simulink model "MATLAB_TEST"  (R2019b)
settings: Solver=FixedStepDiscrete  StartTime=0  StopTime=50  FixedStep=0.0025  RelTol=1e-3
undefined symbols (not defined in the file): BCM_COM_PROC_P20, BCM_COM_PROC_P20_SFW_R2018b, BCM_COM_PROC_P2_5, BCM_COM_PROC_P2_5_SFW_R2018b, BCM_COM_PROC_P5, BCM_COM_PROC_P5_SFW_R2018b, BCMA_ACCU_PT_Conf_Flt, BCMA_ACCU_PT_Unconf_Flt, BCMA_Antiskid_Off_Sanction, BCMA_Avionics_Conf_Flt, BCMA_BCM_CCDL_Conf_Flt, BCMA_BCM_CCDL_Unconf_Flt, BCMA_BCM_DBCU_INHIBITION_Conf_Flt, BCMA_BCM_DBCU_INHIBITION_Unconf_Flt, BCMA_BCP_ALT_Disp_Sw_Conf_Flt, BCMA_BCP_ALT_Disp_Sw_Unconf_Flt, BCMA_BCP_ALT_SW_ON_CMD_Conf_Flt, BCMA_BCP_ALT_SW_ON_CMD_Unconf_Flt, BCMA_BCP_PARK_OFF_SW_CMD_Conf_Flt, BCMA_BCP_PARK_OFF_SW_CMD_Unconf_Flt, BCMA_CF_BSELV_JCL, BCMA_CF_BSELV_JOP, BCMA_CF_BSELV_OC, BCMA_CF_BSELV_SC, BCMA_CF_LH_SV_JCL, BCMA_CF_LH_SV_JOP, BCMA_CF_LH_SV_OC, BCMA_CF_LH_SV_SC, BCMA_CF_PARK_BRK, BCMA_CF_RESIDUAL_PRESS, BCMA_CF_RH_SV_JCL, BCMA_CF_RH_SV_JOP, BCMA_CF_RH_SV_OC, BCMA_CF_RH_SV_SC, BCMA_CF_SELV_JCL, BCMA_CF_SELV_JOP, BCMA_CF_SELV_OC, BCMA_CF_SELV_SC, BCMA_CF_SV_DRIFT, BCMA_DBCU_ALT_MODE_Conf_Flt, BCMA_DBCU_ALT_MODE_Unconf_Flt, BCMA_DBCU_BRK_ORDER_FAIL_Conf_Flt, BCMA_DBCU_BRK_ORDER_FAIL_Unconf_Flt, BCMA_DBCU_Conf_Flt, BCMA_DBCU_DISPATCH_SW_ON_Conf_Flt, BCMA_DBCU_DISPATCH_SW_ON_Unconf_Flt, BCMA_DBCU_FAILED_Conf_Flt, BCMA_DBCU_FAILED_Unconf_Flt, BCMA_DFCS1_Capsule_Validity, BCMA_DFCS1_Label202_Corrupted, BCMA_DFCS1_Label202_Not_Refreshed, BCMA_DFCS1_Label204_Corrupted, BCMA_DFCS1_Label204_Not_Refreshed, BCMA_DFCS1_Label205_Corrupted, BCMA_DFCS1_Label205_Not_Refreshed, BCMA_DFCS1_Label206_Corrupted, BCMA_DFCS1_Label206_Not_Refreshed, BCMA_DFCS1_Label207_Corrupted, BCMA_DFCS1_Label207_Not_Refreshed, BCMA_DFCS3_Capsule_Validity ... (+762)
libraries: simulink x73, lib_MBD_Control x5
(part 10 of 16)

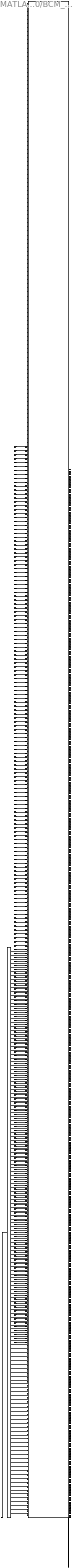
== system MATLAB_TEST/AVIONICS/Brake_Control_Module_Side_A/BCSA Controller CP/BCM_COM_PROC_P20/BCM_COM_PROC_P20 ==
  V_BCM_COM_Tacho_Conf_Flt_W12 : Inport
  V_BCM_COM_Tacho_Conf_Flt_W34 : Inport  Port=2
  V_BCM_COM_DFCS_A_Gnd_Spd_Acq : Inport  Port=3
  V_BCM_COM_DFCS_B_Gnd_Spd_Acq : Inport  Port=4
  V_BCM_COM_DFCS_A_Long_Accel_Acq : Inport  Port=5
  V_BCM_COM_DFCS_B_Long_Accel_Acq : Inport  Port=6
  V_BCM_COM_DFCS_A_Pitch_Ang_Acq : Inport  Port=7
  V_BCM_COM_DFCS_B_Pitch_Ang_Acq : Inport  Port=8
  V_BCM_COM_DFCS_A_LMLG_WOWs_Acq : Inport  Port=9
  V_BCM_COM_DFCS_B_LMLG_WOWs_Acq : Inport  Port=10
  V_BCM_COM_DFCS_A_RMLG_WOWs_Acq : Inport  Port=11
  V_BCM_COM_DFCS_B_RMLG_WOWs_Acq : Inport  Port=12
  V_BCM_COM_DFCS_A_NLG_WOWs_Acq : Inport  Port=13
  V_BCM_COM_DFCS_B_NLG_WOWs_Acq : Inport  Port=14
  V_BCM_COM_DFCS_A_WOWs_Val_Acq : Inport  Port=15
  V_BCM_COM_DFCS_B_WOWs_Val_Acq : Inport  Port=16
  V_BCM_COM_RH_Decel_Law_Brkg_Press_Cmd : Inport  Port=17
  V_BCM_COM_LH_Decel_Law_Brkg_Press_Cmd : Inport  Port=18
  V_BCM_COM_DFCS_A_DFCS_LH_Braking_Cmd_Acq : Inport  Port=19
  V_BCM_COM_DFCS_A_DFCS_RH_Braking_Cmd_Acq : Inport  Port=20
  V_BCM_COM_DFCS_B_DFCS_LH_Braking_Cmd_Acq : Inport  Port=21
  V_BCM_COM_DFCS_B_DFCS_RH_Braking_Cmd_Acq : Inport  Port=22
  V_BCM_COM_DFCS_A_Decel_Law_Inhib_Acq : Inport  Port=23
  V_BCM_COM_DFCS_B_Decel_Law_Inhib_Acq : Inport  Port=24
  V_BCM_COM_DFCS_A_TLA_Above_Idle_Acq : Inport  Port=25
  V_BCM_COM_DFCS_B_TLA_Above_Idle_Acq : Inport  Port=26
  V_BCM_COM_LG_Lever_Up_Acq : Inport  Port=27
  V_BCM_COM_LG_Lever_Up_Unconf_Flt : Inport  Port=28
  V_BCM_COM_LG_Lever_Up_Conf_Flt : Inport  Port=29
  V_BCM_COM_LMLG_Downlock_Acq : Inport  Port=30
  V_BCM_COM_RMLG_Downlock_Acq : Inport  Port=31
  V_BCM_COM_LMLG_Dnlk_Unconf_Flt : Inport  Port=32
  V_BCM_COM_LMLG_Dnlk_Conf_Flt : Inport  Port=33
  V_BCM_COM_RMLG_Dnlk_Unconf_Flt : Inport  Port=34
  V_BCM_COM_RMLG_Dnlk_Conf_Flt : Inport  Port=35
  V_BCM_COM_Engine_Running_Acq : Inport  Port=36
  V_BCM_COM_Maint_Itv_Function_Req : Inport  Port=37
  V_BCM_COM_BCM_Config : Inport  Port=38
  V_BCM_COM_BCM_Off_Sanction : Inport  Port=39
  V_BCM_COM_BCM_Validity_By_SP : Inport  Port=40
  V_BCM_COM_BCP_BCM_Alt_Sw_On_Cmd_Acq : Inport  Port=41
  V_BCM_COM_BCP_BCM_Alt_Sw_On_Cmd_Conf_Flt : Inport  Port=42
  V_BCM_COM_BCP_BCM_Alt_Sw_On_Cmd_Unconf_Flt : Inport  Port=43
  V_BCM_COM_MP_BCMA_Alt_Disp_Sw_Conf_Flt : Inport  Port=44
  V_BCM_COM_MP_BCMA_Alt_Disp_Sw_Unconf_Flt : Inport  Port=45
  V_BCM_COM_MP_BCMA_Alt_Disp_Sw_Acq : Inport  Port=46
  V_BCM_COM_Antiskid_Off_Sanction : Inport  Port=47
  V_BCM_COM_Norm_Brkg_Off_Sanc : Inport  Port=48
  V_BCM_COM_CF_LH_ALT_BRK_LOSS : Inport  Port=49
  V_BCM_COM_CF_DBCU_FAILED : Inport  Port=50
  V_BCM_COM_CF_RH_ALT_BRK_LOSS : Inport  Port=51
  V_BCM_COM_SV_PT_Filt : Inport  Port=52
  V_BCM_COM_PBSELV_ON_POS_Acq : Inport  Port=53
  V_BCM_COM_PBSELV_ON_POS_Unconf_Flt : Inport  Port=54
  V_BCM_COM_PBSELV_ON_POS_Conf_Flt : Inport  Port=55
  V_BCM_COM_Hyd_A_Press_Acq : Inport  Port=56
  V_BCM_COM_Hyd_B_Press_Acq : Inport  Port=57
  V_BCM_COM_Whl_AS_Inhib_Cond_W12 : Inport  Port=58
  V_BCM_COM_Whl_AS_Inhib_Cond_W34 : Inport  Port=59
  V_BCM_COM_Whl_LP_AS_Curr_Order : Inport  Port=60
  V_BCM_COM_SV_PT_Cons : Inport  Port=61
  V_BCM_COM_Wheel_Filtered_Speed_W12 : Inport  Port=62
  V_BCM_COM_Wheel_Filtered_Speed_W34 : Inport  Port=63
  V_BCM_COM_Wheel_Speed_Error_W12 : Inport  Port=64
  V_BCM_COM_Wheel_Speed_Error_W34 : Inport  Port=65
  V_BCM_COM_Whl_LP_AS_Curr_Order_W12 : Inport  Port=66
  V_BCM_COM_Whl_LP_AS_Curr_Order_W34 : Inport  Port=67
  V_BCM_COM_SV_Current : Inport  Port=68
  V_BCM_COM_SV_PT_Cons_Val : Inport  Port=69
  V_BCM_COM_BCM_CCDL_Conf_Flt : Inport  Port=70
  V_BCM_COM_BCM_CCDL_Unconf_Flt : Inport  Port=71
  V_BCM_COM_Adhesion_In_Acq_W12 : Inport  Port=72
  V_BCM_COM_Adhesion_In_Acq_W34 : Inport  Port=73
  V_BCM_COM_Opt_Adhesion_In_Acq_W12 : Inport  Port=74
  V_BCM_COM_Opt_Adhesion_In_Acq_W34 : Inport  Port=75
  V_BCM_COM_Target_Speed_In_Acq_W12 : Inport  Port=76
  V_BCM_COM_Target_Speed_In_Acq_W34 : Inport  Port=77
  V_BCM_COM_Big_Slip_WD_Trig_In_Acq_W12 : Inport  Port=78
  V_BCM_COM_Big_Slip_WD_Trig_In_Acq_W34 : Inport  Port=79
  V_BCM_COM_Big_Gamma_Trig_In_Acq_W12 : Inport  Port=80
  V_BCM_COM_Big_Gamma_Trig_In_Acq_W34 : Inport  Port=81
  V_BCM_COM_Small_Slip_Trig_In_Acq_W12 : Inport  Port=82
  V_BCM_COM_Small_Slip_Trig_In_Acq_W34 : Inport  Port=83
  V_BCM_COM_Big_Slip_Trig_In_Acq_W12 : Inport  Port=84
  V_BCM_COM_Big_Slip_Trig_In_Acq_W34 : Inport  Port=85
  V_BCM_COM_BCM_DBCU_INHIBITION_Conf_Flt : Inport  Port=86
  V_BCM_COM_BCM_DBCU_INHIBITION_Unconf_Flt : Inport  Port=87
  V_BCM_COM_BCM_DBCU_INHIBITION_Acq : Inport  Port=88
  V_BCM_COM_Engine_1_Running_Acq_Val : Inport  Port=89
  V_BCM_COM_Engine_2_Running_Acq_Val : Inport  Port=90
  V_BCM_COM_Hyd_A_Press_Acq_Val : Inport  Port=91
  V_BCM_COM_Hyd_B_Press_Acq_Val : Inport  Port=92
  V_BCM_COM_DFCS_A_Gnd_Spd_Acq_Val : Inport  Port=93
  V_BCM_COM_DFCS_A_Long_Accel_Acq_Val : Inport  Port=94
  V_BCM_COM_DFCS_A_Pitch_Angle_Acq_Val : Inport  Port=95
  V_BCM_COM_DFCS_A_Decel_Law_Inhib_Acq_Val : Inport  Port=96
  V_BCM_COM_DFCS_B_Decel_Law_Inhib_Acq_Val : Inport  Port=97
  V_BCM_COM_DFCS_B_Gnd_Spd_Acq_Val : Inport  Port=98
  V_BCM_COM_DFCS_B_Long_Accel_Acq_Val : Inport  Port=99
  V_BCM_COM_DFCS_B_Pitch_Angle_Acq_Val : Inport  Port=100
  V_BCM_COM_DFCS_A_Lmlg_Wow_1_Acq_Val : Inport  Port=101
  V_BCM_COM_DFCS_A_Lmlg_Wow_2_Acq_Val : Inport  Port=102
  V_BCM_COM_DFCS_A_Lmlg_Wow_3_Acq_Val : Inport  Port=103
  V_BCM_COM_DFCS_A_Rmlg_Wow_1_Acq_Val : Inport  Port=104
  V_BCM_COM_DFCS_A_Rmlg_Wow_2_Acq_Val : Inport  Port=105
  V_BCM_COM_DFCS_A_Rmlg_Wow_3_Acq_Val : Inport  Port=106
  V_BCM_COM_DFCS_A_Nlg_Wow_1_Acq_Val : Inport  Port=107
  V_BCM_COM_DFCS_A_Nlg_Wow_2_Acq_Val : Inport  Port=108
  V_BCM_COM_DFCS_A_Nlg_Wow_3_Acq_Val : Inport  Port=109
  V_BCM_COM_DFCS_A_Wow_Val_1_Acq_Val : Inport  Port=110
  V_BCM_COM_DFCS_A_Wow_Val_2_Acq_Val : Inport  Port=111
  V_BCM_COM_DFCS_A_Wow_Val_3_Acq_Val : Inport  Port=112
  V_BCM_COM_DFCS_B_Lmlg_Wow_1_Acq_Val : Inport  Port=113
  V_BCM_COM_DFCS_B_Lmlg_Wow_2_Acq_Val : Inport  Port=114
  V_BCM_COM_DFCS_B_Lmlg_Wow_3_Acq_Val : Inport  Port=115
  V_BCM_COM_DFCS_B_Rmlg_Wow_1_Acq_Val : Inport  Port=116
  V_BCM_COM_DFCS_B_Rmlg_Wow_2_Acq_Val : Inport  Port=117
  V_BCM_COM_DFCS_B_Rmlg_Wow_3_Acq_Val : Inport  Port=118
  V_BCM_COM_DFCS_B_Nlg_Wow_1_Acq_Val : Inport  Port=119
  V_BCM_COM_DFCS_B_Nlg_Wow_2_Acq_Val : Inport  Port=120
  V_BCM_COM_DFCS_B_Nlg_Wow_3_Acq_Val : Inport  Port=121
  V_BCM_COM_DFCS_B_Wow_Val_1_Acq_Val : Inport  Port=122
  V_BCM_COM_DFCS_B_Wow_Val_2_Acq_Val : Inport  Port=123
  V_BCM_COM_DFCS_B_Wow_Val_3_Acq_Val : Inport  Port=124
  V_BCM_COM_DFCS_B_DFCS_RH_Brkg_Cmd_Acq_Val : Inport  Port=125
  V_BCM_COM_DFCS_B_DFCS_LH_Brkg_Cmd_Acq_Val : Inport  Port=126
  V_BCM_COM_DFCS_A_DFCS_RH_Brkg_Cmd_Acq_Val : Inport  Port=127
  V_BCM_COM_DFCS_A_DFCS_LH_Brkg_Cmd_Acq_Val : Inport  Port=128
  V_BCM_COM_DFCS_A_DBCU_ALT_Mode_1_Acq_Val : Inport  Port=129
  V_BCM_COM_DFCS_A_DBCU_ALT_Mode_2_Acq_Val : Inport  Port=130
  V_BCM_COM_DFCS_B_DBCU_ALT_Mode_1_Acq_Val : Inport  Port=131
  V_BCM_COM_DFCS_B_DBCU_ALT_Mode_2_Acq_Val : Inport  Port=132
  V_BCM_COM_DFCS_A_TLA_Above_Idle_Acq_Val : Inport  Port=133
  V_BCM_COM_DFCS_B_TLA_Above_Idle_Acq_Val : Inport  Port=134
  V_BCM_COM_UTC_Time_Hours_Acq : Inport  Port=135
  V_BCM_COM_UTC_Time_Hours_Conf_Flt : Inport  Port=136
  V_BCM_COM_UTC_Time_Hours_Unconf_Flt : Inport  Port=137
  V_BCM_COM_UTC_Time_Minutes_Acq : Inport  Port=138
  V_BCM_COM_UTC_Time_Minutes_Conf_Flt : Inport  Port=139
  V_BCM_COM_UTC_Time_Minutes_Unconf_Flt : Inport  Port=140
  V_BCM_COM_UTC_Time_Seconds_Acq : Inport  Port=141
  V_BCM_COM_UTC_Time_Seconds_Conf_Flt : Inport  Port=142
  V_BCM_COM_UTC_Time_Seconds_Unconf_Flt : Inport  Port=143
  V_BCM_COM_DBCU_BRK_ORDER_FAIL_Acq : Inport  Port=144
  V_BCM_COM_DBCU_DISPATCH_SW_ON_Acq : Inport  Port=145
  V_BCM_COM_LH_DBCU_BRK_CMD_FDBK_Acq : Inport  Port=146
  V_BCM_COM_RH_DBCU_BRK_CMD_FDBK_Acq : Inport  Port=147
  V_BCM_COM_DBCU_FAILED_Acq : Inport  Port=148
  V_BCM_COM_DBCU_ALT_MODE_Acq : Inport  Port=149
  V_BCM_COM_DBCU_BRK_ORDER_FAIL_Conf_Flt : Inport  Port=150
  V_BCM_COM_DBCU_BRK_ORDER_FAIL_Unconf_Flt : Inport  Port=151
  V_BCM_COM_DBCU_DISPATCH_SW_ON_Conf_Flt : Inport  Port=152
  V_BCM_COM_DBCU_DISPATCH_SW_ON_Unconf_Flt : Inport  Port=153
  V_BCM_COM_LH_DBCU_BRK_CMD_FDBK_Conf_Flt : Inport  Port=154
  V_BCM_COM_LH_DBCU_BRK_CMD_FDBK_Unconf_Flt : Inport  Port=155
  V_BCM_COM_RH_DBCU_BRK_CMD_FDBK_Conf_Flt : Inport  Port=156
  V_BCM_COM_RH_DBCU_BRK_CMD_FDBK_Unconf_Flt : Inport  Port=157
  V_BCM_COM_DBCU_FAILED_Conf_Flt : Inport  Port=158
  V_BCM_COM_DBCU_FAILED_Unconf_Flt : Inport  Port=159
  V_BCM_COM_DBCU_ALT_MODE_Conf_Flt : Inport  Port=160
  V_BCM_COM_DBCU_ALT_MODE_Unconf_Flt : Inport  Port=161
  V_BCM_COM_ACCU_PT_Conf_Flt : Inport  Port=162
  V_BCM_COM_ACCU_PT_Unconf_Flt : Inport  Port=163
  V_BCM_COM_ACCU_PT_Acq : Inport  Port=164
  V_BCM_COM_LH_BTS_Conf_Flt : Inport  Port=165
  V_BCM_COM_LH_BTS_Unconf_Flt : Inport  Port=166
  V_BCM_COM_RH_BTS_Conf_Flt : Inport  Port=167
  V_BCM_COM_RH_BTS_Unconf_Flt : Inport  Port=168
  V_BCM_COM_BCP_PARK_OFF_SW_CMD_Acq : Inport  Port=169
  V_BCM_COM_BCP_PARK_OFF_SW_CMD_Conf_Flt : Inport  Port=170
  V_BCM_COM_BCP_PARK_OFF_SW_CMD_Unconf_Flt : Inport  Port=171
  V_BCM_COM_MP_MAINT_MODE_CMD_28V_Acq : Inport  Port=172
  V_BCM_COM_MP_MAINT_MODE_CMD_GND_Acq : Inport  Port=173
  V_BCM_COM_LNLG_Tire_Press_Acq : Inport  Port=174
  V_BCM_COM_LNLG_Tire_Press_Conf_Flt : Inport  Port=175
  V_BCM_COM_LNLG_Tire_Press_Unconf_Flt : Inport  Port=176
  V_BCM_COM_RNLG_Tire_Press_Acq : Inport  Port=177
  V_BCM_COM_RNLG_Tire_Press_Conf_Flt : Inport  Port=178
  V_BCM_COM_RNLG_Tire_Press_Unconf_Flt : Inport  Port=179
  V_BCM_COM_LMLG_Outboard_Tire_Press_Acq : Inport  Port=180
  V_BCM_COM_LMLG_Outboard_Tire_Press_Conf_Flt : Inport  Port=181
  V_BCM_COM_LMLG_Outboard_Tire_Press_Unconf_Flt : Inport  Port=182
  V_BCM_COM_LMLG_Inboard_Tire_Press_Acq : Inport  Port=183
  V_BCM_COM_LMLG_Inboard_Tire_Press_Conf_Flt : Inport  Port=184
  V_BCM_COM_LMLG_Inboard_Tire_Press_Unconf_Flt : Inport  Port=185
  V_BCM_COM_RMLG_Inboard_Tire_Press_Acq : Inport  Port=186
  V_BCM_COM_RMLG_Inboard_Tire_Press_Conf_Flt : Inport  Port=187
  V_BCM_COM_RMLG_Inboard_Tire_Press_Unconf_Flt : Inport  Port=188
  V_BCM_COM_RMLG_Outboard_Tire_Press_Acq : Inport  Port=189
  V_BCM_COM_RMLG_Outboard_Tire_Press_Conf_Flt : Inport  Port=190
  V_BCM_COM_RMLG_Outboard_Tire_Press_Unconf_Flt : Inport  Port=191
  V_BCM_COM_Whl_AS_Curr_Order : Inport  Port=192
  V_BCM_COM_SV_Current_Readback : Inport  Port=193
  V_BCM_COM_Whl_AS_Activity : Inport  Port=194
  V_BCM_COM_SELV_High_Side_Readback_Val : Inport  Port=195
  V_BCM_COM_SELV_High_Side_Readback : Inport  Port=196
  V_BCM_COM_CF_LH_SV_SC : Inport  Port=197
  V_BCM_COM_CF_LH_SV_OC : Inport  Port=198
  V_BCM_COM_CF_RH_SV_SC : Inport  Port=199
  V_BCM_COM_CF_RH_SV_OC : Inport  Port=200
  V_BCM_COM_CF_SELV_SC : Inport  Port=201
  V_BCM_COM_CF_SELV_OC : Inport  Port=202
  V_BCM_COM_CF_SELV_JOP : Inport  Port=203
  V_BCM_COM_CF_SELV_JCL : Inport  Port=204
  V_BCM_COM_CF_PARK_BRK : Inport  Port=205
  V_BCM_COM_CF_RESIDUAL_PRESS : Inport  Port=206
  V_BCM_COM_Avionics_Conf_Flt : Inport  Port=207
  V_BCM_COM_DFCS_A_Conf_Flt : Inport  Port=208
  V_BCM_COM_DFCS_A_DFCS_BCM_Caps_Val : Inport  Port=209
  V_BCM_COM_DFCS_B_Conf_Flt : Inport  Port=210
  V_BCM_COM_DFCS_B_DFCS_BCM_Caps_Val : Inport  Port=211
  V_BCM_COM_PPRG_i_Acquired : Inport  Port=212
  V_BCM_COM_PPRG_Fault : Inport  Port=213
  V_BCM_COM_DBCU_Conf_Flt : Inport  Port=214
  V_BCM_COM_SV_Current_Readback_Val : Inport  Port=215
  V_BCM_COM_SV_Current_Order : Inport  Port=216
  V_BCM_COM_CF_BSELV_OC : Inport  Port=217
  V_BCM_COM_CF_BSELV_SC : Inport  Port=218
  V_BCM_COM_CF_BSELV_JCL : Inport  Port=219
  V_BCM_COM_CF_BSELV_JOP : Inport  Port=220
  V_BCM_COM_LH_SV_PT_Conf_Flt : Inport  Port=221
  V_BCM_COM_CF_SV_DRIFT : Inport  Port=222
  V_BCM_COM_CF_LH_SV_JCL : Inport  Port=223
  V_BCM_COM_CF_LH_SV_JOP : Inport  Port=224
  V_BCM_COM_RH_SV_PT_Conf_Flt : Inport  Port=225
  V_BCM_COM_CF_RH_SV_JCL : Inport  Port=226
  V_BCM_COM_CF_RH_SV_JOP : Inport  Port=227
  V_BCM_COM_LH_BTS_TEMP_Comp : Inport  Port=228
  V_BCM_COM_RH_BTS_TEMP_Comp : Inport  Port=229
  BCM_Tuning : Inport  Port=230
  BCM_COM_PROC_P20 : S-Function  FunctionName=BCM_COM_PROC_P20_SFCT  SFunctionModules=<binary blob, 18839 chars, not shown>  SFunctionDeploymentMode=off  EnableBusSupport=off
  DTC{1..2,9..16,23..36,39..51,53..55,58..59,69..71,78..134,136..137,139..140,142..163,165..173,175..176,178..179,181..182,184..185,187..188,190..191,194..215,217..227} (182 alike) : DataTypeConversion  OutDataTypeStr=boolean  SaturateOnIntegerOverflow=on  RndMeth=Zero
  DTC{37..38,135,138,141} (5 alike) : DataTypeConversion  OutDataTypeStr=int32  SaturateOnIntegerOverflow=on  RndMeth=Zero
  DTC{3..8,17..22,52,56..57,60..68,72..77,164,174,177,180,183,186,189,192..193,216,228..229} (42 alike) : DataTypeConversion  OutDataTypeStr=single  SaturateOnIntegerOverflow=on  RndMeth=Zero
  PRB_BrakeFilled : Terminator
  PRB_BrakeFilled (1) : Terminator
  PRB_GroundStopFastCond : Terminator
  PRB_GroundStopSlowCond : Terminator
  PRB_RateLimitation : Terminator
  PRB_RateLimitation (1) : Terminator
  PRB_RateLimitationActivation : Terminator
  PRB_RateLimitationActivation (1) : Terminator
  Prb_Adhesion : Terminator
  Prb_Adhesion (1) : Terminator
  Prb_Adhesion (2) : Terminator
  Prb_Adhesion (3) : Terminator
  Prb_AdhesionOpt : Terminator
  Prb_AdhesionOpt (1) : Terminator
  Prb_AdhesionOpt (2) : Terminator
  Prb_AdhesionOpt (3) : Terminator
  Prb_AsBrkLossTargetDecel : Terminator
  Prb_AsBrkLossTargetDecel (1) : Terminator
  Prb_AsBrkLossTargetDecel (2) : Terminator
  Prb_AsBrkLossTargetDecel (3) : Terminator
  Prb_AsLowPassTheorCurrent : Terminator
  Prb_AsLowPassTheorCurrent (1) : Terminator
  Prb_AsLowPassTheorCurrent (2) : Terminator
  Prb_AsLowPassTheorCurrent (3) : Terminator
  Prb_AsLowPassTheorPressure : Terminator
  Prb_AsLowPassTheorPressure (1) : Terminator
  Prb_AsLowPassTheorPressure (2) : Terminator
  Prb_AsLowPassTheorPressure (3) : Terminator
  Prb_AutomateFilteredPressure : Terminator
  Prb_AutomateFilteredPressure (1) : Terminator
  Prb_AutomateFilteredPressure (2) : Terminator
  Prb_AutomateFilteredPressure (3) : Terminator
  Prb_AutomateSofteningFreezingCond : Terminator
  Prb_AutomateSofteningFreezingCond (1) : Terminator
  Prb_AutomateSofteningFreezingCond (2) : Terminator
  Prb_AutomateSofteningFreezingCond (3) : Terminator
  Prb_AutomateState : Terminator
  Prb_AutomateState (1) : Terminator
  Prb_AutomateState (2) : Terminator
  Prb_AutomateState (3) : Terminator
  Prb_BigGammaStepSize : Terminator
  Prb_BigGammaStepSize (1) : Terminator
  Prb_BigGammaStepSize (2) : Terminator
  Prb_BigGammaStepSize (3) : Terminator
  Prb_BigGammaThreshold : Terminator
  Prb_BigGammaThreshold (1) : Terminator
  Prb_BigGammaThreshold (2) : Terminator
  Prb_BigGammaThreshold (3) : Terminator
  Prb_BigSlipStepAuthorize : Terminator
  Prb_BigSlipStepAuthorize (1) : Terminator
  Prb_BigSlipStepAuthorize (2) : Terminator
  Prb_BigSlipStepAuthorize (3) : Terminator
  Prb_BigSlipWatchDogTargetDecel : Terminator
  Prb_BigSlipWatchDogTargetDecel (1) : Terminator
  Prb_BigSlipWatchDogTargetDecel (2) : Terminator
  Prb_BigSlipWatchDogTargetDecel (3) : Terminator
  Prb_BrakingPhaseAcceleration : Terminator
  Prb_BrakingPhaseAcceleration (1) : Terminator
  Prb_BrakingPhaseAcceleration (2) : Terminator
  Prb_BrakingPhaseAcceleration (3) : Terminator
  Prb_BrakingPhaseAcceleration (4) : Terminator
  Prb_CommandedPressureTheorCurrent : Terminator
  Prb_CommandedPressureTheorCurrent (1) : Terminator
  Prb_CommandedPressureTheorCurrent (2) : Terminator
  Prb_CommandedPressureTheorCurrent (3) : Terminator
  Prb_DecelerationDecrement : Terminator
  Prb_DecelerationDecrement (1) : Terminator
  Prb_DecelerationDecrement (2) : Terminator
  Prb_DecelerationDecrement (3) : Terminator
  Prb_DenAccuBigSlip : Terminator
  Prb_DenAccuBigSlip (1) : Terminator
  Prb_DenAccuBigSlip (2) : Terminator
  Prb_DenAccuBigSlip (3) : Terminator
  Prb_FastMonitoringCondition : Terminator
  Prb_FastMonitoringCondition (1) : Terminator
  Prb_FastMonitoringCondition (2) : Terminator
  Prb_FastMonitoringCondition (3) : Terminator
  Prb_FastStateCondition : Terminator
  Prb_FastStateCondition (1) : Terminator
  Prb_FastStateCondition (2) : Terminator
  Prb_FastStateCondition (3) : Terminator
  Prb_FastTrigCondition : Terminator
  Prb_FastTrigCondition (1) : Terminator
  Prb_FastTrigCondition (2) : Terminator
  Prb_FastTrigCondition (3) : Terminator
  Prb_ForcedBigGammaStep : Terminator
  Prb_ForcedBigGammaStep (1) : Terminator
  Prb_ForcedBigGammaStep (2) : Terminator
  Prb_ForcedBigGammaStep (3) : Terminator
  Prb_ForcedBigSlipStep : Terminator
  Prb_ForcedBigSlipStep (1) : Terminator
  Prb_ForcedBigSlipStep (2) : Terminator
  Prb_ForcedBigSlipStep (3) : Terminator
  Prb_ForcedBigSlipWatchDog : Terminator
  Prb_ForcedBigSlipWatchDog (1) : Terminator
  Prb_ForcedBigSlipWatchDog (2) : Terminator
  Prb_ForcedBigSlipWatchDog (3) : Terminator
  Prb_ForcedMonitoringAuthorized : Terminator
  Prb_ForcedMonitoringAuthorized (1) : Terminator
  Prb_ForcedMonitoringAuthorized (2) : Terminator
  Prb_ForcedMonitoringAuthorized (3) : Terminator
  Prb_ForcedSmallSlipStep : Terminator
  Prb_ForcedSmallSlipStep (1) : Terminator
  Prb_ForcedSmallSlipStep (2) : Terminator
  Prb_ForcedSmallSlipStep (3) : Terminator
  Prb_HydroplaneAccelCond : Terminator
  Prb_HydroplaneAccelCond (1) : Terminator
  Prb_HydroplaneAccelCond (2) : Terminator
  Prb_HydroplaneAccelCond (3) : Terminator
  Prb_HydroplaneAccelCond (4) : Terminator
  Prb_HydroplaneAccelProblem : Terminator
  Prb_HydroplaneAccelProblem (1) : Terminator
  Prb_HydroplaneAccelProblem (2) : Terminator
  Prb_HydroplaneAccelProblem (3) : Terminator
  Prb_HydroplaneAccelProblem (4) : Terminator
  Prb_HydroplaneAcceleration : Terminator
  Prb_HydroplaneAcceleration (1) : Terminator
  Prb_HydroplaneAcceleration (2) : Terminator
  Prb_HydroplaneAcceleration (3) : Terminator
  Prb_HydroplaneAcceleration (4) : Terminator
  Prb_HydroplaneCondition : Terminator
  Prb_HydroplaneCondition (1) : Terminator
  Prb_HydroplaneCondition (2) : Terminator
  Prb_HydroplaneCondition (3) : Terminator
  Prb_HydroplanePhaseInit : Terminator
  Prb_HydroplanePhaseInit (1) : Terminator
  Prb_HydroplanePhaseInit (2) : Terminator
  Prb_HydroplanePhaseInit (3) : Terminator
  Prb_HydroplanePhaseInit (4) : Terminator
  Prb_HydroplaneTransition : Terminator
  Prb_HydroplaneTransition (1) : Terminator
  Prb_HydroplaneTransition (2) : Terminator
  Prb_HydroplaneTransition (3) : Terminator
  Prb_HydroplaneTransition (4) : Terminator
  Prb_Hydroplane_PreviousSpeed : Terminator
  Prb_Hydroplane_PreviousSpeed (1) : Terminator
  Prb_Hydroplane_PreviousSpeed (2) : Terminator
  Prb_Hydroplane_PreviousSpeed (3) : Terminator
  Prb_LeftIsInvalid : Terminator
  Prb_LeftWheelSpeed : Terminator
  Prb_MinimalTargetDecel : Terminator
  Prb_MinimalTargetDecel (1) : Terminator
  Prb_MinimalTargetDecel (2) : Terminator
  Prb_MinimalTargetDecel (3) : Terminator
  Prb_NaturalBigGammaStep : Terminator
  Prb_NaturalBigGammaStep (1) : Terminator
  Prb_NaturalBigGammaStep (2) : Terminator
  Prb_NaturalBigGammaStep (3) : Terminator
  Prb_NaturalBigSlipStep : Terminator
  Prb_NaturalBigSlipStep (1) : Terminator
  Prb_NaturalBigSlipStep (2) : Terminator
  Prb_NaturalBigSlipStep (3) : Terminator
  Prb_NaturalBigSlipWatchDog : Terminator
  Prb_NaturalBigSlipWatchDog (1) : Terminator
  Prb_NaturalBigSlipWatchDog (2) : Terminator
  Prb_NaturalBigSlipWatchDog (3) : Terminator
  Prb_NaturalSmallSlipStep : Terminator
  Prb_NaturalSmallSlipStep (1) : Terminator
  Prb_NaturalSmallSlipStep (2) : Terminator
  Prb_NaturalSmallSlipStep (3) : Terminator
  Prb_OnGndAfterHydroAccel : Terminator
  Prb_OnGndAfterHydroAccel (1) : Terminator
  Prb_OnGndAfterHydroAccel (2) : Terminator
  Prb_OnGndAfterHydroAccel (3) : Terminator
  Prb_OnGndAfterHydroAccel (4) : Terminator
  Prb_OnGroundAfterHydroTransition : Terminator
  Prb_OnGroundAfterHydroTransition (1) : Terminator
  Prb_OnGroundAfterHydroTransition (2) : Terminator
  Prb_OnGroundAfterHydroTransition (3) : Terminator
  Prb_OnGroundAfterHydroplaneTransition : Terminator
  Prb_OptimalSpeed : Terminator
  Prb_OptimalSpeed (1) : Terminator
  Prb_OptimalSpeed (2) : Terminator
  Prb_OptimalSpeed (3) : Terminator
  Prb_PreviousSpeed : Terminator
  Prb_Previous_GlobalReferenceSpeed : Terminator
  Prb_Previous_ReferenceSpeed : Terminator
  Prb_Previous_ReferenceSpeed (1) : Terminator
  Prb_Previous_ReferenceSpeed (2) : Terminator
  Prb_Previous_ReferenceSpeed (3) : Terminator
  Prb_Previous_WheelSpeedState : Terminator
  Prb_Previous_WheelSpeedState (1) : Terminator
  Prb_Previous_WheelSpeedState (2) : Terminator
  Prb_Previous_WheelSpeedState (3) : Terminator
  Prb_Previous_WheelSpeedState (4) : Terminator
  Prb_RefSpeedLowLimit : Terminator
  Prb_RefSpeedLowLimit (1) : Terminator
  Prb_RefSpeedLowLimit (2) : Terminator
  Prb_RefSpeedLowLimit (3) : Terminator
  Prb_RefSpeedLowLimit (4) : Terminator
  Prb_RefSpeedLowLimit (5) : Terminator
  Prb_RefSpeedLowLimit (6) : Terminator
  Prb_RefSpeedLowLimit (7) : Terminator
  Prb_RefSpeedLowLimit (8) : Terminator
  Prb_ReferenceSpeedDelta : Terminator
  Prb_ReferenceSpeedDelta (1) : Terminator
  Prb_ReferenceSpeedDelta (2) : Terminator
  Prb_ReferenceSpeedDelta (3) : Terminator
  Prb_ResearchModeCondition : Terminator
  Prb_ResearchModeCondition (1) : Terminator
  Prb_ResearchModeCondition (2) : Terminator
  Prb_ResearchModeCondition (3) : Terminator
  Prb_RightIsInvalid : Terminator
  Prb_RightWheelSpeed : Terminator
  Prb_SelectedPressureOrder_i : Terminator
  Prb_SlowMonitoringCondition : Terminator
  Prb_SlowMonitoringCondition (1) : Terminator
  Prb_SlowMonitoringCondition (2) : Terminator
  Prb_SlowMonitoringCondition (3) : Terminator
  Prb_SlowStateCondition : Terminator
  Prb_SlowStateCondition (1) : Terminator
  Prb_SlowStateCondition (2) : Terminator
  Prb_SlowStateCondition (3) : Terminator
  Prb_SlowTrigCondition : Terminator
  Prb_SlowTrigCondition (1) : Terminator
  Prb_SlowTrigCondition (2) : Terminator
  Prb_SlowTrigCondition (3) : Terminator
  Prb_SoftSpeedCountOrder : Terminator
  Prb_SoftSpeedCountOrder (1) : Terminator
  Prb_SoftSpeedCountOrder (2) : Terminator
  Prb_SoftSpeedCountOrder (3) : Terminator
  Prb_SoftSpeedCounter : Terminator
  Prb_SoftSpeedCounter (1) : Terminator
  Prb_SoftSpeedCounter (2) : Terminator
  Prb_SoftSpeedCounter (3) : Terminator
  Prb_SoftSpeedMaximum : Terminator
  Prb_SoftSpeedMaximum (1) : Terminator
  Prb_SoftSpeedMaximum (2) : Terminator
  Prb_SoftSpeedMaximum (3) : Terminator
  Prb_SoftSpeedResetOrder : Terminator
  Prb_SoftSpeedResetOrder (1) : Terminator
  Prb_SoftSpeedResetOrder (2) : Terminator
  Prb_SoftSpeedResetOrder (3) : Terminator
  Prb_SofteningSpeed : Terminator
  Prb_SofteningSpeed (1) : Terminator
  Prb_SofteningSpeed (2) : Terminator
  Prb_SofteningSpeed (3) : Terminator
  Prb_SpunUpCondition : Terminator
  Prb_SpunUpCondition (1) : Terminator
  Prb_SpunUpCondition (2) : Terminator
  Prb_SpunUpCondition (3) : Terminator
  Prb_SpunUpCondition_i : Terminator
  Prb_SpunUpProtectedBrakingOrder : Terminator
  Prb_StateSignalValidityCondition : Terminator
  Prb_StateSignalValidityCondition (1) : Terminator
  Prb_StateSignalValidityCondition (2) : Terminator
  Prb_StateSignalValidityCondition (3) : Terminator
  Prb_StepSize : Terminator
  Prb_StepSize (1) : Terminator
  Prb_StepSize (2) : Terminator
  Prb_StepSize (3) : Terminator
  Prb_SvLowPassTheorCurrent : Terminator
  Prb_SvLowPassTheorCurrent (1) : Terminator
  Prb_SvLowPassTheorCurrent (2) : Terminator
  Prb_SvLowPassTheorCurrent (3) : Terminator
  Prb_TargetOverDecelInteg : Terminator
  Prb_TargetOverDecelInteg (1) : Terminator
  Prb_TargetOverDecelInteg (2) : Terminator
  Prb_TargetOverDecelInteg (3) : Terminator
  Prb_TargetSpeedDelta : Terminator
  Prb_TargetSpeedDelta (1) : Terminator
  Prb_TargetSpeedDelta (2) : Terminator
  Prb_TargetSpeedDelta (3) : Terminator
  Prb_TheorCommandedPressure : Terminator
  Prb_TheorCommandedPressure (1) : Terminator
  Prb_TheorCommandedPressure (2) : Terminator
  Prb_TheorCommandedPressure (3) : Terminator
  Prb_TransitionAntiskidBrakeLoss : Terminator
  Prb_TransitionAntiskidBrakeLoss (1) : Terminator
  Prb_TransitionAntiskidBrakeLoss (2) : Terminator
  Prb_TransitionAntiskidBrakeLoss (3) : Terminator
  Prb_TransitionBigGammaStep : Terminator
  Prb_TransitionBigGammaStep (1) : Terminator
  Prb_TransitionBigGammaStep (2) : Terminator
  Prb_TransitionBigGammaStep (3) : Terminator
  Prb_TransitionBigSlipStep : Terminator
  Prb_TransitionBigSlipStep (1) : Terminator
  Prb_TransitionBigSlipStep (2) : Terminator
  Prb_TransitionBigSlipStep (3) : Terminator
  Prb_TransitionBigSlipWatchDog : Terminator
  Prb_TransitionBigSlipWatchDog (1) : Terminator
  Prb_TransitionBigSlipWatchDog (2) : Terminator
  Prb_TransitionBigSlipWatchDog (3) : Terminator
  Prb_TransitionBrakingInit : Terminator
  Prb_TransitionBrakingInit (1) : Terminator
  Prb_TransitionBrakingInit (2) : Terminator
  Prb_TransitionBrakingInit (3) : Terminator
  Prb_TransitionGammaDecrease : Terminator
  Prb_TransitionGammaDecrease (1) : Terminator
  Prb_TransitionGammaDecrease (2) : Terminator
  Prb_TransitionGammaDecrease (3) : Terminator
  Prb_TransitionGammaIncrease : Terminator
  Prb_TransitionGammaIncrease (1) : Terminator
  Prb_TransitionGammaIncrease (2) : Terminator
  Prb_TransitionGammaIncrease (3) : Terminator
  Prb_TransitionSmallSlipStep : Terminator
  Prb_TransitionSmallSlipStep (1) : Terminator
  Prb_TransitionSmallSlipStep (2) : Terminator
  Prb_TransitionSmallSlipStep (3) : Terminator
  Prb_UncorrectedMinimaltargetDecel : Terminator
  Prb_UncorrectedMinimaltargetDecel (1) : Terminator
  Prb_UncorrectedMinimaltargetDecel (2) : Terminator
  Prb_UncorrectedMinimaltargetDecel (3) : Terminator
  Prb_UnlimitedReferenceSpeed_3 : Terminator
  Prb_UnlimitedReferenceSpeed_3 (1) : Terminator
  Prb_UnlimitedReferenceSpeed_3 (2) : Terminator
  Prb_UnlimitedReferenceSpeed_3 (3) : Terminator
  Prb_UnlimitedReferenceSpeed_4 : Terminator
  Prb_UnlimitedReferenceSpeed_4 (1) : Terminator
  Prb_UnlimitedReferenceSpeed_4 (2) : Terminator
  Prb_UnlimitedReferenceSpeed_4 (3) : Terminator
  Prb_WheelSkidSmoothAverage : Terminator
  Prb_WheelSkidSmoothAverage (1) : Terminator
  Prb_WheelSkidSmoothAverage (2) : Terminator
  Prb_WheelSkidSmoothAverage (3) : Terminator
  Prb_WheelSpeedState : Terminator
  Prb_WheelSpeedState (1) : Terminator
  Prb_WheelSpeedState (2) : Terminator
  Prb_WheelSpeedState (3) : Terminator
  Prb_WheelSpeedState (4) : Terminator
  Prb_WheelSpunUpCond : Terminator
  Subsystem : Subsystem
  v_BCM_COM_AC_Long_Accel_Filt : Terminator
  v_BCM_COM_ATB_in : Terminator
  v_BCM_COM_ATB_out : Terminator
  v_BCM_COM_All_Engines_Off : Terminator
  v_BCM_COM_Alt_FT_Reset_Cond : Terminator
  v_BCM_COM_Automate_On_W12 : Terminator
  v_BCM_COM_Automate_On_W34 : Terminator
  v_BCM_COM_Automate_WD_Frozen : Terminator
  v_BCM_COM_Braking_On_W12 : Terminator
  v_BCM_COM_Braking_On_W34 : Terminator
  v_BCM_COM_Braking_State_Norm : Terminator
  v_BCM_COM_Braking_Ste_Is_Normal : Terminator
  v_BCM_COM_Brkg_SELV_High_Side_FT_Cond : Terminator
  v_BCM_COM_CF_DFCS_A_ACCEL_RX : Terminator
  v_BCM_COM_CF_DFCS_A_DBCU_ALT_MODE_1_RX : Terminator
  v_BCM_COM_CF_DFCS_A_DBCU_ALT_MODE_2_RX : Terminator
  v_BCM_COM_CF_DFCS_A_DECEL_LAW_INHIB_RX : Terminator
  v_BCM_COM_CF_DFCS_A_GND_SPEED_RX : Terminator
  v_BCM_COM_CF_DFCS_A_LH_BRK_CMD_RX : Terminator
  v_BCM_COM_CF_DFCS_A_LMLGWOW_1_RX : Terminator
  v_BCM_COM_CF_DFCS_A_LMLGWOW_2_RX : Terminator
  v_BCM_COM_CF_DFCS_A_LMLGWOW_3_RX : Terminator
  v_BCM_COM_CF_DFCS_A_NLGWOW_1_RX : Terminator
  v_BCM_COM_CF_DFCS_A_NLGWOW_2_RX : Terminator
  v_BCM_COM_CF_DFCS_A_NLGWOW_3_RX : Terminator
  v_BCM_COM_CF_DFCS_A_PITCH_RX : Terminator
  v_BCM_COM_CF_DFCS_A_RH_BRK_CMD_RX : Terminator
  v_BCM_COM_CF_DFCS_A_RMLGWOW_1_RX : Terminator
  v_BCM_COM_CF_DFCS_A_RMLGWOW_2_RX : Terminator
  v_BCM_COM_CF_DFCS_A_RMLGWOW_3_RX : Terminator
  v_BCM_COM_CF_DFCS_A_TLA_ABOVE_IDLE_RX : Terminator
  v_BCM_COM_CF_DFCS_A_VALWOW_1_RX : Terminator
  v_BCM_COM_CF_DFCS_A_VALWOW_2_RX : Terminator
  v_BCM_COM_CF_DFCS_A_VALWOW_3_RX : Terminator
  v_BCM_COM_CF_DFCS_B_ACCEL_RX : Terminator
  v_BCM_COM_CF_DFCS_B_DBCU_ALT_MODE_1_RX : Terminator
  v_BCM_COM_CF_DFCS_B_DBCU_ALT_MODE_2_RX : Terminator
  v_BCM_COM_CF_DFCS_B_DECEL_LAW_INHIB_RX : Terminator
  v_BCM_COM_CF_DFCS_B_GND_SPEED_RX : Terminator
  v_BCM_COM_CF_DFCS_B_LH_BRK_CMD_RX : Terminator
  v_BCM_COM_CF_DFCS_B_LMLGWOW_1_RX : Terminator
  v_BCM_COM_CF_DFCS_B_LMLGWOW_2_RX : Terminator
  v_BCM_COM_CF_DFCS_B_LMLGWOW_3_RX : Terminator
  v_BCM_COM_CF_DFCS_B_NLGWOW_1_RX : Terminator
  v_BCM_COM_CF_DFCS_B_NLGWOW_2_RX : Terminator
  v_BCM_COM_CF_DFCS_B_NLGWOW_3_RX : Terminator
  v_BCM_COM_CF_DFCS_B_PITCH_RX : Terminator
  v_BCM_COM_CF_DFCS_B_RH_BRK_CMD_RX : Terminator
  v_BCM_COM_CF_DFCS_B_RMLGWOW_1_RX : Terminator
  v_BCM_COM_CF_DFCS_B_RMLGWOW_2_RX : Terminator
  v_BCM_COM_CF_DFCS_B_RMLGWOW_3_RX : Terminator
  v_BCM_COM_CF_DFCS_B_TLA_ABOVE_IDLE_RX : Terminator
  v_BCM_COM_CF_DFCS_B_VALWOW_1_RX : Terminator
  v_BCM_COM_CF_DFCS_B_VALWOW_2_RX : Terminator
  v_BCM_COM_CF_DFCS_B_VALWOW_3_RX : Terminator
  v_BCM_COM_CF_ENG_1_RUN_RX : Terminator
  v_BCM_COM_CF_ENG_2_RUN_RX : Terminator
  v_BCM_COM_CF_HYD_A_PRESS_RX : Terminator
  v_BCM_COM_CF_HYD_B_PRESS_RX : Terminator
  v_BCM_COM_Custom_Braking_Mode : Terminator
  v_BCM_COM_Custom_Brkg_Cmd : Terminator
  v_BCM_COM_ERU_in : Terminator
  v_BCM_COM_ERU_out : Terminator
  v_BCM_COM_FTB_in : Terminator
  v_BCM_COM_FTB_out : Terminator
  v_BCM_COM_Forced_Act_SELV : Terminator
  v_BCM_COM_Func_Test_Press_Cmd : Terminator
  v_BCM_COM_Hyd_Press_State : Terminator
  v_BCM_COM_LGRB_in : Terminator
  v_BCM_COM_LGRB_out : Terminator
  v_BCM_COM_MLG_Dnlk_State_Cons : Terminator
  v_BCM_COM_MLG_Downlock_State_Cond : Terminator
  v_BCM_COM_MTB_in : Terminator
  v_BCM_COM_MTB_out : Terminator
  v_BCM_COM_Norm_FT_Reset_Cond : Terminator
  v_BCM_COM_PB_in : Terminator
  v_BCM_COM_PB_out : Terminator
  v_BCM_COM_Press_Cmd_FT : Terminator
  v_BCM_COM_Press_Rate_Lim_Inhib_Cond : Terminator
  v_BCM_COM_Rate_Lim_Law : Terminator
  v_BCM_COM_Regular_Brkg_Press_Cmd : Terminator
  v_BCM_COM_Ret_Brkg_Press_Cmd : Terminator
  v_BCM_COM_SELV_FT : Terminator
  v_BCM_COM_SELV_High_Side_Cmd_Order_Prev : Terminator
  v_BCM_COM_Spun_Up_Condition_W12 : Terminator
  v_BCM_COM_Spun_Up_Condition_W34 : Terminator
  v_BCM_COM_Takeoff_Phase : Terminator
  v_BCM_COM_Touchdown_Not_Active : Terminator
  v_BCM_COM_UF_DFCS_A_ACCEL_RX : Terminator
  v_BCM_COM_UF_DFCS_A_DBCU_ALT_MODE_1_RX : Terminator
  v_BCM_COM_UF_DFCS_A_DBCU_ALT_MODE_2_RX : Terminator
  v_BCM_COM_UF_DFCS_A_DECEL_LAW_INHIB_RX : Terminator
  v_BCM_COM_UF_DFCS_A_GND_SPEED_RX : Terminator
  v_BCM_COM_UF_DFCS_A_LH_BRK_CMD_RX : Terminator
  v_BCM_COM_UF_DFCS_A_LMLGWOW_1_RX : Terminator
  v_BCM_COM_UF_DFCS_A_LMLGWOW_2_RX : Terminator
  v_BCM_COM_UF_DFCS_A_LMLGWOW_3_RX : Terminator
  v_BCM_COM_UF_DFCS_A_NLGWOW_1_RX : Terminator
  v_BCM_COM_UF_DFCS_A_NLGWOW_2_RX : Terminator
  v_BCM_COM_UF_DFCS_A_NLGWOW_3_RX : Terminator
  v_BCM_COM_UF_DFCS_A_PITCH_RX : Terminator
  v_BCM_COM_UF_DFCS_A_RH_BRK_CMD_RX : Terminator
  v_BCM_COM_UF_DFCS_A_RMLGWOW_1_RX : Terminator
  v_BCM_COM_UF_DFCS_A_RMLGWOW_2_RX : Terminator
  v_BCM_COM_UF_DFCS_A_RMLGWOW_3_RX : Terminator
  v_BCM_COM_UF_DFCS_A_TLA_ABOVE_IDLE_RX : Terminator
  v_BCM_COM_UF_DFCS_A_VALWOW_1_RX : Terminator
  v_BCM_COM_UF_DFCS_A_VALWOW_2_RX : Terminator
  v_BCM_COM_UF_DFCS_A_VALWOW_3_RX : Terminator
  v_BCM_COM_UF_DFCS_B_ACCEL_RX : Terminator
  v_BCM_COM_UF_DFCS_B_DBCU_ALT_MODE_1_RX : Terminator
  v_BCM_COM_UF_DFCS_B_DBCU_ALT_MODE_2_RX : Terminator
  v_BCM_COM_UF_DFCS_B_DECEL_LAW_INHIB_RX : Terminator
  v_BCM_COM_UF_DFCS_B_GND_SPEED_RX : Terminator
  v_BCM_COM_UF_DFCS_B_LH_BRK_CMD_RX : Terminator
  v_BCM_COM_UF_DFCS_B_LMLGWOW_1_RX : Terminator
  v_BCM_COM_UF_DFCS_B_LMLGWOW_2_RX : Terminator
  v_BCM_COM_UF_DFCS_B_LMLGWOW_3_RX : Terminator
  v_BCM_COM_UF_DFCS_B_NLGWOW_1_RX : Terminator
  v_BCM_COM_UF_DFCS_B_NLGWOW_2_RX : Terminator
  v_BCM_COM_UF_DFCS_B_NLGWOW_3_RX : Terminator
  v_BCM_COM_UF_DFCS_B_PITCH_RX : Terminator
  v_BCM_COM_UF_DFCS_B_RH_BRK_CMD_RX : Terminator
  v_BCM_COM_UF_DFCS_B_RMLGWOW_1_RX : Terminator
  v_BCM_COM_UF_DFCS_B_RMLGWOW_2_RX : Terminator
  v_BCM_COM_UF_DFCS_B_RMLGWOW_3_RX : Terminator
  v_BCM_COM_UF_DFCS_B_TLA_ABOVE_IDLE_RX : Terminator
  v_BCM_COM_UF_DFCS_B_VALWOW_1_RX : Terminator
  v_BCM_COM_UF_DFCS_B_VALWOW_2_RX : Terminator
  v_BCM_COM_UF_DFCS_B_VALWOW_3_RX : Terminator
  v_BCM_COM_UF_ENG_1_RUN_RX : Terminator
  v_BCM_COM_UF_ENG_2_RUN_RX : Terminator
  v_BCM_COM_UF_HYD_A_PRESS_RX : Terminator
  v_BCM_COM_UF_HYD_B_PRESS_RX : Terminator
  V_BCM_COM_Whl_Spun_Up_State_W12 : Outport
  V_BCM_COM_Whl_Ref_Speed_W12 : Outport  Port=2
  V_BCM_COM_Whl_Spun_Up_State_W34 : Outport  Port=3
  V_BCM_COM_Whl_Ref_Speed_W34 : Outport  Port=4
  V_BCM_COM_DFCS_A_Gnd_Spd_Conv : Outport  Port=5
  V_BCM_COM_DFCS_B_Gnd_Spd_Conv : Outport  Port=6
  V_BCM_COM_AC_Gnd_Spd_Cons : Outport  Port=7
  V_BCM_COM_AC_Gnd_Spd_Cons_Val : Outport  Port=8
  V_BCM_COM_DFCS_A_Long_Accel_Conv : Outport  Port=9
  V_BCM_COM_DFCS_B_Long_Accel_Conv : Outport  Port=10
  V_BCM_COM_AC_Long_Accel_Cons : Outport  Port=11
  V_BCM_COM_AC_Long_Accel_Cons_Val : Outport  Port=12
  V_BCM_COM_AC_Long_Accel_Filt_Corr : Outport  Port=13
  V_BCM_COM_AC_Pitch_Ang_Cons_Val : Outport  Port=14
  V_BCM_COM_AC_Pitch_Ang_Filt : Outport  Port=15
  V_BCM_COM_AC_Pitch_Ang_Cons : Outport  Port=16
  V_BCM_COM_DFCS_A_WOWs_Val_Cons : Outport  Port=17
  V_BCM_COM_DFCS_B_WOWs_Val_Cons : Outport  Port=18
  V_BCM_COM_LMLG_WOWs_Cons : Outport  Port=19
  V_BCM_COM_LMLG_WOWs_Cons_Val : Outport  Port=20
  V_BCM_COM_RMLG_WOWs_Cons : Outport  Port=21
  V_BCM_COM_RMLG_WOWs_Cons_Val : Outport  Port=22
  V_BCM_COM_NLG_WOWs_Cons : Outport  Port=23
  V_BCM_COM_NLG_WOWs_Cons_Val : Outport  Port=24
  V_BCM_COM_LMLG_On_Gnd_State : Outport  Port=25
  V_BCM_COM_RMLG_On_Gnd_State : Outport  Port=26
  V_BCM_COM_LMLG_On_Gnd_State_Val : Outport  Port=27
  V_BCM_COM_RMLG_On_Gnd_State_Val : Outport  Port=28
  V_BCM_COM_MLG_On_Gnd_State : Outport  Port=29
  V_BCM_COM_NLG_On_Gnd_State : Outport  Port=30
  V_BCM_COM_NLG_On_Gnd_State_Val : Outport  Port=31
  V_BCM_COM_NLG_On_Gnd_State_Cons : Outport  Port=32
  V_BCM_COM_LH_Braking_Cmd_Cons : Outport  Port=33
  V_BCM_COM_RH_Braking_Cmd_Cons : Outport  Port=34
  V_BCM_COM_Decel_Law_Inhib_Cons : Outport  Port=35
  V_BCM_COM_Decel_Law_Inhib_Cons_Val : Outport  Port=36
  V_BCM_COM_TLA_State_Cons : Outport  Port=37
  V_BCM_COM_TLA_State_Cons_Val : Outport  Port=38
  V_BCM_COM_LG_Lever_Up_Conf : Outport  Port=39
  V_BCM_COM_LG_Lever_State_Cons : Outport  Port=40
  V_BCM_COM_LG_Lever_Ste_Cons_Val : Outport  Port=41
  V_BCM_COM_LMLG_Downlock_Conf : Outport  Port=42
  V_BCM_COM_RMLG_Downlock_Conf : Outport  Port=43
  V_BCM_COM_LMLG_Downlock_State : Outport  Port=44
  V_BCM_COM_LMLG_Dnlk_State_Val : Outport  Port=45
  V_BCM_COM_RMLG_Downlock_State : Outport  Port=46
  V_BCM_COM_RMLG_Dnlk_State_Val : Outport  Port=47
  V_BCM_COM_SELV_High_Side_Cmd_Order : Outport  Port=48
  V_BCM_COM_SELV_Low_Speed_Logic : Outport  Port=49
  V_BCM_COM_Engine_State : Outport  Port=50
  V_BCM_COM_Engine_State_Val : Outport  Port=51
  V_BCM_COM_LH_Braking_Cmd_State : Outport  Port=52
  V_BCM_COM_RH_Braking_Cmd_State : Outport  Port=53
  V_BCM_COM_LH_Regular_Brkg_Press_Cmd : Outport  Port=54
  V_BCM_COM_RH_Regular_Brkg_Press_Cmd : Outport  Port=55
  V_BCM_COM_Wheels_Global_Spun_Up_Ste : Outport  Port=56
  V_BCM_COM_Global_Reference_Spd : Outport  Port=57
  V_BCM_COM_Global_Wheel_Spd : Outport  Port=58
  V_BCM_COM_LMLG_Global_Wheel_Spd : Outport  Port=59
  V_BCM_COM_RMLG_Global_Wheel_Spd : Outport  Port=60
  V_BCM_COM_AC_State : Outport  Port=61
  V_BCM_COM_AC_Flight_Phase : Outport  Port=62
  V_BCM_COM_Braking_Mode : Outport  Port=63
  v_BCM_COM_FT_Seq : Outport  Port=64
  V_BCM_COM_Start_Norm_FT_Cond : Outport  Port=65
  V_BCM_COM_Brkg_Norm_FT_Prog_Sts : Outport  Port=66
  V_BCM_COM_Brkg_Norm_FT_Cond : Outport  Port=67
  V_BCM_COM_Braking_Norm_FT_Seq : Outport  Port=68
  V_BCM_COM_Abort_Norm_FT_Cond : Outport  Port=69
  V_BCM_COM_Brkg_Alt_FT_Prog_Sts : Outport  Port=70
  V_BCM_COM_Braking_Alt_FT_Seq : Outport  Port=71
  V_BCM_COM_Abort_Alt_FT_Cond : Outport  Port=72
  V_BCM_COM_Start_Alt_FT_Cond : Outport  Port=73
  V_BCM_COM_Brkg_Alt_FT_Cond : Outport  Port=74
  V_BCM_COM_LH_Press_Reg_FT_Act_Cond : Outport  Port=75
  V_BCM_COM_RH_Press_Reg_FT_Act_Cond : Outport  Port=76
  V_BCM_COM_LH_Press_Law_Brkg_Press_Cmd : Outport  Port=77
  V_BCM_COM_RH_Press_Law_Brkg_Press_Cmd : Outport  Port=78
  V_BCM_COM_LH_FT_Press_Cmd : Outport  Port=79
  V_BCM_COM_RH_FT_Press_Cmd : Outport  Port=80
  V_BCM_COM_LH_Ret_Brkg_Press_Cmd : Outport  Port=81
  V_BCM_COM_RH_Ret_Brkg_Press_Cmd : Outport  Port=82
  V_BCM_COM_LH_Eng_Run_Press_Cmd : Outport  Port=83
  V_BCM_COM_RH_Eng_Run_Press_Cmd : Outport  Port=84
  V_BCM_COM_Brkg_SELV_High_Side_FT_Cmd_Order : Outport  Port=85
  V_BCM_COM_DBCU_FT_Inhib_Order : Outport  Port=86
  V_BCM_COM_DBCU_Inhib_Order : Outport  Port=87
  V_BCM_COM_BCM_Validity : Outport  Port=88
  V_BCM_COM_Alt_Sw_Cmd_Cons : Outport  Port=89
  V_BCM_COM_Alt_Sw_Cmd_Cons_Val : Outport  Port=90
  V_BCM_COM_Disp_Sw_Cmd_Cons : Outport  Port=91
  V_BCM_COM_Disp_Sw_Cmd_Cons_Val : Outport  Port=92
  V_BCM_COM_MP_BCMA_Alt_Disp_Sw_Conf : Outport  Port=93
  V_BCM_COM_BCP_BCM_Alt_Sw_On_Cmd_Conf : Outport  Port=94
  V_BCM_COM_Braking_State : Outport  Port=95
  V_BCM_COM_Norm_Brkg_Availability : Outport  Port=96
  V_BCM_COM_Alt_Brkg_Availability : Outport  Port=97
  V_BCM_COM_Braking_Type : Outport  Port=98
  V_BCM_COM_Press_Cmd : Outport  Port=99
  V_BCM_COM_Brkg_On_Wheels : Outport  Port=100
  V_BCM_COM_Press_Cmd_Rate_Lim : Outport  Port=101
  V_BCM_COM_PBSELV_ON_POS_Conf : Outport  Port=102
  V_BCM_COM_PBSELV_State_Cons : Outport  Port=103
  V_BCM_COM_PBSELV_State_Cons_Val : Outport  Port=104
  V_BCM_COM_Hyd_A_Press_Cons : Outport  Port=105
  V_BCM_COM_Hyd_B_Press_Cons : Outport  Port=106
  V_BCM_COM_Hyd_A_Press_Cons_Val : Outport  Port=107
  V_BCM_COM_Hyd_B_Press_Cons_Val : Outport  Port=108
  V_BCM_COM_Hyd_A_Press_State : Outport  Port=109
  V_BCM_COM_Hyd_B_Press_State : Outport  Port=110
  V_BCM_COM_Sys_Sanc_Inhib_During_FT : Outport  Port=111
  V_BCM_COM_Wheel_Control_Speed_W12 : Outport  Port=112
  V_BCM_COM_Wheel_Control_Speed_W34 : Outport  Port=113
  V_BCM_COM_Big_Gamma_Trig_Out_W12 : Outport  Port=114
  V_BCM_COM_Big_Gamma_Trig_Out_W34 : Outport  Port=115
  V_BCM_COM_Big_Slip_Trig_Out_W12 : Outport  Port=116
  V_BCM_COM_Big_Slip_Trig_Out_W34 : Outport  Port=117
  V_BCM_COM_Big_Slip_WD_Trig_Out_W12 : Outport  Port=118
  V_BCM_COM_Big_Slip_WD_Trig_Out_W34 : Outport  Port=119
  V_BCM_COM_Small_Slip_Trig_Out_W12 : Outport  Port=120
  V_BCM_COM_Small_Slip_Trig_Out_W34 : Outport  Port=121
  V_BCM_COM_Automate_State_W12 : Outport  Port=122
  V_BCM_COM_Automate_State_W34 : Outport  Port=123
  V_BCM_COM_Target_Speed_Out_W12 : Outport  Port=124
  V_BCM_COM_Target_Speed_Out_W34 : Outport  Port=125
  V_BCM_COM_Target_Decel_Out_W12 : Outport  Port=126
  V_BCM_COM_Target_Decel_Out_W34 : Outport  Port=127
  V_BCM_COM_Adhesion_Out_W12 : Outport  Port=128
  V_BCM_COM_Adhesion_Out_W34 : Outport  Port=129
  V_BCM_COM_Opt_Adhesion_Out_W12 : Outport  Port=130
  V_BCM_COM_Opt_Adhesion_Out_W34 : Outport  Port=131
  V_BCM_COM_Whl_AS_Adp_Gain_W12 : Outport  Port=132
  V_BCM_COM_Whl_AS_Adp_Gain_W34 : Outport  Port=133
  V_BCM_COM_Adhesion_In_Cons_W12 : Outport  Port=134
  V_BCM_COM_Adhesion_In_Cons_W34 : Outport  Port=135
  V_BCM_COM_Opt_Adhesion_In_Cons_W12 : Outport  Port=136
  V_BCM_COM_Opt_Adhesion_In_Cons_W34 : Outport  Port=137
  V_BCM_COM_Target_Speed_In_Cons_W12 : Outport  Port=138
  V_BCM_COM_Target_Speed_In_Cons_W34 : Outport  Port=139
  V_BCM_COM_Big_Slip_WD_Trig_In_Cons_W12 : Outport  Port=140
  V_BCM_COM_Big_Slip_WD_Trig_In_Cons_W34 : Outport  Port=141
  V_BCM_COM_Big_Gamma_Trig_In_Cons_W12 : Outport  Port=142
  V_BCM_COM_Big_Gamma_Trig_In_Cons_W34 : Outport  Port=143
  V_BCM_COM_Small_Slip_Trig_In_Cons_W12 : Outport  Port=144
  V_BCM_COM_Small_Slip_Trig_In_Cons_W34 : Outport  Port=145
  V_BCM_COM_Big_Slip_Trig_In_Cons_W12 : Outport  Port=146
  V_BCM_COM_Big_Slip_Trig_In_Cons_W34 : Outport  Port=147
  V_BCM_COM_CCDL_Data_From_Opp_BCM_Val : Outport  Port=148
  V_BCM_COM_DBCU_Inhibition_Order_From_Opp_BCM_Cons : Outport  Port=149
  V_BCM_COM_DBCU_Inhibition_Order_From_Opp_BCM_Cons_Val : Outport  Port=150
  V_BCM_COM_Engine_Running_Conf_Flt : Outport  Port=151
  V_BCM_COM_Engine_Running_Unconf_Flt : Outport  Port=152
  V_BCM_COM_Hyd_A_Press_Conf_Flt : Outport  Port=153
  V_BCM_COM_Hyd_B_Press_Conf_Flt : Outport  Port=154
  V_BCM_COM_Hyd_A_Press_Unconf_Flt : Outport  Port=155
  V_BCM_COM_Hyd_B_Press_Unconf_Flt : Outport  Port=156
  V_BCM_COM_DFCS_A_AC_Gnd_Spd_Val : Outport  Port=157
  V_BCM_COM_DFCS_A_AC_Long_Accel_Val : Outport  Port=158
  V_BCM_COM_DFCS_A_AC_Pitch_Angle_Val : Outport  Port=159
  V_BCM_COM_DFCS_A_Decel_Law_Inhib_Val : Outport  Port=160
  V_BCM_COM_DFCS_B_Decel_Law_Inhib_Val : Outport  Port=161
  V_BCM_COM_DFCS_B_AC_Gnd_Spd_Val : Outport  Port=162
  V_BCM_COM_DFCS_B_AC_Long_Accel_Val : Outport  Port=163
  V_BCM_COM_DFCS_B_AC_Pitch_Angle_Val : Outport  Port=164
  V_BCM_COM_DFCS_A_LMLG_WOWs_Val : Outport  Port=165
  V_BCM_COM_DFCS_A_RMLG_WOWs_Val : Outport  Port=166
  V_BCM_COM_DFCS_A_NLG_WOWs_Val : Outport  Port=167
  V_BCM_COM_DFCS_A_WOWs_Val_Val : Outport  Port=168
  V_BCM_COM_DFCS_B_LMLG_WOWs_Val : Outport  Port=169
  V_BCM_COM_DFCS_B_RMLG_WOWs_Val : Outport  Port=170
  V_BCM_COM_DFCS_B_NLG_WOWs_Val : Outport  Port=171
  V_BCM_COM_DFCS_B_WOWs_Val_Val : Outport  Port=172
  V_BCM_COM_DFCS_A_LH_Braking_Cmd_Val : Outport  Port=173
  V_BCM_COM_DFCS_A_RH_Braking_Cmd_Val : Outport  Port=174
  V_BCM_COM_DFCS_B_LH_Braking_Cmd_Val : Outport  Port=175
  V_BCM_COM_DFCS_B_RH_Braking_Cmd_Val : Outport  Port=176
  V_BCM_COM_DFCS_A_DBCU_Alt_Mode_1_Val : Outport  Port=177
  V_BCM_COM_DFCS_A_DBCU_Alt_Mode_2_Val : Outport  Port=178
  V_BCM_COM_DFCS_B_DBCU_Alt_Mode_1_Val : Outport  Port=179
  V_BCM_COM_DFCS_B_DBCU_Alt_Mode_2_Val : Outport  Port=180
  V_BCM_COM_DFCS_A_TLA_Above_Idle_Val : Outport  Port=181
  V_BCM_COM_DFCS_B_TLA_Above_Idle_Val : Outport  Port=182
  V_BCM_COM_UTC_Time_Hours_Cons : Outport  Port=183
  V_BCM_COM_UTC_Time_Hours_Cons_Val : Outport  Port=184
  V_BCM_COM_UTC_Time_Minutes_Cons : Outport  Port=185
  V_BCM_COM_UTC_Time_Minutes_Cons_Val : Outport  Port=186
  V_BCM_COM_UTC_Time_Seconds_Cons : Outport  Port=187
  V_BCM_COM_UTC_Time_Seconds_Cons_Val : Outport  Port=188
  V_BCM_COM_DBCU_BRK_ORDER_FAIL_Conf : Outport  Port=189
  V_BCM_COM_DBCU_DISPATCH_SW_ON_Conf : Outport  Port=190
  V_BCM_COM_LH_DBCU_BRK_CMD_FDBK_Conf : Outport  Port=191
  V_BCM_COM_RH_DBCU_BRK_CMD_FDBK_Conf : Outport  Port=192
  V_BCM_COM_DBCU_FAILED_Conf : Outport  Port=193
  V_BCM_COM_DBCU_ALT_MODE_Conf : Outport  Port=194
  V_BCM_COM_DBCU_BRK_ORDER_FAIL_Cons : Outport  Port=195
  V_BCM_COM_DBCU_BRK_ORDER_FAIL_Cons_Val : Outport  Port=196
  V_BCM_COM_DBCU_DISPATCH_SW_ON_Cons : Outport  Port=197
  V_BCM_COM_DBCU_DISPATCH_SW_ON_Cons_Val : Outport  Port=198
  V_BCM_COM_LH_DBCU_BRK_CMD_FDBK_Cons : Outport  Port=199
  V_BCM_COM_LH_DBCU_BRK_CMD_FDBK_Cons_Val : Outport  Port=200
  V_BCM_COM_RH_DBCU_BRK_CMD_FDBK_Cons : Outport  Port=201
  V_BCM_COM_RH_DBCU_BRK_CMD_FDBK_Cons_Val : Outport  Port=202
  V_BCM_COM_DBCU_FAILED_Cons : Outport  Port=203
  V_BCM_COM_DBCU_FAILED_Cons_Val : Outport  Port=204
  V_BCM_COM_DBCU_ALT_MODE_Cons : Outport  Port=205
  V_BCM_COM_DBCU_ALT_MODE_Cons_Val : Outport  Port=206
  V_BCM_COM_ACCU_PT_Cons : Outport  Port=207
  V_BCM_COM_ACCU_PT_Cons_Val : Outport  Port=208
  V_BCM_COM_ACCU_Pressure_State : Outport  Port=209
  V_BCM_COM_LH_Brake_Temp_Cons : Outport  Port=210
  V_BCM_COM_LH_Brake_Temp_Cons_Val : Outport  Port=211
  V_BCM_COM_RH_Brake_Temp_Cons : Outport  Port=212
  V_BCM_COM_RH_Brake_Temp_Cons_Val : Outport  Port=213
  V_BCM_COM_BCP_PARK_OFF_SW_CMD_Conf : Outport  Port=214
  V_BCM_COM_Park_Sw_Cmd_Cons : Outport  Port=215
  V_BCM_COM_Park_Sw_Cmd_Cons_Val : Outport  Port=216
  V_BCM_COM_MP_MAINT_MODE_CMD_28V_Conf : Outport  Port=217
  V_BCM_COM_MP_MAINT_MODE_CMD_GND_Conf : Outport  Port=218
  V_BCM_COM_Maint_Mode_State_Cons : Outport  Port=219
  V_BCM_COM_LNLG_Tire_Press_Cons : Outport  Port=220
  V_BCM_COM_RNLG_Tire_Press_Cons : Outport  Port=221
  V_BCM_COM_LNLG_Tire_Press_Cons_Val : Outport  Port=222
  V_BCM_COM_RNLG_Tire_Press_Cons_Val : Outport  Port=223
  V_BCM_COM_LMLG_Outboard_Tire_Press_Cons : Outport  Port=224
  V_BCM_COM_LMLG_Outboard_Tire_Press_Cons_Val : Outport  Port=225
  V_BCM_COM_LMLG_Inboard_Tire_Press_Cons : Outport  Port=226
  V_BCM_COM_LMLG_Inboard_Tire_Press_Cons_Val : Outport  Port=227
  V_BCM_COM_RMLG_Inboard_Tire_Press_Cons : Outport  Port=228
  V_BCM_COM_RMLG_Inboard_Tire_Press_Cons_Val : Outport  Port=229
  V_BCM_COM_RMLG_Outboard_Tire_Press_Cons : Outport  Port=230
  V_BCM_COM_RMLG_Outboard_Tire_Press_Cons_Val : Outport  Port=231
  V_BCM_COM_A429_SSM_Avionics_Label_005 : Outport  Port=232
  V_BCM_COM_A429_SSM_Avionics_Label_006 : Outport  Port=233
  V_BCM_COM_A429_SSM_Avionics_Label_021 : Outport  Port=234
  V_BCM_COM_A429_SSM_Avionics_Label_022 : Outport  Port=235
  V_BCM_COM_A429_SSM_Avionics_Label_030 : Outport  Port=236
  V_BCM_COM_A429_SSM_Avionics_Label_031 : Outport  Port=237
  V_BCM_COM_A429_SSM_Avionics_Label_032 : Outport  Port=238
  V_BCM_COM_A429_SSM_Avionics_Label_033 : Outport  Port=239
  V_BCM_COM_A429_SSM_Avionics_Label_040 : Outport  Port=240
  V_BCM_COM_A429_SSM_Avionics_Label_041 : Outport  Port=241
  V_BCM_COM_A429_SSM_Avionics_Label_042 : Outport  Port=242
  V_BCM_COM_A429_SSM_Avionics_Label_043 : Outport  Port=243
  V_BCM_COM_A429_SSM_Avionics_Label_050 : Outport  Port=244
  V_BCM_COM_A429_SSM_DFCS_Label_105 : Outport  Port=245
  V_BCM_COM_A429_Wheel_Speed_W12 : Outport  Port=246
  V_BCM_COM_A429_Wheel_Speed_W34 : Outport  Port=247
  V_BCM_COM_A429_TACHO_Fail_W12 : Outport  Port=248
  V_BCM_COM_A429_TACHO_Fail_W34 : Outport  Port=249
  V_BCM_COM_A429_SSM_Avionics_Label_001 : Outport  Port=250
  V_BCM_COM_A429_SSM_Avionics_Label_002 : Outport  Port=251
  V_BCM_COM_A429_SSM_Avionics_Label_003 : Outport  Port=252
  V_BCM_COM_A429_SSM_Avionics_Label_004 : Outport  Port=253
  V_BCM_COM_A429_SSM_DFCS_Label_101 : Outport  Port=254
  V_BCM_COM_A429_SSM_DFCS_Label_102 : Outport  Port=255
  V_BCM_COM_A429_SSM_DFCS_Label_103 : Outport  Port=256
  V_BCM_COM_A429_SSM_DFCS_Label_104 : Outport  Port=257
  V_BCM_COM_A429_LH_Brake_Temp : Outport  Port=258
  V_BCM_COM_A429_RH_Brake_Temp : Outport  Port=259
  V_BCM_COM_A429_LH_Brake_Temp_Sensor_Fail : Outport  Port=260
  V_BCM_COM_A429_RH_Brake_Temp_Sensor_Fail : Outport  Port=261
  V_BCM_COM_A429_SSM_Avionics_Label_010 : Outport  Port=262
  V_BCM_COM_A429_SSM_Avionics_Label_011 : Outport  Port=263
  V_BCM_COM_A429_LNLG_Tire_Press : Outport  Port=264
  V_BCM_COM_A429_RNLG_Tire_Press : Outport  Port=265
  V_BCM_COM_A429_LMLG_Outboard_Tire_Press : Outport  Port=266
  V_BCM_COM_A429_LMLG_Inboard_Tire_Press : Outport  Port=267
  V_BCM_COM_A429_RMLG_Inboard_Tire_Press : Outport  Port=268
  V_BCM_COM_A429_RMLG_Outboard_Tire_Press : Outport  Port=269
  V_BCM_COM_A429_LNLG_Tire_Press_Sensor_Fail : Outport  Port=270
  V_BCM_COM_A429_RNLG_Tire_Press_Sensor_Fail : Outport  Port=271
  V_BCM_COM_A429_LMLG_Outboard_Tire_Press_Sensor_Fail : Outport  Port=272
  V_BCM_COM_A429_LMLG_Inboard_Tire_Press_Sensor_Fail : Outport  Port=273
  V_BCM_COM_A429_RMLG_Inboard_Tire_Press_Sensor_Fail : Outport  Port=274
  V_BCM_COM_A429_RMLG_Outboard_Tire_Press_Sensor_Fail : Outport  Port=275
  V_BCM_COM_A429_TPIS_Fail : Outport  Port=276
  V_BCM_COM_A429_SSM_Avionics_Label_012 : Outport  Port=277
  V_BCM_COM_A429_SSM_Avionics_Label_013 : Outport  Port=278
  V_BCM_COM_A429_SSM_Avionics_Label_014 : Outport  Port=279
  V_BCM_COM_A429_SSM_Avionics_Label_015 : Outport  Port=280
  V_BCM_COM_A429_SSM_Avionics_Label_016 : Outport  Port=281
  V_BCM_COM_A429_SSM_Avionics_Label_017 : Outport  Port=282
  V_BCM_COM_A429_Curr_Ord_Before_AS : Outport  Port=283
  V_BCM_COM_A429_AS_Curr_Order : Outport  Port=284
  V_BCM_COM_A429_SV_Current_Readback : Outport  Port=285
  V_BCM_COM_A429_SV_PT_In_Bar : Outport  Port=286
  V_BCM_COM_A429_SV_PT_In_PSI : Outport  Port=287
  V_BCM_COM_A429_Antiskid_Activity : Outport  Port=288
  V_BCM_COM_A429_ACCU_PT_Fail : Outport  Port=289
  V_BCM_COM_A429_SV_PT_Fail : Outport  Port=290
  V_BCM_COM_A429_SV_Fail : Outport  Port=291
  V_BCM_COM_A429_ACCU_PT : Outport  Port=292
  V_BCM_COM_A429_SELV_Disc_Sts_Rdbk : Outport  Port=293
  V_BCM_COM_A429_SELV_Disc_Sts_Rdbk_Val : Outport  Port=294
  V_BCM_COM_A429_SELV_Fail : Outport  Port=295
  V_BCM_COM_A429_SSM_Avionics_Label_020 : Outport  Port=296
  V_BCM_COM_A429_SSM_Avionics_Label_036 : Outport  Port=297
  V_BCM_COM_A429_SSM_Avionics_Label_037 : Outport  Port=298
  V_BCM_COM_A429_SSM_DFCS_Label_106 : Outport  Port=299
  V_BCM_COM_A429_SSM_DFCS_Label_107 : Outport  Port=300
  V_BCM_COM_A429_SSM_Avionics_Label_034 : Outport  Port=301
  V_BCM_COM_A429_SSM_Avionics_Label_035 : Outport  Port=302
  V_BCM_COM_A429_Park_Brake_ON : Outport  Port=303
  V_BCM_COM_A429_Park_Brake_Fail : Outport  Port=304
  V_BCM_COM_A429_Norm_FT_In_Progress : Outport  Port=305
  V_BCM_COM_A429_Alt_FT_In_Progress : Outport  Port=306
  V_BCM_COM_A429_Alt_FT_DFCS_Brkg_Req : Outport  Port=307
  V_BCM_COM_A429_Brk_Residual_Press : Outport  Port=308
  V_BCM_COM_A429_PLT_Not_Performed : Outport  Port=309
  V_BCM_COM_A429_Avionics_Comm_Fail_RX : Outport  Port=310
  V_BCM_COM_A429_DFCS_Decel_Law_Inhib : Outport  Port=311
  V_BCM_COM_A429_LH_Brkg_Cmd_Fdbk : Outport  Port=312
  V_BCM_COM_A429_RH_Brkg_Cmd_Fdbk : Outport  Port=313
  V_BCM_COM_A429_DFCS_LH_Brk_Pdl_Ord_Fail : Outport  Port=314
  V_BCM_COM_A429_DFCS_RH_Brk_Pdl_Ord_Fail : Outport  Port=315
  V_BCM_COM_A429_DFCS_A_Comm_Fail_RX : Outport  Port=316
  V_BCM_COM_A429_DFCS_B_Comm_Fail_RX : Outport  Port=317
  V_BCM_COM_A429_DFCS_A_Capsule_Fail : Outport  Port=318
  V_BCM_COM_A429_DFCS_B_Capsule_Fail : Outport  Port=319
  V_BCM_COM_A429_Pinprog_1 : Outport  Port=320
  V_BCM_COM_A429_Pinprog_2 : Outport  Port=321
  V_BCM_COM_A429_Pinprog_3 : Outport  Port=322
  V_BCM_COM_A429_Pinprog_4 : Outport  Port=323
  V_BCM_COM_A429_Pinprog_5 : Outport  Port=324
  V_BCM_COM_A429_PP_Channel_ID : Outport  Port=325
  V_BCM_COM_A429_DBCU_Dispatch_Conf : Outport  Port=326
  V_BCM_COM_A429_Maint_Mode_Active : Outport  Port=327
  V_BCM_COM_A429_Maint_Mode_Req_GND : Outport  Port=328
  V_BCM_COM_A429_Maint_Mode_Req_28V : Outport  Port=329
  V_BCM_COM_A429_Pinprog_Fail : Outport  Port=330
  V_BCM_COM_A429_Norm_Brake_Fail : Outport  Port=331
  V_BCM_COM_A429_BCM_Passivated : Outport  Port=332
  V_BCM_COM_A429_BCM_Fail : Outport  Port=333
  V_BCM_COM_A429_DBCU_Fail : Outport  Port=334
  V_BCM_COM_A429_Alternate_Fail : Outport  Port=335
  V_BCM_COM_A429_DBCU_LH_Brk_Cmd_Fdbk : Outport  Port=336
  V_BCM_COM_A429_DBCU_RH_Brk_Cmd_Fdbk : Outport  Port=337
  V_BCM_COM_A429_DBCU_Inhib_Opp_Side : Outport  Port=338
  V_BCM_COM_A429_DBCU_Alt_Mode : Outport  Port=339
  V_BCM_COM_A429_SSM_DFCS_Label_100 : Outport  Port=340
  V_BCM_COM_A429_Global_Wheel_Spd : Outport  Port=341
  V_BCM_COM_ETH_HYD_A_PRESS : Outport  Port=342
  V_BCM_COM_ETH_HYD_B_PRESS : Outport  Port=343
  V_BCM_COM_ETH_ENG1_RUNNING : Outport  Port=344
  V_BCM_COM_ETH_ENG2_RUNNING : Outport  Port=345
  V_BCM_COM_ETH_LMLG_Dnlk : Outport  Port=346
  V_BCM_COM_ETH_RMLG_Dnlk : Outport  Port=347
  V_BCM_COM_ETH_Lever_Up : Outport  Port=348
  V_BCM_COM_ETH_BCP_BCM_ALT_SW_ON_CMD : Outport  Port=349
  V_BCM_COM_ETH_MP_MAINT_MODE_CMD_GND : Outport  Port=350
  V_BCM_COM_ETH_MP_MAINT_MODE_CMD_28V : Outport  Port=351
  V_BCM_COM_ETH_MP_BCMA_ALT_DISP_SW : Outport  Port=352
  V_BCM_COM_ETH_PBSELV_ON_POS : Outport  Port=353
  V_BCM_COM_ETH_DBCU_BRK_ORDER_FAIL : Outport  Port=354
  V_BCM_COM_ETH_DISPATCH_SW_ON : Outport  Port=355
  V_BCM_COM_ETH_LH_DBCU_BRK_CMD_FDBK : Outport  Port=356
  V_BCM_COM_ETH_RH_DBCU_BRK_CMD_FDBK : Outport  Port=357
  V_BCM_COM_ETH_DBCU_FAILED : Outport  Port=358
  V_BCM_COM_ETH_ALT_MODE : Outport  Port=359
  V_BCM_COM_ETH_Opp_BCM_DBCU_INHIB : Outport  Port=360
  V_BCM_COM_ETH_LH_SV_Current_Order : Outport  Port=361
  V_BCM_COM_ETH_RH_SV_Current_Order : Outport  Port=362
  V_BCM_COM_ETH_SELV_High_Side_Cmd_Order : Outport  Port=363
  V_BCM_COM_ETH_DBCU_Inhib_Order : Outport  Port=364
  V_BCM_COM_ETH_FB_BCM_FAIL : Outport  Port=365
  V_BCM_COM_ETH_FB_DFCS_A_RX : Outport  Port=366
  V_BCM_COM_ETH_FB_DFCS_B_RX : Outport  Port=367
  V_BCM_COM_ETH_FB_MAINT_MODE_DIS : Outport  Port=368
  V_BCM_COM_ETH_FB_PARK_BRK_STATUS_DIS : Outport  Port=369
  V_BCM_COM_ETH_FB_BCM_DBCU_MODE_DIS : Outport  Port=370
  V_BCM_COM_ETH_FB_DBCU_SIMULT_ACT : Outport  Port=371
  V_BCM_COM_ETH_FB_DBCU_FAIL : Outport  Port=372
  V_BCM_COM_ETH_FB_DBCU_BRK_ORDER_FAIL : Outport  Port=373
  V_BCM_COM_ETH_FB_INHIB_FAIL : Outport  Port=374
  V_BCM_COM_ETH_FB_HYD_A_LOW_PRESS : Outport  Port=375
  V_BCM_COM_ETH_FB_HYD_B_LOW_PRESS : Outport  Port=376
  V_BCM_COM_ETH_FB_ACCU_LOW_PRESS : Outport  Port=377
  V_BCM_COM_ETH_FB_ACCU_PT_FAIL : Outport  Port=378
  V_BCM_COM_ETH_FB_BSELV_CMD_FAIL : Outport  Port=379
  V_BCM_COM_ETH_FB_BSELV_JCL : Outport  Port=380
  V_BCM_COM_ETH_FB_BSELV_JOP : Outport  Port=381
  V_BCM_COM_ETH_FB_LH_SV_PT_FAIL : Outport  Port=382
  V_BCM_COM_ETH_FB_LH_SV_CMD_FAIL : Outport  Port=383
  V_BCM_COM_ETH_FB_LH_SV_JCL : Outport  Port=384
  V_BCM_COM_ETH_FB_LH_SV_JOP : Outport  Port=385
  V_BCM_COM_ETH_FB_RH_SV_PT_FAIL : Outport  Port=386
  V_BCM_COM_ETH_FB_RH_SV_CMD_FAIL : Outport  Port=387
  V_BCM_COM_ETH_FB_RH_SV_JCL : Outport  Port=388
  V_BCM_COM_ETH_FB_RH_SV_JOP : Outport  Port=389
  V_BCM_COM_ETH_AC_State : Outport  Port=390
  V_BCM_COM_ETH_AC_Flight_Phase : Outport  Port=391
  V_BCM_COM_ETH_Braking_Mode : Outport  Port=392
  V_BCM_COM_ETH_Braking_Norm_FT_Seq : Outport  Port=393
  V_BCM_COM_ETH_Braking_Alt_FT_Seq : Outport  Port=394
  V_BCM_COM_ETH_FB_LG_LEVER_FAIL : Outport  Port=395
  V_BCM_COM_ETH_FB_LMLG_DWNLOCK_FAIL : Outport  Port=396
  V_BCM_COM_ETH_FB_RMLG_DWNLOCK_FAIL : Outport  Port=397
  V_BCM_COM_ETH_TARGET_HW_ID : Outport  Port=398
  V_BCM_COM_ETH_Invalid_Config : Outport  Port=399
  V_BCM_COM_ETH_FB_LH_OUT_TACHO_FAIL : Outport  Port=400
  V_BCM_COM_ETH_FB_LH_IN_TACHO_FAIL : Outport  Port=401
  V_BCM_COM_ETH_FB_RH_IN_TACHO_FAIL : Outport  Port=402
  V_BCM_COM_ETH_FB_RH_OUT_TACHO_FAIL : Outport  Port=403
  V_BCM_COM_ETH_TT_in_progress_id : Outport  Port=404
  V_BCM_COM_ETH_TT_rejection_cause : Outport  Port=405
  V_BCM_COM_ETH_TT_rejected : Outport  Port=406
  V_BCM_COM_ETH_TT_completed : Outport  Port=407
  V_BCM_COM_ETH_TT_result_significant : Outport  Port=408
  V_BCM_COM_BCM_DBCU_INHIBITION_Conf : Outport  Port=409
  V_BCM_COM_Target_DCL : Outport  Port=410
  V_BCM_COM_Decel_Ctrl_Loop_Act_Cond : Outport  Port=411
  wires:
  BCM_COM_PROC_P20/81 -> V_BCM_COM_LH_Ret_Brkg_Press_Cmd/1
  BCM_COM_PROC_P20/519 -> v_BCM_COM_MTB_in/1  "v_BCM_COM_MTB_in_1_BCMA"
  BCM_COM_PROC_P20/853 -> v_BCM_COM_Ret_Brkg_Press_Cmd/1  "v_BCM_COM_Ret_Brkg_Press_Cmd_1_BCMA"
  BCM_COM_PROC_P20/856 -> v_BCM_COM_Braking_Ste_Is_Normal/1  "v_BCM_COM_Braking_Ste_Is_Normal_1_BCMA"
  BCM_COM_PROC_P20/275 -> V_BCM_COM_A429_RMLG_Outboard_Tire_Press_Sensor_Fail/1
  BCM_COM_PROC_P20/866 -> v_BCM_COM_Press_Cmd_FT/1  "v_BCM_COM_Press_Cmd_FT_1_BCMA"
  BCM_COM_PROC_P20/638 -> Prb_ForcedMonitoringAuthorized (1)/1  "Prb_ForcedMonitoringAuthorized_3_BCMA"
  BCM_COM_PROC_P20/386 -> V_BCM_COM_ETH_FB_RH_SV_PT_FAIL/1
  BCM_COM_PROC_P20/805 -> v_BCM_COM_UF_DFCS_A_LMLGWOW_2_RX/1  "v_BCM_COM_UF_DFCS_A_LMLGWOW_2_RX_1_BCMA"
  BCM_COM_PROC_P20/32 -> V_BCM_COM_NLG_On_Gnd_State_Cons/1
  BCM_COM_PROC_P20/808 -> v_BCM_COM_CF_DFCS_B_LMLGWOW_2_RX/1  "v_BCM_COM_CF_DFCS_B_LMLGWOW_2_RX_1_BCMA"
  BCM_COM_PROC_P20/465 -> Prb_Previous_ReferenceSpeed (2)/1  "Prb_Previous_ReferenceSpeed_2_BCMA"
  BCM_COM_PROC_P20/382 -> V_BCM_COM_ETH_FB_LH_SV_PT_FAIL/1
  BCM_COM_PROC_P20/812 -> v_BCM_COM_CF_DFCS_B_RMLGWOW_2_RX/1  "v_BCM_COM_CF_DFCS_B_RMLGWOW_2_RX_1_BCMA"
  BCM_COM_PROC_P20/231 -> V_BCM_COM_RMLG_Outboard_Tire_Press_Cons_Val/1
  BCM_COM_PROC_P20/865 -> v_BCM_COM_SELV_FT/1  "v_BCM_COM_SELV_FT_1_BCMA"
  BCM_COM_PROC_P20/615 -> Prb_ForcedBigGammaStep (1)/1  "Prb_ForcedBigGammaStep_3_BCMA"
  BCM_COM_PROC_P20/864 -> v_BCM_COM_Rate_Lim_Law/1  "v_BCM_COM_Rate_Lim_Law_1_BCMA"
  BCM_COM_PROC_P20/861 -> PRB_RateLimitationActivation (1)/1  "PRB_RateLimitationActivation_1_BCMA"
  BCM_COM_PROC_P20/863 -> v_BCM_COM_Press_Rate_Lim_Inhib_Cond/1  "v_BCM_COM_Press_Rate_Lim_Inhib_Cond_1_BCMA"
  BCM_COM_PROC_P20/852 -> v_BCM_COM_Touchdown_Not_Active/1  "v_BCM_COM_Touchdown_Not_Active_1_BCMA"
  BCM_COM_PROC_P20/433 -> Prb_HydroplaneCondition (1)/1  "Prb_HydroplaneCondition_3_BCMA"
  BCM_COM_PROC_P20/859 -> PRB_BrakeFilled/1  "PRB_BrakeFilled_2_BCMA"
  BCM_COM_PROC_P20/431 -> Prb_OnGroundAfterHydroTransition (1)/1  "Prb_OnGroundAfterHydroTransition_3_BCMA"
  BCM_COM_PROC_P20/854 -> v_BCM_COM_Func_Test_Press_Cmd/1  "v_BCM_COM_Func_Test_Press_Cmd_1_BCMA"
  BCM_COM_PROC_P20/500 -> Prb_HydroplaneAccelCond (4)/1  "Prb_HydroplaneAccelCond_1_BCMA"
  BCM_COM_PROC_P20/851 -> v_BCM_COM_Custom_Brkg_Cmd/1  "v_BCM_COM_Custom_Brkg_Cmd_1_BCMA"
  BCM_COM_PROC_P20/759 -> v_BCM_COM_CF_HYD_A_PRESS_RX/1  "v_BCM_COM_CF_HYD_A_PRESS_RX_1_BCMA"
  BCM_COM_PROC_P20/844 -> v_BCM_COM_CF_DFCS_B_TLA_ABOVE_IDLE_RX/1  "v_BCM_COM_CF_DFCS_B_TLA_ABOVE_IDLE_RX_1_BCMA"
  BCM_COM_PROC_P20/847 -> Prb_SelectedPressureOrder_i/1  "Prb_SelectedPressureOrder_i_1_BCMA"
  BCM_COM_PROC_P20/850 -> v_BCM_COM_Custom_Braking_Mode/1  "v_BCM_COM_Custom_Braking_Mode_1_BCMA"
  BCM_COM_PROC_P20/419 -> Prb_HydroplaneAcceleration/1  "Prb_HydroplaneAcceleration_5_BCMA"
  V_BCM_COM_CF_RH_SV_JOP/1 -> DTC227/1
  BCM_COM_PROC_P20/741 -> Prb_MinimalTargetDecel (3)/1  "Prb_MinimalTargetDecel_1_BCMA"
  BCM_COM_PROC_P20/641 -> Prb_CommandedPressureTheorCurrent (2)/1  "Prb_CommandedPressureTheorCurrent_2_BCMA"
  BCM_COM_PROC_P20/34 -> V_BCM_COM_RH_Braking_Cmd_Cons/1
  BCM_COM_PROC_P20/849 -> Prb_SpunUpCondition_i/1  "Prb_SpunUpCondition_i_1_BCMA"
  BCM_COM_PROC_P20/848 -> Prb_SpunUpProtectedBrakingOrder/1  "Prb_SpunUpProtectedBrakingOrder_1_BCMA"
  BCM_COM_PROC_P20/837 -> v_BCM_COM_CF_DFCS_B_DBCU_ALT_MODE_2_RX/1  "v_BCM_COM_CF_DFCS_B_DBCU_ALT_MODE_2_RX_1_BCMA"
  BCM_COM_PROC_P20/418 -> Prb_HydroplaneAccelCond/1  "Prb_HydroplaneAccelCond_5_BCMA"
  BCM_COM_PROC_P20/514 -> v_BCM_COM_ATB_out/1  "v_BCM_COM_ATB_out_1_BCMA"
  BCM_COM_PROC_P20/414 -> Prb_SpunUpCondition/1  "Prb_SpunUpCondition_4_BCMA"
  BCM_COM_PROC_P20/838 -> v_BCM_COM_CF_DFCS_B_DBCU_ALT_MODE_1_RX/1  "v_BCM_COM_CF_DFCS_B_DBCU_ALT_MODE_1_RX_1_BCMA"
  BCM_COM_PROC_P20/455 -> Prb_HydroplaneAcceleration (2)/1  "Prb_HydroplaneAcceleration_3_BCMA"
  BCM_COM_PROC_P20/199 -> V_BCM_COM_LH_DBCU_BRK_CMD_FDBK_Cons/1
  BCM_COM_PROC_P20/843 -> v_BCM_COM_CF_DFCS_A_TLA_ABOVE_IDLE_RX/1  "v_BCM_COM_CF_DFCS_A_TLA_ABOVE_IDLE_RX_1_BCMA"
  BCM_COM_PROC_P20/842 -> v_BCM_COM_UF_DFCS_A_DBCU_ALT_MODE_1_RX/1  "v_BCM_COM_UF_DFCS_A_DBCU_ALT_MODE_1_RX_1_BCMA"
  BCM_COM_PROC_P20/543 -> Prb_SoftSpeedMaximum/1  "Prb_SoftSpeedMaximum_4_BCMA"
  BCM_COM_PROC_P20/841 -> v_BCM_COM_UF_DFCS_A_DBCU_ALT_MODE_2_RX/1  "v_BCM_COM_UF_DFCS_A_DBCU_ALT_MODE_2_RX_1_BCMA"
  BCM_COM_PROC_P20/839 -> v_BCM_COM_UF_DFCS_B_DBCU_ALT_MODE_2_RX/1  "v_BCM_COM_UF_DFCS_B_DBCU_ALT_MODE_2_RX_1_BCMA"
  BCM_COM_PROC_P20/708 -> Prb_SoftSpeedMaximum (3)/1  "Prb_SoftSpeedMaximum_1_BCMA"
  BCM_COM_PROC_P20/259 -> V_BCM_COM_A429_RH_Brake_Temp/1
  BCM_COM_PROC_P20/201 -> V_BCM_COM_RH_DBCU_BRK_CMD_FDBK_Cons/1
  BCM_COM_PROC_P20/155 -> V_BCM_COM_Hyd_A_Press_Unconf_Flt/1
  BCM_COM_PROC_P20/409 -> V_BCM_COM_BCM_DBCU_INHIBITION_Conf/1
  BCM_COM_PROC_P20/826 -> v_BCM_COM_UF_DFCS_B_NLGWOW_2_RX/1  "v_BCM_COM_UF_DFCS_B_NLGWOW_2_RX_1_BCMA"
  BCM_COM_PROC_P20/830 -> v_BCM_COM_UF_DFCS_B_LMLGWOW_1_RX/1  "v_BCM_COM_UF_DFCS_B_LMLGWOW_1_RX_1_BCMA"
  BCM_COM_PROC_P20/836 -> v_BCM_COM_CF_DFCS_A_DBCU_ALT_MODE_2_RX/1  "v_BCM_COM_CF_DFCS_A_DBCU_ALT_MODE_2_RX_1_BCMA"
  BCM_COM_PROC_P20/660 -> Prb_StateSignalValidityCondition (2)/1  "Prb_StateSignalValidityCondition_2_BCMA"
  BCM_COM_PROC_P20/777 -> v_BCM_COM_CF_DFCS_B_GND_SPEED_RX/1  "v_BCM_COM_CF_DFCS_B_GND_SPEED_RX_1_BCMA"
  BCM_COM_PROC_P20/584 -> Prb_AutomateFilteredPressure (1)/1  "Prb_AutomateFilteredPressure_3_BCMA"
  BCM_COM_PROC_P20/835 -> v_BCM_COM_CF_DFCS_A_DBCU_ALT_MODE_1_RX/1  "v_BCM_COM_CF_DFCS_A_DBCU_ALT_MODE_1_RX_1_BCMA"
  BCM_COM_PROC_P20/834 -> v_BCM_COM_UF_DFCS_B_DECEL_LAW_INHIB_RX/1  "v_BCM_COM_UF_DFCS_B_DECEL_LAW_INHIB_RX_1_BCMA"
  BCM_COM_PROC_P20/712 -> Prb_ResearchModeCondition (3)/1  "Prb_ResearchModeCondition_1_BCMA"
  BCM_COM_PROC_P20/491 -> v_BCM_COM_Brkg_SELV_High_Side_FT_Cond/1  "v_BCM_COM_Brkg_SELV_High_Side_FT_Cond_1_BCMA"
  BCM_COM_PROC_P20/833 -> v_BCM_COM_UF_DFCS_A_DECEL_LAW_INHIB_RX/1  "v_BCM_COM_UF_DFCS_A_DECEL_LAW_INHIB_RX_1_BCMA"
  BCM_COM_PROC_P20/827 -> v_BCM_COM_UF_DFCS_B_NLGWOW_1_RX/1  "v_BCM_COM_UF_DFCS_B_NLGWOW_1_RX_1_BCMA"
  BCM_COM_PROC_P20/782 -> v_BCM_COM_UF_DFCS_B_ACCEL_RX/1  "v_BCM_COM_UF_DFCS_B_ACCEL_RX_1_BCMA"
  BCM_COM_PROC_P20/821 -> v_BCM_COM_UF_DFCS_B_VALWOW_1_RX/1  "v_BCM_COM_UF_DFCS_B_VALWOW_1_RX_1_BCMA"
  BCM_COM_PROC_P20/402 -> V_BCM_COM_ETH_FB_RH_IN_TACHO_FAIL/1
  BCM_COM_PROC_P20/401 -> V_BCM_COM_ETH_FB_LH_IN_TACHO_FAIL/1
  BCM_COM_PROC_P20/86 -> V_BCM_COM_DBCU_FT_Inhib_Order/1
  BCM_COM_PROC_P20/822 -> v_BCM_COM_UF_DFCS_B_RMLGWOW_3_RX/1  "v_BCM_COM_UF_DFCS_B_RMLGWOW_3_RX_1_BCMA"
  BCM_COM_PROC_P20/825 -> v_BCM_COM_UF_DFCS_B_NLGWOW_3_RX/1  "v_BCM_COM_UF_DFCS_B_NLGWOW_3_RX_1_BCMA"
  BCM_COM_PROC_P20/815 -> v_BCM_COM_CF_DFCS_B_NLGWOW_2_RX/1  "v_BCM_COM_CF_DFCS_B_NLGWOW_2_RX_1_BCMA"
  BCM_COM_PROC_P20/105 -> V_BCM_COM_Hyd_A_Press_Cons/1
  BCM_COM_PROC_P20/818 -> v_BCM_COM_CF_DFCS_B_VALWOW_2_RX/1  "v_BCM_COM_CF_DFCS_B_VALWOW_2_RX_1_BCMA"
  BCM_COM_PROC_P20/819 -> v_BCM_COM_UF_DFCS_B_VALWOW_3_RX/1  "v_BCM_COM_UF_DFCS_B_VALWOW_3_RX_1_BCMA"
  BCM_COM_PROC_P20/388 -> V_BCM_COM_ETH_FB_RH_SV_JCL/1
  BCM_COM_PROC_P20/202 -> V_BCM_COM_RH_DBCU_BRK_CMD_FDBK_Cons_Val/1
  BCM_COM_PROC_P20/814 -> v_BCM_COM_CF_DFCS_B_NLGWOW_1_RX/1  "v_BCM_COM_CF_DFCS_B_NLGWOW_1_RX_1_BCMA"
  BCM_COM_PROC_P20/263 -> V_BCM_COM_A429_SSM_Avionics_Label_011/1
  BCM_COM_PROC_P20/813 -> v_BCM_COM_CF_DFCS_B_NLGWOW_3_RX/1  "v_BCM_COM_CF_DFCS_B_NLGWOW_3_RX_1_BCMA"
  BCM_COM_PROC_P20/811 -> v_BCM_COM_CF_DFCS_B_RMLGWOW_1_RX/1  "v_BCM_COM_CF_DFCS_B_RMLGWOW_1_RX_1_BCMA"
  BCM_COM_PROC_P20/803 -> v_BCM_COM_UF_DFCS_A_NLGWOW_1_RX/1  "v_BCM_COM_UF_DFCS_A_NLGWOW_1_RX_1_BCMA"
  BCM_COM_PROC_P20/304 -> V_BCM_COM_A429_Park_Brake_Fail/1
  BCM_COM_PROC_P20/810 -> v_BCM_COM_CF_DFCS_B_RMLGWOW_3_RX/1  "v_BCM_COM_CF_DFCS_B_RMLGWOW_3_RX_1_BCMA"
  BCM_COM_PROC_P20/794 -> v_BCM_COM_CF_DFCS_A_VALWOW_2_RX/1  "v_BCM_COM_CF_DFCS_A_VALWOW_2_RX_1_BCMA"
  BCM_COM_PROC_P20/186 -> V_BCM_COM_UTC_Time_Minutes_Cons_Val/1
  BCM_COM_PROC_P20/302 -> V_BCM_COM_A429_SSM_Avionics_Label_035/1
  BCM_COM_PROC_P20/686 -> Prb_MinimalTargetDecel (2)/1  "Prb_MinimalTargetDecel_2_BCMA"
  BCM_COM_PROC_P20/785 -> v_BCM_COM_CF_DFCS_A_LMLGWOW_3_RX/1  "v_BCM_COM_CF_DFCS_A_LMLGWOW_3_RX_1_BCMA"
  BCM_COM_PROC_P20/297 -> V_BCM_COM_A429_SSM_Avionics_Label_036/1
  BCM_COM_PROC_P20/806 -> v_BCM_COM_UF_DFCS_A_LMLGWOW_1_RX/1  "v_BCM_COM_UF_DFCS_A_LMLGWOW_1_RX_1_BCMA"
  BCM_COM_PROC_P20/804 -> v_BCM_COM_UF_DFCS_A_LMLGWOW_3_RX/1  "v_BCM_COM_UF_DFCS_A_LMLGWOW_3_RX_1_BCMA"
  BCM_COM_PROC_P20/381 -> V_BCM_COM_ETH_FB_BSELV_JOP/1
  BCM_COM_PROC_P20/795 -> v_BCM_COM_UF_DFCS_A_VALWOW_3_RX/1  "v_BCM_COM_UF_DFCS_A_VALWOW_3_RX_1_BCMA"
  BCM_COM_PROC_P20/798 -> v_BCM_COM_UF_DFCS_A_RMLGWOW_3_RX/1  "v_BCM_COM_UF_DFCS_A_RMLGWOW_3_RX_1_BCMA"
  BCM_COM_PROC_P20/802 -> v_BCM_COM_UF_DFCS_A_NLGWOW_2_RX/1  "v_BCM_COM_UF_DFCS_A_NLGWOW_2_RX_1_BCMA"
  BCM_COM_PROC_P20/378 -> V_BCM_COM_ETH_FB_ACCU_PT_FAIL/1
  BCM_COM_PROC_P20/801 -> v_BCM_COM_UF_DFCS_A_NLGWOW_3_RX/1  "v_BCM_COM_UF_DFCS_A_NLGWOW_3_RX_1_BCMA"
  BCM_COM_PROC_P20/592 -> Prb_UncorrectedMinimaltargetDecel (1)/1  "Prb_UncorrectedMinimaltargetDecel_3_BCMA"
  BCM_COM_PROC_P20/748 -> Prb_ForcedMonitoringAuthorized (3)/1  "Prb_ForcedMonitoringAuthorized_1_BCMA"
  BCM_COM_PROC_P20/800 -> v_BCM_COM_UF_DFCS_A_RMLGWOW_1_RX/1  "v_BCM_COM_UF_DFCS_A_RMLGWOW_1_RX_1_BCMA"
  BCM_COM_PROC_P20/177 -> V_BCM_COM_DFCS_A_DBCU_Alt_Mode_1_Val/1
  BCM_COM_PROC_P20/799 -> v_BCM_COM_UF_DFCS_A_RMLGWOW_2_RX/1  "v_BCM_COM_UF_DFCS_A_RMLGWOW_2_RX_1_BCMA"
  BCM_COM_PROC_P20/441 -> Prb_UnlimitedReferenceSpeed_3 (1)/1  "Prb_UnlimitedReferenceSpeed_3_3_BCMA"
  BCM_COM_PROC_P20/790 -> v_BCM_COM_CF_DFCS_A_NLGWOW_1_RX/1  "v_BCM_COM_CF_DFCS_A_NLGWOW_1_RX_1_BCMA"
  BCM_COM_PROC_P20/792 -> v_BCM_COM_CF_DFCS_A_VALWOW_3_RX/1  "v_BCM_COM_CF_DFCS_A_VALWOW_3_RX_1_BCMA"
  BCM_COM_PROC_P20/444 -> Prb_UnlimitedReferenceSpeed_4 (1)/1  "Prb_UnlimitedReferenceSpeed_4_3_BCMA"
  BCM_COM_PROC_P20/791 -> v_BCM_COM_CF_DFCS_A_NLGWOW_2_RX/1  "v_BCM_COM_CF_DFCS_A_NLGWOW_2_RX_1_BCMA"
  BCM_COM_PROC_P20/832 -> v_BCM_COM_CF_DFCS_B_DECEL_LAW_INHIB_RX/1  "v_BCM_COM_CF_DFCS_B_DECEL_LAW_INHIB_RX_1_BCMA"
  BCM_COM_PROC_P20/789 -> v_BCM_COM_CF_DFCS_A_NLGWOW_3_RX/1  "v_BCM_COM_CF_DFCS_A_NLGWOW_3_RX_1_BCMA"
  BCM_COM_PROC_P20/757 -> v_BCM_COM_UF_ENG_2_RUN_RX/1  "v_BCM_COM_UF_ENG_2_RUN_RX_1_BCMA"
  BCM_COM_PROC_P20/781 -> v_BCM_COM_UF_DFCS_B_GND_SPEED_RX/1  "v_BCM_COM_UF_DFCS_B_GND_SPEED_RX_1_BCMA"
  BCM_COM_PROC_P20/787 -> v_BCM_COM_CF_DFCS_A_RMLGWOW_1_RX/1  "v_BCM_COM_CF_DFCS_A_RMLGWOW_1_RX_1_BCMA"
  BCM_COM_PROC_P20/14 -> V_BCM_COM_AC_Pitch_Ang_Cons_Val/1
  BCM_COM_PROC_P20/786 -> v_BCM_COM_CF_DFCS_A_RMLGWOW_3_RX/1  "v_BCM_COM_CF_DFCS_A_RMLGWOW_3_RX_1_BCMA"
  BCM_COM_PROC_P20/778 -> v_BCM_COM_CF_DFCS_B_ACCEL_RX/1  "v_BCM_COM_CF_DFCS_B_ACCEL_RX_1_BCMA"
  BCM_COM_PROC_P20/377 -> V_BCM_COM_ETH_FB_ACCU_LOW_PRESS/1
  BCM_COM_PROC_P20/114 -> V_BCM_COM_Big_Gamma_Trig_Out_W12/1
  BCM_COM_PROC_P20/779 -> v_BCM_COM_CF_DFCS_B_PITCH_RX/1  "v_BCM_COM_CF_DFCS_B_PITCH_RX_1_BCMA"
  BCM_COM_PROC_P20/784 -> v_BCM_COM_CF_DFCS_A_LMLGWOW_2_RX/1  "v_BCM_COM_CF_DFCS_A_LMLGWOW_2_RX_1_BCMA"
  BCM_COM_PROC_P20/776 -> v_BCM_COM_UF_DFCS_A_PITCH_RX/1  "v_BCM_COM_UF_DFCS_A_PITCH_RX_1_BCMA"
  BCM_COM_PROC_P20/415 -> Prb_HydroplaneCondition/1  "Prb_HydroplaneCondition_4_BCMA"
  BCM_COM_PROC_P20/775 -> v_BCM_COM_UF_DFCS_A_GND_SPEED_RX/1  "v_BCM_COM_UF_DFCS_A_GND_SPEED_RX_1_BCMA"
  BCM_COM_PROC_P20/525 -> v_BCM_COM_MLG_Downlock_State_Cond/1  "v_BCM_COM_MLG_Downlock_State_Cond_1_BCMA"
  BCM_COM_PROC_P20/64 -> v_BCM_COM_FT_Seq/1
  BCM_COM_PROC_P20/371 -> V_BCM_COM_ETH_FB_DBCU_SIMULT_ACT/1
  BCM_COM_PROC_P20/773 -> v_BCM_COM_CF_DFCS_A_PITCH_RX/1  "v_BCM_COM_CF_DFCS_A_PITCH_RX_1_BCMA"
  BCM_COM_PROC_P20/772 -> v_BCM_COM_CF_DFCS_A_ACCEL_RX/1  "v_BCM_COM_CF_DFCS_A_ACCEL_RX_1_BCMA"
  BCM_COM_PROC_P20/770 -> v_BCM_COM_UF_DFCS_A_LH_BRK_CMD_RX/1  "v_BCM_COM_UF_DFCS_A_LH_BRK_CMD_RX_1_BCMA"
  BCM_COM_PROC_P20/335 -> V_BCM_COM_A429_Alternate_Fail/1
  BCM_COM_PROC_P20/768 -> v_BCM_COM_UF_DFCS_B_LH_BRK_CMD_RX/1  "v_BCM_COM_UF_DFCS_B_LH_BRK_CMD_RX_1_BCMA"
  BCM_COM_PROC_P20/367 -> V_BCM_COM_ETH_FB_DFCS_B_RX/1
  BCM_COM_PROC_P20/767 -> v_BCM_COM_UF_DFCS_B_RH_BRK_CMD_RX/1  "v_BCM_COM_UF_DFCS_B_RH_BRK_CMD_RX_1_BCMA"
  BCM_COM_PROC_P20/766 -> v_BCM_COM_CF_DFCS_A_LH_BRK_CMD_RX/1  "v_BCM_COM_CF_DFCS_A_LH_BRK_CMD_RX_1_BCMA"
  BCM_COM_PROC_P20/765 -> v_BCM_COM_CF_DFCS_A_RH_BRK_CMD_RX/1  "v_BCM_COM_CF_DFCS_A_RH_BRK_CMD_RX_1_BCMA"
  BCM_COM_PROC_P20/360 -> V_BCM_COM_ETH_Opp_BCM_DBCU_INHIB/1
  BCM_COM_PROC_P20/361 -> V_BCM_COM_ETH_LH_SV_Current_Order/1
  DTC207/1 -> BCM_COM_PROC_P20/207
  BCM_COM_PROC_P20/764 -> v_BCM_COM_CF_DFCS_B_LH_BRK_CMD_RX/1  "v_BCM_COM_CF_DFCS_B_LH_BRK_CMD_RX_1_BCMA"
  BCM_COM_PROC_P20/336 -> V_BCM_COM_A429_DBCU_LH_Brk_Cmd_Fdbk/1
  BCM_COM_PROC_P20/163 -> V_BCM_COM_DFCS_B_AC_Long_Accel_Val/1
  BCM_COM_PROC_P20/363 -> V_BCM_COM_ETH_SELV_High_Side_Cmd_Order/1
  BCM_COM_PROC_P20/762 -> v_BCM_COM_UF_HYD_B_PRESS_RX/1  "v_BCM_COM_UF_HYD_B_PRESS_RX_1_BCMA"
  BCM_COM_PROC_P20/354 -> V_BCM_COM_ETH_DBCU_BRK_ORDER_FAIL/1
  BCM_COM_PROC_P20/761 -> v_BCM_COM_CF_HYD_B_PRESS_RX/1  "v_BCM_COM_CF_HYD_B_PRESS_RX_1_BCMA"
  BCM_COM_PROC_P20/758 -> v_BCM_COM_CF_ENG_2_RUN_RX/1  "v_BCM_COM_CF_ENG_2_RUN_RX_1_BCMA"
  BCM_COM_PROC_P20/359 -> V_BCM_COM_ETH_ALT_MODE/1
  BCM_COM_PROC_P20/755 -> v_BCM_COM_CF_ENG_1_RUN_RX/1  "v_BCM_COM_CF_ENG_1_RUN_RX_1_BCMA"
  BCM_COM_PROC_P20/406 -> V_BCM_COM_ETH_TT_rejected/1
  BCM_COM_PROC_P20/410 -> V_BCM_COM_Target_DCL/1
  BCM_COM_PROC_P20/752 -> PRB_GroundStopSlowCond/1  "PRB_GroundStopSlowCond_1_BCMA"
  BCM_COM_PROC_P20/192 -> V_BCM_COM_RH_DBCU_BRK_CMD_FDBK_Conf/1
  BCM_COM_PROC_P20/751 -> v_BCM_COM_Automate_On_W12/1  "v_BCM_COM_Automate_On_W12_1_BCMA"
  BCM_COM_PROC_P20/711 -> Prb_BigSlipWatchDogTargetDecel (3)/1  "Prb_BigSlipWatchDogTargetDecel_1_BCMA"
  BCM_COM_PROC_P20/537 -> Prb_UncorrectedMinimaltargetDecel/1  "Prb_UncorrectedMinimaltargetDecel_4_BCMA"
  BCM_COM_PROC_P20/750 -> v_BCM_COM_Automate_On_W34/1  "v_BCM_COM_Automate_On_W34_1_BCMA"
  BCM_COM_PROC_P20/729 -> Prb_BigSlipStepAuthorize (3)/1  "Prb_BigSlipStepAuthorize_1_BCMA"
  BCM_COM_PROC_P20/573 -> Prb_AutomateState/1  "Prb_AutomateState_4_BCMA"
  BCM_COM_PROC_P20/749 -> v_BCM_COM_Automate_WD_Frozen/1  "v_BCM_COM_Automate_WD_Frozen_1_BCMA"
  BCM_COM_PROC_P20/347 -> V_BCM_COM_ETH_RMLG_Dnlk/1
  BCM_COM_PROC_P20/746 -> Prb_StepSize (3)/1  "Prb_StepSize_1_BCMA"
  V_BCM_COM_MP_MAINT_MODE_CMD_GND_Acq/1 -> DTC173/1
  BCM_COM_PROC_P20/642 -> Prb_AsLowPassTheorPressure (2)/1  "Prb_AsLowPassTheorPressure_2_BCMA"
  BCM_COM_PROC_P20/745 -> Prb_DenAccuBigSlip (3)/1  "Prb_DenAccuBigSlip_1_BCMA"
  BCM_COM_PROC_P20/744 -> Prb_WheelSkidSmoothAverage (3)/1  "Prb_WheelSkidSmoothAverage_1_BCMA"
  BCM_COM_PROC_P20/348 -> V_BCM_COM_ETH_Lever_Up/1
  BCM_COM_PROC_P20/743 -> Prb_SofteningSpeed (3)/1  "Prb_SofteningSpeed_1_BCMA"
  BCM_COM_PROC_P20/337 -> V_BCM_COM_A429_DBCU_RH_Brk_Cmd_Fdbk/1
  BCM_COM_PROC_P20/742 -> Prb_OptimalSpeed (3)/1  "Prb_OptimalSpeed_1_BCMA"
  BCM_COM_PROC_P20/340 -> V_BCM_COM_A429_SSM_DFCS_Label_100/1
  V_BCM_COM_CF_LH_SV_OC/1 -> DTC198/1
  BCM_COM_PROC_P20/740 -> Prb_TargetSpeedDelta (3)/1  "Prb_TargetSpeedDelta_1_BCMA"
  BCM_COM_PROC_P20/738 -> Prb_AutomateState (3)/1  "Prb_AutomateState_1_BCMA"
  BCM_COM_PROC_P20/736 -> Prb_TransitionGammaDecrease (3)/1  "Prb_TransitionGammaDecrease_1_BCMA"
  BCM_COM_PROC_P20/596 -> Prb_SoftSpeedCountOrder (1)/1  "Prb_SoftSpeedCountOrder_3_BCMA"
  BCM_COM_PROC_P20/735 -> Prb_TransitionSmallSlipStep (3)/1  "Prb_TransitionSmallSlipStep_1_BCMA"
  BCM_COM_PROC_P20/734 -> Prb_ForcedSmallSlipStep (3)/1  "Prb_ForcedSmallSlipStep_1_BCMA"
  BCM_COM_PROC_P20/637 -> Prb_TargetOverDecelInteg (1)/1  "Prb_TargetOverDecelInteg_3_BCMA"
  BCM_COM_PROC_P20/732 -> Prb_TransitionBigSlipStep (3)/1  "Prb_TransitionBigSlipStep_1_BCMA"
  BCM_COM_PROC_P20/558 -> Prb_NaturalBigSlipWatchDog/1  "Prb_NaturalBigSlipWatchDog_4_BCMA"
  BCM_COM_PROC_P20/731 -> Prb_NaturalBigSlipStep (3)/1  "Prb_NaturalBigSlipStep_1_BCMA"
  BCM_COM_PROC_P20/334 -> V_BCM_COM_A429_DBCU_Fail/1
  BCM_COM_PROC_P20/194 -> V_BCM_COM_DBCU_ALT_MODE_Conf/1
  BCM_COM_PROC_P20/730 -> Prb_ForcedBigSlipStep (3)/1  "Prb_ForcedBigSlipStep_1_BCMA"
  BCM_COM_PROC_P20/326 -> V_BCM_COM_A429_DBCU_Dispatch_Conf/1
  BCM_COM_PROC_P20/726 -> Prb_NaturalBigGammaStep (3)/1  "Prb_NaturalBigGammaStep_1_BCMA"
  BCM_COM_PROC_P20/725 -> Prb_ForcedBigGammaStep (3)/1  "Prb_ForcedBigGammaStep_1_BCMA"
  BCM_COM_PROC_P20/723 -> Prb_NaturalBigSlipWatchDog (3)/1  "Prb_NaturalBigSlipWatchDog_1_BCMA"
  BCM_COM_PROC_P20/793 -> v_BCM_COM_CF_DFCS_A_VALWOW_1_RX/1  "v_BCM_COM_CF_DFCS_A_VALWOW_1_RX_1_BCMA"
  BCM_COM_PROC_P20/252 -> V_BCM_COM_A429_SSM_Avionics_Label_003/1
  BCM_COM_PROC_P20/715 -> Prb_StateSignalValidityCondition (3)/1  "Prb_StateSignalValidityCondition_1_BCMA"
  BCM_COM_PROC_P20/267 -> V_BCM_COM_A429_LMLG_Inboard_Tire_Press/1
  BCM_COM_PROC_P20/722 -> Prb_ForcedBigSlipWatchDog (3)/1  "Prb_ForcedBigSlipWatchDog_1_BCMA"
  BCM_COM_PROC_P20/487 -> v_BCM_COM_Spun_Up_Condition_W12/1  "v_BCM_COM_Spun_Up_Condition_W12_1_BCMA"
  BCM_COM_PROC_P20/330 -> V_BCM_COM_A429_Pinprog_Fail/1
  BCM_COM_PROC_P20/721 -> Prb_SlowTrigCondition (3)/1  "Prb_SlowTrigCondition_1_BCMA"
  BCM_COM_PROC_P20/719 -> Prb_SlowStateCondition (3)/1  "Prb_SlowStateCondition_1_BCMA"
  BCM_COM_PROC_P20/718 -> Prb_FastStateCondition (3)/1  "Prb_FastStateCondition_1_BCMA"
  BCM_COM_PROC_P20/716 -> Prb_FastMonitoringCondition (3)/1  "Prb_FastMonitoringCondition_1_BCMA"
  BCM_COM_PROC_P20/325 -> V_BCM_COM_A429_PP_Channel_ID/1
  BCM_COM_PROC_P20/281 -> V_BCM_COM_A429_SSM_Avionics_Label_016/1
  BCM_COM_PROC_P20/422 -> Prb_RefSpeedLowLimit (1)/1  "Prb_RefSpeedLowLimit_8_BCMA"
  BCM_COM_PROC_P20/714 -> Prb_TransitionAntiskidBrakeLoss (3)/1  "Prb_TransitionAntiskidBrakeLoss_1_BCMA"
  BCM_COM_PROC_P20/710 -> Prb_AsBrkLossTargetDecel (3)/1  "Prb_AsBrkLossTargetDecel_1_BCMA"
  BCM_COM_PROC_P20/709 -> Prb_DecelerationDecrement (3)/1  "Prb_DecelerationDecrement_1_BCMA"
  BCM_COM_PROC_P20/307 -> V_BCM_COM_A429_Alt_FT_DFCS_Brkg_Req/1
  BCM_COM_PROC_P20/707 -> Prb_SoftSpeedResetOrder (3)/1  "Prb_SoftSpeedResetOrder_1_BCMA"
  BCM_COM_PROC_P20/318 -> V_BCM_COM_A429_DFCS_A_Capsule_Fail/1
  BCM_COM_PROC_P20/319 -> V_BCM_COM_A429_DFCS_B_Capsule_Fail/1
  BCM_COM_PROC_P20/706 -> Prb_SoftSpeedCountOrder (3)/1  "Prb_SoftSpeedCountOrder_1_BCMA"
  BCM_COM_PROC_P20/704 -> Prb_AutomateSofteningFreezingCond (3)/1  "Prb_AutomateSofteningFreezingCond_1_BCMA"
  BCM_COM_PROC_P20/536 -> Prb_AdhesionOpt/1  "Prb_AdhesionOpt_4_BCMA"
  BCM_COM_PROC_P20/332 -> V_BCM_COM_A429_BCM_Passivated/1
  BCM_COM_PROC_P20/702 -> Prb_UncorrectedMinimaltargetDecel (3)/1  "Prb_UncorrectedMinimaltargetDecel_1_BCMA"
  BCM_COM_PROC_P20/699 -> Prb_SvLowPassTheorCurrent (3)/1  "Prb_SvLowPassTheorCurrent_1_BCMA"
  BCM_COM_PROC_P20/391 -> V_BCM_COM_ETH_AC_Flight_Phase/1
  BCM_COM_PROC_P20/698 -> Prb_AsLowPassTheorCurrent (3)/1  "Prb_AsLowPassTheorCurrent_1_BCMA"
  BCM_COM_PROC_P20/316 -> V_BCM_COM_A429_DFCS_A_Comm_Fail_RX/1
  DTC219/1 -> BCM_COM_PROC_P20/219
  BCM_COM_PROC_P20/697 -> Prb_AsLowPassTheorPressure (3)/1  "Prb_AsLowPassTheorPressure_1_BCMA"
  BCM_COM_PROC_P20/538 -> Prb_BigGammaStepSize/1  "Prb_BigGammaStepSize_4_BCMA"
  BCM_COM_PROC_P20/696 -> Prb_CommandedPressureTheorCurrent (3)/1  "Prb_CommandedPressureTheorCurrent_1_BCMA"
  BCM_COM_PROC_P20/273 -> V_BCM_COM_A429_LMLG_Inboard_Tire_Press_Sensor_Fail/1
  BCM_COM_PROC_P20/665 -> Prb_FastTrigCondition (2)/1  "Prb_FastTrigCondition_2_BCMA"
  BCM_COM_PROC_P20/693 -> Prb_ForcedMonitoringAuthorized (2)/1  "Prb_ForcedMonitoringAuthorized_2_BCMA"
  BCM_COM_PROC_P20/549 -> Prb_TransitionAntiskidBrakeLoss/1  "Prb_TransitionAntiskidBrakeLoss_4_BCMA"
  BCM_COM_PROC_P20/692 -> Prb_TargetOverDecelInteg (2)/1  "Prb_TargetOverDecelInteg_2_BCMA"
  BCM_COM_PROC_P20/691 -> Prb_StepSize (2)/1  "Prb_StepSize_2_BCMA"
  BCM_COM_PROC_P20/649 -> Prb_AutomateSofteningFreezingCond (2)/1  "Prb_AutomateSofteningFreezingCond_2_BCMA"
  BCM_COM_PROC_P20/688 -> Prb_SofteningSpeed (2)/1  "Prb_SofteningSpeed_2_BCMA"
  BCM_COM_PROC_P20/684 -> Prb_ReferenceSpeedDelta (2)/1  "Prb_ReferenceSpeedDelta_2_BCMA"
  BCM_COM_PROC_P20/306 -> V_BCM_COM_A429_Alt_FT_In_Progress/1
  BCM_COM_PROC_P20/682 -> Prb_TransitionGammaIncrease (2)/1  "Prb_TransitionGammaIncrease_2_BCMA"
  BCM_COM_PROC_P20/389 -> V_BCM_COM_ETH_FB_RH_SV_JOP/1
  BCM_COM_PROC_P20/681 -> Prb_TransitionGammaDecrease (2)/1  "Prb_TransitionGammaDecrease_2_BCMA"
  BCM_COM_PROC_P20/679 -> Prb_ForcedSmallSlipStep (2)/1  "Prb_ForcedSmallSlipStep_2_BCMA"
  BCM_COM_PROC_P20/461 -> Prb_BrakingPhaseAcceleration (2)/1  "Prb_BrakingPhaseAcceleration_3_BCMA"
  BCM_COM_PROC_P20/678 -> Prb_NaturalSmallSlipStep (2)/1  "Prb_NaturalSmallSlipStep_2_BCMA"
  BCM_COM_PROC_P20/695 -> Prb_TheorCommandedPressure (3)/1  "Prb_TheorCommandedPressure_1_BCMA"
  BCM_COM_PROC_P20/295 -> V_BCM_COM_A429_SELV_Fail/1
  BCM_COM_PROC_P20/677 -> Prb_TransitionBigSlipStep (2)/1  "Prb_TransitionBigSlipStep_2_BCMA"
  BCM_COM_PROC_P20/739 -> Prb_ReferenceSpeedDelta (3)/1  "Prb_ReferenceSpeedDelta_1_BCMA"
  BCM_COM_PROC_P20/284 -> V_BCM_COM_A429_AS_Curr_Order/1
  BCM_COM_PROC_P20/286 -> V_BCM_COM_A429_SV_PT_In_Bar/1
  BCM_COM_PROC_P20/817 -> v_BCM_COM_CF_DFCS_B_VALWOW_1_RX/1  "v_BCM_COM_CF_DFCS_B_VALWOW_1_RX_1_BCMA"
  BCM_COM_PROC_P20/676 -> Prb_NaturalBigSlipStep (2)/1  "Prb_NaturalBigSlipStep_2_BCMA"
  BCM_COM_PROC_P20/675 -> Prb_ForcedBigSlipStep (2)/1  "Prb_ForcedBigSlipStep_2_BCMA"
  BCM_COM_PROC_P20/674 -> Prb_BigSlipStepAuthorize (2)/1  "Prb_BigSlipStepAuthorize_2_BCMA"
  BCM_COM_PROC_P20/291 -> V_BCM_COM_A429_SV_Fail/1
  BCM_COM_PROC_P20/75 -> V_BCM_COM_LH_Press_Reg_FT_Act_Cond/1
  BCM_COM_PROC_P20/671 -> Prb_NaturalBigGammaStep (2)/1  "Prb_NaturalBigGammaStep_2_BCMA"
  BCM_COM_PROC_P20/672 -> Prb_BigGammaThreshold (2)/1  "Prb_BigGammaThreshold_2_BCMA"
  BCM_COM_PROC_P20/670 -> Prb_ForcedBigGammaStep (2)/1  "Prb_ForcedBigGammaStep_2_BCMA"
  BCM_COM_PROC_P20/669 -> Prb_TransitionBigSlipWatchDog (2)/1  "Prb_TransitionBigSlipWatchDog_2_BCMA"
  V_BCM_COM_RNLG_Tire_Press_Acq/1 -> DTC177/1
  BCM_COM_PROC_P20/283 -> V_BCM_COM_A429_Curr_Ord_Before_AS/1
  BCM_COM_PROC_P20/667 -> Prb_ForcedBigSlipWatchDog (2)/1  "Prb_ForcedBigSlipWatchDog_2_BCMA"
  BCM_COM_PROC_P20/99 -> V_BCM_COM_Press_Cmd/1
  BCM_COM_PROC_P20/666 -> Prb_SlowTrigCondition (2)/1  "Prb_SlowTrigCondition_2_BCMA"
  BCM_COM_PROC_P20/664 -> Prb_SlowStateCondition (2)/1  "Prb_SlowStateCondition_2_BCMA"
  BCM_COM_PROC_P20/542 -> Prb_SoftSpeedResetOrder/1  "Prb_SoftSpeedResetOrder_4_BCMA"
  BCM_COM_PROC_P20/662 -> Prb_SlowMonitoringCondition (2)/1  "Prb_SlowMonitoringCondition_2_BCMA"
  DTC213/1 -> BCM_COM_PROC_P20/213
  BCM_COM_PROC_P20/661 -> Prb_FastMonitoringCondition (2)/1  "Prb_FastMonitoringCondition_2_BCMA"
  BCM_COM_PROC_P20/200 -> V_BCM_COM_LH_DBCU_BRK_CMD_FDBK_Cons_Val/1
  BCM_COM_PROC_P20/159 -> V_BCM_COM_DFCS_A_AC_Pitch_Angle_Val/1
  BCM_COM_PROC_P20/656 -> Prb_BigSlipWatchDogTargetDecel (2)/1  "Prb_BigSlipWatchDogTargetDecel_2_BCMA"
  BCM_COM_PROC_P20/272 -> V_BCM_COM_A429_LMLG_Outboard_Tire_Press_Sensor_Fail/1
  DTC174/1 -> BCM_COM_PROC_P20/174
  BCM_COM_PROC_P20/654 -> Prb_DecelerationDecrement (2)/1  "Prb_DecelerationDecrement_2_BCMA"
  BCM_COM_PROC_P20/653 -> Prb_SoftSpeedMaximum (2)/1  "Prb_SoftSpeedMaximum_2_BCMA"
  BCM_COM_PROC_P20/449 -> Prb_OnGroundAfterHydroTransition (2)/1  "Prb_OnGroundAfterHydroTransition_2_BCMA"
  BCM_COM_PROC_P20/753 -> PRB_GroundStopFastCond/1  "PRB_GroundStopFastCond_1_BCMA"
  BCM_COM_PROC_P20/651 -> Prb_SoftSpeedCountOrder (2)/1  "Prb_SoftSpeedCountOrder_2_BCMA"
  BCM_COM_PROC_P20/262 -> V_BCM_COM_A429_SSM_Avionics_Label_010/1
  BCM_COM_PROC_P20/650 -> Prb_SoftSpeedCounter (2)/1  "Prb_SoftSpeedCounter_2_BCMA"
  BCM_COM_PROC_P20/606 -> Prb_FastMonitoringCondition (1)/1  "Prb_FastMonitoringCondition_3_BCMA"
  BCM_COM_PROC_P20/648 -> Prb_BigGammaStepSize (2)/1  "Prb_BigGammaStepSize_2_BCMA"
  BCM_COM_PROC_P20/243 -> V_BCM_COM_A429_SSM_Avionics_Label_043/1
  BCM_COM_PROC_P20/351 -> V_BCM_COM_ETH_MP_MAINT_MODE_CMD_28V/1
  BCM_COM_PROC_P20/244 -> V_BCM_COM_A429_SSM_Avionics_Label_050/1
  V_BCM_COM_CF_SELV_JCL/1 -> DTC204/1
  BCM_COM_PROC_P20/647 -> Prb_UncorrectedMinimaltargetDecel (2)/1  "Prb_UncorrectedMinimaltargetDecel_2_BCMA"
  BCM_COM_PROC_P20/644 -> Prb_SvLowPassTheorCurrent (2)/1  "Prb_SvLowPassTheorCurrent_2_BCMA"
  BCM_COM_PROC_P20/190 -> V_BCM_COM_DBCU_DISPATCH_SW_ON_Conf/1
  BCM_COM_PROC_P20/238 -> V_BCM_COM_A429_SSM_Avionics_Label_032/1
  BCM_COM_PROC_P20/196 -> V_BCM_COM_DBCU_BRK_ORDER_FAIL_Cons_Val/1
  BCM_COM_PROC_P20/639 -> Prb_AutomateFilteredPressure (2)/1  "Prb_AutomateFilteredPressure_2_BCMA"
  BCM_COM_PROC_P20/253 -> V_BCM_COM_A429_SSM_Avionics_Label_004/1
  BCM_COM_PROC_P20/426 -> Prb_UnlimitedReferenceSpeed_4/1  "Prb_UnlimitedReferenceSpeed_4_4_BCMA"
  BCM_COM_PROC_P20/635 -> Prb_DenAccuBigSlip (1)/1  "Prb_DenAccuBigSlip_3_BCMA"
  BCM_COM_PROC_P20/234 -> V_BCM_COM_A429_SSM_Avionics_Label_021/1
  BCM_COM_PROC_P20/235 -> V_BCM_COM_A429_SSM_Avionics_Label_022/1
  BCM_COM_PROC_P20/633 -> Prb_SofteningSpeed (1)/1  "Prb_SofteningSpeed_3_BCMA"
  BCM_COM_PROC_P20/539 -> Prb_AutomateSofteningFreezingCond/1  "Prb_AutomateSofteningFreezingCond_4_BCMA"
  BCM_COM_PROC_P20/631 -> Prb_MinimalTargetDecel (1)/1  "Prb_MinimalTargetDecel_3_BCMA"
  V_BCM_COM_CF_BSELV_SC/1 -> DTC218/1
  BCM_COM_PROC_P20/629 -> Prb_ReferenceSpeedDelta (1)/1  "Prb_ReferenceSpeedDelta_3_BCMA"
  BCM_COM_PROC_P20/236 -> V_BCM_COM_A429_SSM_Avionics_Label_030/1
  BCM_COM_PROC_P20/628 -> Prb_AutomateState (1)/1  "Prb_AutomateState_3_BCMA"
  BCM_COM_PROC_P20/626 -> Prb_TransitionGammaDecrease (1)/1  "Prb_TransitionGammaDecrease_3_BCMA"
  BCM_COM_PROC_P20/432 -> Prb_SpunUpCondition (1)/1  "Prb_SpunUpCondition_3_BCMA"
  BCM_COM_PROC_P20/226 -> V_BCM_COM_LMLG_Inboard_Tire_Press_Cons/1
  BCM_COM_PROC_P20/621 -> Prb_NaturalBigSlipStep (1)/1  "Prb_NaturalBigSlipStep_3_BCMA"
  BCM_COM_PROC_P20/219 -> V_BCM_COM_Maint_Mode_State_Cons/1
  BCM_COM_PROC_P20/135 -> V_BCM_COM_Adhesion_In_Cons_W34/1
  BCM_COM_PROC_P20/620 -> Prb_ForcedBigSlipStep (1)/1  "Prb_ForcedBigSlipStep_3_BCMA"
  BCM_COM_PROC_P20/619 -> Prb_BigSlipStepAuthorize (1)/1  "Prb_BigSlipStepAuthorize_3_BCMA"
  BCM_COM_PROC_P20/211 -> V_BCM_COM_LH_Brake_Temp_Cons_Val/1
  BCM_COM_PROC_P20/220 -> V_BCM_COM_LNLG_Tire_Press_Cons/1
  BCM_COM_PROC_P20/617 -> Prb_BigGammaThreshold (1)/1  "Prb_BigGammaThreshold_3_BCMA"
  BCM_COM_PROC_P20/687 -> Prb_OptimalSpeed (2)/1  "Prb_OptimalSpeed_2_BCMA"
  BCM_COM_PROC_P20/224 -> V_BCM_COM_LMLG_Outboard_Tire_Press_Cons/1
  BCM_COM_PROC_P20/616 -> Prb_NaturalBigGammaStep (1)/1  "Prb_NaturalBigGammaStep_3_BCMA"
  BCM_COM_PROC_P20/210 -> V_BCM_COM_LH_Brake_Temp_Cons/1
  BCM_COM_PROC_P20/77 -> V_BCM_COM_LH_Press_Law_Brkg_Press_Cmd/1
  BCM_COM_PROC_P20/614 -> Prb_TransitionBigSlipWatchDog (1)/1  "Prb_TransitionBigSlipWatchDog_3_BCMA"
  BCM_COM_PROC_P20/613 -> Prb_NaturalBigSlipWatchDog (1)/1  "Prb_NaturalBigSlipWatchDog_3_BCMA"
  BCM_COM_PROC_P20/611 -> Prb_SlowTrigCondition (1)/1  "Prb_SlowTrigCondition_3_BCMA"
  BCM_COM_PROC_P20/610 -> Prb_FastTrigCondition (1)/1  "Prb_FastTrigCondition_3_BCMA"
  BCM_COM_PROC_P20/483 -> Prb_Previous_ReferenceSpeed (3)/1  "Prb_Previous_ReferenceSpeed_1_BCMA"
  BCM_COM_PROC_P20/658 -> Prb_TransitionBrakingInit (2)/1  "Prb_TransitionBrakingInit_2_BCMA"
  BCM_COM_PROC_P20/552 -> Prb_SlowMonitoringCondition/1  "Prb_SlowMonitoringCondition_4_BCMA"
  BCM_COM_PROC_P20/845 -> v_BCM_COM_UF_DFCS_B_TLA_ABOVE_IDLE_RX/1  "v_BCM_COM_UF_DFCS_B_TLA_ABOVE_IDLE_RX_1_BCMA"
  BCM_COM_PROC_P20/609 -> Prb_SlowStateCondition (1)/1  "Prb_SlowStateCondition_3_BCMA"
  BCM_COM_PROC_P20/607 -> Prb_SlowMonitoringCondition (1)/1  "Prb_SlowMonitoringCondition_3_BCMA"
  BCM_COM_PROC_P20/195 -> V_BCM_COM_DBCU_BRK_ORDER_FAIL_Cons/1
  BCM_COM_PROC_P20/605 -> Prb_StateSignalValidityCondition (1)/1  "Prb_StateSignalValidityCondition_3_BCMA"
  V_BCM_COM_RMLG_Outboard_Tire_Press_Acq/1 -> DTC189/1
  BCM_COM_PROC_P20/591 -> Prb_AdhesionOpt (1)/1  "Prb_AdhesionOpt_3_BCMA"
  BCM_COM_PROC_P20/603 -> Prb_TransitionBrakingInit (1)/1  "Prb_TransitionBrakingInit_3_BCMA"
  BCM_COM_PROC_P20/602 -> Prb_ResearchModeCondition (1)/1  "Prb_ResearchModeCondition_3_BCMA"
  BCM_COM_PROC_P20/179 -> V_BCM_COM_DFCS_B_DBCU_Alt_Mode_1_Val/1
  V_BCM_COM_SV_Current_Readback/1 -> DTC193/1
  BCM_COM_PROC_P20/601 -> Prb_BigSlipWatchDogTargetDecel (1)/1  "Prb_BigSlipWatchDogTargetDecel_3_BCMA"
  BCM_COM_PROC_P20/598 -> Prb_SoftSpeedMaximum (1)/1  "Prb_SoftSpeedMaximum_3_BCMA"
  BCM_COM_PROC_P20/597 -> Prb_SoftSpeedResetOrder (1)/1  "Prb_SoftSpeedResetOrder_3_BCMA"
  BCM_COM_PROC_P20/595 -> Prb_SoftSpeedCounter (1)/1  "Prb_SoftSpeedCounter_3_BCMA"
  BCM_COM_PROC_P20/590 -> Prb_Adhesion (1)/1  "Prb_Adhesion_3_BCMA"
  BCM_COM_PROC_P20/831 -> v_BCM_COM_CF_DFCS_A_DECEL_LAW_INHIB_RX/1  "v_BCM_COM_CF_DFCS_A_DECEL_LAW_INHIB_RX_1_BCMA"
  BCM_COM_PROC_P20/589 -> Prb_SvLowPassTheorCurrent (1)/1  "Prb_SvLowPassTheorCurrent_3_BCMA"
  BCM_COM_PROC_P20/208 -> V_BCM_COM_ACCU_PT_Cons_Val/1
  BCM_COM_PROC_P20/587 -> Prb_AsLowPassTheorPressure (1)/1  "Prb_AsLowPassTheorPressure_3_BCMA"
  BCM_COM_PROC_P20/157 -> V_BCM_COM_DFCS_A_AC_Gnd_Spd_Val/1
  BCM_COM_PROC_P20/586 -> Prb_CommandedPressureTheorCurrent (1)/1  "Prb_CommandedPressureTheorCurrent_3_BCMA"
  DTC188/1 -> BCM_COM_PROC_P20/188
  BCM_COM_PROC_P20/574 -> Prb_ReferenceSpeedDelta/1  "Prb_ReferenceSpeedDelta_4_BCMA"
  BCM_COM_PROC_P20/585 -> Prb_TheorCommandedPressure (1)/1  "Prb_TheorCommandedPressure_3_BCMA"
  BCM_COM_PROC_P20/583 -> Prb_ForcedMonitoringAuthorized/1  "Prb_ForcedMonitoringAuthorized_4_BCMA"
  BCM_COM_PROC_P20/26 -> V_BCM_COM_RMLG_On_Gnd_State/1
  BCM_COM_PROC_P20/582 -> Prb_TargetOverDecelInteg/1  "Prb_TargetOverDecelInteg_4_BCMA"
  BCM_COM_PROC_P20/188 -> V_BCM_COM_UTC_Time_Seconds_Cons_Val/1
  BCM_COM_PROC_P20/145 -> V_BCM_COM_Small_Slip_Trig_In_Cons_W34/1
  BCM_COM_PROC_P20/352 -> V_BCM_COM_ETH_MP_BCMA_ALT_DISP_SW/1
  BCM_COM_PROC_P20/581 -> Prb_StepSize/1  "Prb_StepSize_4_BCMA"
  BCM_COM_PROC_P20/357 -> V_BCM_COM_ETH_RH_DBCU_BRK_CMD_FDBK/1
  BCM_COM_PROC_P20/579 -> Prb_WheelSkidSmoothAverage/1  "Prb_WheelSkidSmoothAverage_4_BCMA"
  BCM_COM_PROC_P20/561 -> Prb_NaturalBigGammaStep/1  "Prb_NaturalBigGammaStep_4_BCMA"
  BCM_COM_PROC_P20/578 -> Prb_SofteningSpeed/1  "Prb_SofteningSpeed_4_BCMA"
  BCM_COM_PROC_P20/577 -> Prb_OptimalSpeed/1  "Prb_OptimalSpeed_4_BCMA"
  BCM_COM_PROC_P20/513 -> v_BCM_COM_ATB_in/1  "v_BCM_COM_ATB_in_1_BCMA"
  BCM_COM_PROC_P20/137 -> V_BCM_COM_Opt_Adhesion_In_Cons_W34/1
  BCM_COM_PROC_P20/576 -> Prb_MinimalTargetDecel/1  "Prb_MinimalTargetDecel_4_BCMA"
  BCM_COM_PROC_P20/575 -> Prb_TargetSpeedDelta/1  "Prb_TargetSpeedDelta_4_BCMA"
  BCM_COM_PROC_P20/572 -> Prb_TransitionGammaIncrease/1  "Prb_TransitionGammaIncrease_4_BCMA"
  BCM_COM_PROC_P20/531 -> Prb_CommandedPressureTheorCurrent/1  "Prb_CommandedPressureTheorCurrent_4_BCMA"
  BCM_COM_PROC_P20/571 -> Prb_TransitionGammaDecrease/1  "Prb_TransitionGammaDecrease_4_BCMA"
  BCM_COM_PROC_P20/515 -> v_BCM_COM_ERU_in/1  "v_BCM_COM_ERU_in_1_BCMA"
  BCM_COM_PROC_P20/569 -> Prb_ForcedSmallSlipStep/1  "Prb_ForcedSmallSlipStep_4_BCMA"
  BCM_COM_PROC_P20/796 -> v_BCM_COM_UF_DFCS_A_VALWOW_2_RX/1  "v_BCM_COM_UF_DFCS_A_VALWOW_2_RX_1_BCMA"
  BCM_COM_PROC_P20/459 -> Prb_UnlimitedReferenceSpeed_3 (2)/1  "Prb_UnlimitedReferenceSpeed_3_2_BCMA"
  BCM_COM_PROC_P20/341 -> V_BCM_COM_A429_Global_Wheel_Spd/1
  BCM_COM_PROC_P20/568 -> Prb_NaturalSmallSlipStep/1  "Prb_NaturalSmallSlipStep_4_BCMA"
  BCM_COM_PROC_P20/566 -> Prb_NaturalBigSlipStep/1  "Prb_NaturalBigSlipStep_4_BCMA"
  BCM_COM_PROC_P20/564 -> Prb_BigSlipStepAuthorize/1  "Prb_BigSlipStepAuthorize_4_BCMA"
  BCM_COM_PROC_P20/215 -> V_BCM_COM_Park_Sw_Cmd_Cons/1
  BCM_COM_PROC_P20/125 -> V_BCM_COM_Target_Speed_Out_W34/1
  BCM_COM_PROC_P20/563 -> Prb_TransitionBigGammaStep/1  "Prb_TransitionBigGammaStep_4_BCMA"
  BCM_COM_PROC_P20/559 -> Prb_TransitionBigSlipWatchDog/1  "Prb_TransitionBigSlipWatchDog_4_BCMA"
  BCM_COM_PROC_P20/557 -> Prb_ForcedBigSlipWatchDog/1  "Prb_ForcedBigSlipWatchDog_4_BCMA"
  BCM_COM_PROC_P20/303 -> V_BCM_COM_A429_Park_Brake_ON/1
  V_BCM_COM_LNLG_Tire_Press_Unconf_Flt/1 -> DTC176/1
  BCM_COM_PROC_P20/555 -> Prb_FastTrigCondition/1  "Prb_FastTrigCondition_4_BCMA"
  BCM_COM_PROC_P20/554 -> Prb_SlowStateCondition/1  "Prb_SlowStateCondition_4_BCMA"
  BCM_COM_PROC_P20/107 -> V_BCM_COM_Hyd_A_Press_Cons_Val/1
  BCM_COM_PROC_P20/553 -> Prb_FastStateCondition/1  "Prb_FastStateCondition_4_BCMA"
  BCM_COM_PROC_P20/551 -> Prb_FastMonitoringCondition/1  "Prb_FastMonitoringCondition_4_BCMA"
  BCM_COM_PROC_P20/245 -> V_BCM_COM_A429_SSM_DFCS_Label_105/1
  BCM_COM_PROC_P20/550 -> Prb_StateSignalValidityCondition/1  "Prb_StateSignalValidityCondition_4_BCMA"
  BCM_COM_PROC_P20/395 -> V_BCM_COM_ETH_FB_LG_LEVER_FAIL/1
  BCM_COM_PROC_P20/548 -> Prb_TransitionBrakingInit/1  "Prb_TransitionBrakingInit_4_BCMA"
  BCM_COM_PROC_P20/547 -> Prb_ResearchModeCondition/1  "Prb_ResearchModeCondition_4_BCMA"
  BCM_COM_PROC_P20/546 -> Prb_BigSlipWatchDogTargetDecel/1  "Prb_BigSlipWatchDogTargetDecel_4_BCMA"
  BCM_COM_PROC_P20/544 -> Prb_DecelerationDecrement/1  "Prb_DecelerationDecrement_4_BCMA"
  BCM_COM_PROC_P20/223 -> V_BCM_COM_RNLG_Tire_Press_Cons_Val/1
  BCM_COM_PROC_P20/523 -> v_BCM_COM_PB_in/1  "v_BCM_COM_PB_in_1_BCMA"
  BCM_COM_PROC_P20/121 -> V_BCM_COM_Small_Slip_Trig_Out_W34/1
  V_BCM_COM_SV_Current_Readback_Val/1 -> DTC215/1
  BCM_COM_PROC_P20/535 -> Prb_Adhesion/1  "Prb_Adhesion_4_BCMA"
  V_BCM_COM_MP_MAINT_MODE_CMD_28V_Acq/1 -> DTC172/1
  BCM_COM_PROC_P20/533 -> Prb_AsLowPassTheorCurrent/1  "Prb_AsLowPassTheorCurrent_4_BCMA"
  BCM_COM_PROC_P20/90 -> V_BCM_COM_Alt_Sw_Cmd_Cons_Val/1
  BCM_COM_PROC_P20/532 -> Prb_AsLowPassTheorPressure/1  "Prb_AsLowPassTheorPressure_4_BCMA"
  BCM_COM_PROC_P20/530 -> Prb_TheorCommandedPressure/1  "Prb_TheorCommandedPressure_4_BCMA"
  BCM_COM_PROC_P20/529 -> Prb_AutomateFilteredPressure/1  "Prb_AutomateFilteredPressure_4_BCMA"
  BCM_COM_PROC_P20/526 -> v_BCM_COM_Norm_FT_Reset_Cond/1  "v_BCM_COM_Norm_FT_Reset_Cond_1_BCMA"
  BCM_COM_PROC_P20/11 -> V_BCM_COM_AC_Long_Accel_Cons/1
  BCM_COM_PROC_P20/807 -> v_BCM_COM_CF_DFCS_B_LMLGWOW_1_RX/1  "v_BCM_COM_CF_DFCS_B_LMLGWOW_1_RX_1_BCMA"
  BCM_COM_PROC_P20/524 -> v_BCM_COM_PB_out/1  "v_BCM_COM_PB_out_1_BCMA"
  BCM_COM_PROC_P20/522 -> v_BCM_COM_FTB_out/1  "v_BCM_COM_FTB_out_1_BCMA"
  BCM_COM_PROC_P20/521 -> v_BCM_COM_FTB_in/1  "v_BCM_COM_FTB_in_1_BCMA"
  BCM_COM_PROC_P20/165 -> V_BCM_COM_DFCS_A_LMLG_WOWs_Val/1
  BCM_COM_PROC_P20/520 -> v_BCM_COM_MTB_out/1  "v_BCM_COM_MTB_out_1_BCMA"
  BCM_COM_PROC_P20/68 -> V_BCM_COM_Braking_Norm_FT_Seq/1
  BCM_COM_PROC_P20/518 -> v_BCM_COM_LGRB_out/1  "v_BCM_COM_LGRB_out_1_BCMA"
  BCM_COM_PROC_P20/517 -> v_BCM_COM_LGRB_in/1  "v_BCM_COM_LGRB_in_1_BCMA"
  BCM_COM_PROC_P20/516 -> v_BCM_COM_ERU_out/1  "v_BCM_COM_ERU_out_1_BCMA"
  BCM_COM_PROC_P20/511 -> Prb_Previous_WheelSpeedState (4)/1  "Prb_Previous_WheelSpeedState_1_BCMA"
  BCM_COM_PROC_P20/509 -> Prb_RightIsInvalid/1  "Prb_RightIsInvalid_1_BCMA"
  BCM_COM_PROC_P20/508 -> Prb_LeftIsInvalid/1  "Prb_LeftIsInvalid_1_BCMA"
  BCM_COM_PROC_P20/435 -> Prb_HydroplanePhaseInit (1)/1  "Prb_HydroplanePhaseInit_4_BCMA"
  BCM_COM_PROC_P20/862 -> PRB_BrakeFilled (1)/1  "PRB_BrakeFilled_1_BCMA"
  BCM_COM_PROC_P20/507 -> Prb_RightWheelSpeed/1  "Prb_RightWheelSpeed_1_BCMA"
  BCM_COM_PROC_P20/127 -> V_BCM_COM_Target_Decel_Out_W34/1
  BCM_COM_PROC_P20/506 -> Prb_LeftWheelSpeed/1  "Prb_LeftWheelSpeed_1_BCMA"
  BCM_COM_PROC_P20/421 -> Prb_RefSpeedLowLimit/1  "Prb_RefSpeedLowLimit_9_BCMA"
  BCM_COM_PROC_P20/67 -> V_BCM_COM_Brkg_Norm_FT_Cond/1
  BCM_COM_PROC_P20/505 -> Prb_BrakingPhaseAcceleration (4)/1  "Prb_BrakingPhaseAcceleration_1_BCMA"
  BCM_COM_PROC_P20/504 -> Prb_OnGndAfterHydroAccel (4)/1  "Prb_OnGndAfterHydroAccel_1_BCMA"
  BCM_COM_PROC_P20/462 -> Prb_UnlimitedReferenceSpeed_4 (2)/1  "Prb_UnlimitedReferenceSpeed_4_2_BCMA"
  BCM_COM_PROC_P20/139 -> V_BCM_COM_Target_Speed_In_Cons_W34/1
  BCM_COM_PROC_P20/503 -> Prb_RefSpeedLowLimit (8)/1  "Prb_RefSpeedLowLimit_1_BCMA"
  V_BCM_COM_CF_LH_SV_SC/1 -> DTC197/1
  BCM_COM_PROC_P20/499 -> Prb_HydroplanePhaseInit (4)/1  "Prb_HydroplanePhaseInit_1_BCMA"
  BCM_COM_PROC_P20/498 -> Prb_HydroplaneAccelProblem (4)/1  "Prb_HydroplaneAccelProblem_1_BCMA"
  BCM_COM_PROC_P20/168 -> V_BCM_COM_DFCS_A_WOWs_Val_Val/1
  BCM_COM_PROC_P20/497 -> Prb_WheelSpunUpCond/1  "Prb_WheelSpunUpCond_1_BCMA"
  BCM_COM_PROC_P20/496 -> Prb_HydroplaneTransition (4)/1  "Prb_HydroplaneTransition_1_BCMA"
  BCM_COM_PROC_P20/495 -> Prb_OnGroundAfterHydroplaneTransition/1  "Prb_OnGroundAfterHydroplaneTransition_1_BCMA"
  BCM_COM_PROC_P20/271 -> V_BCM_COM_A429_RNLG_Tire_Press_Sensor_Fail/1
  BCM_COM_PROC_P20/701 -> Prb_AdhesionOpt (3)/1  "Prb_AdhesionOpt_1_BCMA"
  BCM_COM_PROC_P20/494 -> v_BCM_COM_SELV_High_Side_Cmd_Order_Prev/1  "v_BCM_COM_SELV_High_Side_Cmd_Order_Prev_1_BCMA"
  BCM_COM_PROC_P20/493 -> v_BCM_COM_Takeoff_Phase/1  "v_BCM_COM_Takeoff_Phase_1_BCMA"
  BCM_COM_PROC_P20/328 -> V_BCM_COM_A429_Maint_Mode_Req_GND/1
  BCM_COM_PROC_P20/492 -> v_BCM_COM_All_Engines_Off/1  "v_BCM_COM_All_Engines_Off_1_BCMA"
  BCM_COM_PROC_P20/222 -> V_BCM_COM_LNLG_Tire_Press_Cons_Val/1
  BCM_COM_PROC_P20/490 -> v_BCM_COM_Braking_State_Norm/1  "v_BCM_COM_Braking_State_Norm_1_BCMA"
  BCM_COM_PROC_P20/365 -> V_BCM_COM_ETH_FB_BCM_FAIL/1
  DTC176/1 -> BCM_COM_PROC_P20/176
  BCM_COM_PROC_P20/771 -> v_BCM_COM_CF_DFCS_A_GND_SPEED_RX/1  "v_BCM_COM_CF_DFCS_A_GND_SPEED_RX_1_BCMA"
  BCM_COM_PROC_P20/489 -> v_BCM_COM_Forced_Act_SELV/1  "v_BCM_COM_Forced_Act_SELV_1_BCMA"
  BCM_COM_PROC_P20/57 -> V_BCM_COM_Global_Reference_Spd/1
  BCM_COM_PROC_P20/488 -> v_BCM_COM_AC_Long_Accel_Filt/1  "v_BCM_COM_AC_Long_Accel_Filt_1_BCMA"
  BCM_COM_PROC_P20/485 -> v_BCM_COM_Spun_Up_Condition_W34/1  "v_BCM_COM_Spun_Up_Condition_W34_1_BCMA"
  BCM_COM_PROC_P20/285 -> V_BCM_COM_A429_SV_Current_Readback/1
  BCM_COM_PROC_P20/482 -> Prb_Previous_WheelSpeedState (3)/1  "Prb_Previous_WheelSpeedState_2_BCMA"
  BCM_COM_PROC_P20/694 -> Prb_AutomateFilteredPressure (3)/1  "Prb_AutomateFilteredPressure_1_BCMA"
  BCM_COM_PROC_P20/310 -> V_BCM_COM_A429_Avionics_Comm_Fail_RX/1
  BCM_COM_PROC_P20/481 -> Prb_WheelSpeedState (3)/1  "Prb_WheelSpeedState_2_BCMA"
  BCM_COM_PROC_P20/860 -> PRB_RateLimitation (1)/1  "PRB_RateLimitation_1_BCMA"
  BCM_COM_PROC_P20/480 -> Prb_UnlimitedReferenceSpeed_4 (3)/1  "Prb_UnlimitedReferenceSpeed_4_1_BCMA"
  BCM_COM_PROC_P20/209 -> V_BCM_COM_ACCU_Pressure_State/1
  BCM_COM_PROC_P20/479 -> Prb_BrakingPhaseAcceleration (3)/1  "Prb_BrakingPhaseAcceleration_2_BCMA"
  BCM_COM_PROC_P20/673 -> Prb_TransitionBigGammaStep (2)/1  "Prb_TransitionBigGammaStep_2_BCMA"
  BCM_COM_PROC_P20/478 -> Prb_OnGndAfterHydroAccel (3)/1  "Prb_OnGndAfterHydroAccel_2_BCMA"
  BCM_COM_PROC_P20/276 -> V_BCM_COM_A429_TPIS_Fail/1
  BCM_COM_PROC_P20/45 -> V_BCM_COM_LMLG_Dnlk_State_Val/1
  BCM_COM_PROC_P20/477 -> Prb_UnlimitedReferenceSpeed_3 (3)/1  "Prb_UnlimitedReferenceSpeed_3_1_BCMA"
  BCM_COM_PROC_P20/400 -> V_BCM_COM_ETH_FB_LH_OUT_TACHO_FAIL/1
  BCM_COM_PROC_P20/476 -> Prb_RefSpeedLowLimit (7)/1  "Prb_RefSpeedLowLimit_2_BCMA"
  BCM_COM_PROC_P20/368 -> V_BCM_COM_ETH_FB_MAINT_MODE_DIS/1
  BCM_COM_PROC_P20/700 -> Prb_Adhesion (3)/1  "Prb_Adhesion_1_BCMA"
  BCM_COM_PROC_P20/475 -> Prb_RefSpeedLowLimit (6)/1  "Prb_RefSpeedLowLimit_3_BCMA"
  BCM_COM_PROC_P20/474 -> Prb_Hydroplane_PreviousSpeed (3)/1  "Prb_Hydroplane_PreviousSpeed_1_BCMA"
  BCM_COM_PROC_P20/380 -> V_BCM_COM_ETH_FB_BSELV_JCL/1
  BCM_COM_PROC_P20/797 -> v_BCM_COM_UF_DFCS_A_VALWOW_1_RX/1  "v_BCM_COM_UF_DFCS_A_VALWOW_1_RX_1_BCMA"
  BCM_COM_PROC_P20/472 -> Prb_HydroplaneAccelCond (3)/1  "Prb_HydroplaneAccelCond_2_BCMA"
  BCM_COM_PROC_P20/446 -> Prb_Previous_WheelSpeedState (1)/1  "Prb_Previous_WheelSpeedState_4_BCMA"
  BCM_COM_PROC_P20/169 -> V_BCM_COM_DFCS_B_LMLG_WOWs_Val/1
  BCM_COM_PROC_P20/39 -> V_BCM_COM_LG_Lever_Up_Conf/1
  BCM_COM_PROC_P20/469 -> Prb_HydroplaneCondition (3)/1  "Prb_HydroplaneCondition_1_BCMA"
  BCM_COM_PROC_P20/468 -> Prb_SpunUpCondition (3)/1  "Prb_SpunUpCondition_1_BCMA"
  BCM_COM_PROC_P20/466 -> Prb_HydroplaneTransition (3)/1  "Prb_HydroplaneTransition_2_BCMA"
  BCM_COM_PROC_P20/464 -> Prb_Previous_WheelSpeedState (2)/1  "Prb_Previous_WheelSpeedState_3_BCMA"
  BCM_COM_PROC_P20/460 -> Prb_OnGndAfterHydroAccel (2)/1  "Prb_OnGndAfterHydroAccel_3_BCMA"
  BCM_COM_PROC_P20/403 -> V_BCM_COM_ETH_FB_RH_OUT_TACHO_FAIL/1
  BCM_COM_PROC_P20/31 -> V_BCM_COM_NLG_On_Gnd_State_Val/1
  BCM_COM_PROC_P20/458 -> Prb_RefSpeedLowLimit (5)/1  "Prb_RefSpeedLowLimit_4_BCMA"
  BCM_COM_PROC_P20/457 -> Prb_RefSpeedLowLimit (4)/1  "Prb_RefSpeedLowLimit_5_BCMA"
  BCM_COM_PROC_P20/456 -> Prb_Hydroplane_PreviousSpeed (2)/1  "Prb_Hydroplane_PreviousSpeed_2_BCMA"
  BCM_COM_PROC_P20/22 -> V_BCM_COM_RMLG_WOWs_Cons_Val/1
  BCM_COM_PROC_P20/454 -> Prb_HydroplaneAccelCond (2)/1  "Prb_HydroplaneAccelCond_3_BCMA"
  BCM_COM_PROC_P20/453 -> Prb_HydroplanePhaseInit (2)/1  "Prb_HydroplanePhaseInit_3_BCMA"
  BCM_COM_PROC_P20/452 -> Prb_HydroplaneAccelProblem (2)/1  "Prb_HydroplaneAccelProblem_3_BCMA"
  BCM_COM_PROC_P20/450 -> Prb_SpunUpCondition (2)/1  "Prb_SpunUpCondition_2_BCMA"
  BCM_COM_PROC_P20/260 -> V_BCM_COM_A429_LH_Brake_Temp_Sensor_Fail/1
  BCM_COM_PROC_P20/447 -> Prb_Previous_ReferenceSpeed (1)/1  "Prb_Previous_ReferenceSpeed_3_BCMA"
  BCM_COM_PROC_P20/21 -> V_BCM_COM_RMLG_WOWs_Cons/1
  BCM_COM_PROC_P20/445 -> Prb_WheelSpeedState (1)/1  "Prb_WheelSpeedState_4_BCMA"
  BCM_COM_PROC_P20/443 -> Prb_BrakingPhaseAcceleration (1)/1  "Prb_BrakingPhaseAcceleration_4_BCMA"
  BCM_COM_PROC_P20/440 -> Prb_RefSpeedLowLimit (3)/1  "Prb_RefSpeedLowLimit_6_BCMA"
  BCM_COM_PROC_P20/438 -> Prb_Hydroplane_PreviousSpeed (1)/1  "Prb_Hydroplane_PreviousSpeed_3_BCMA"
  BCM_COM_PROC_P20/430 -> Prb_HydroplaneTransition (1)/1  "Prb_HydroplaneTransition_4_BCMA"
  BCM_COM_PROC_P20/428 -> Prb_Previous_WheelSpeedState/1  "Prb_Previous_WheelSpeedState_5_BCMA"
  BCM_COM_PROC_P20/427 -> Prb_WheelSpeedState/1  "Prb_WheelSpeedState_5_BCMA"
  BCM_COM_PROC_P20/246 -> V_BCM_COM_A429_Wheel_Speed_W12/1
  BCM_COM_PROC_P20/423 -> Prb_UnlimitedReferenceSpeed_3/1  "Prb_UnlimitedReferenceSpeed_3_4_BCMA"
  BCM_COM_PROC_P20/420 -> Prb_Hydroplane_PreviousSpeed/1  "Prb_Hydroplane_PreviousSpeed_4_BCMA"
  BCM_COM_PROC_P20/417 -> Prb_HydroplanePhaseInit/1  "Prb_HydroplanePhaseInit_5_BCMA"
  BCM_COM_PROC_P20/355 -> V_BCM_COM_ETH_DISPATCH_SW_ON/1
  BCM_COM_PROC_P20/416 -> Prb_HydroplaneAccelProblem/1  "Prb_HydroplaneAccelProblem_5_BCMA"
  BCM_COM_PROC_P20/413 -> Prb_OnGroundAfterHydroTransition/1  "Prb_OnGroundAfterHydroTransition_4_BCMA"
  BCM_COM_PROC_P20/317 -> V_BCM_COM_A429_DFCS_B_Comm_Fail_RX/1
  BCM_COM_PROC_P20/408 -> V_BCM_COM_ETH_TT_result_significant/1
  BCM_COM_PROC_P20/405 -> V_BCM_COM_ETH_TT_rejection_cause/1
  BCM_COM_PROC_P20/622 -> Prb_TransitionBigSlipStep (1)/1  "Prb_TransitionBigSlipStep_3_BCMA"
  BCM_COM_PROC_P20/404 -> V_BCM_COM_ETH_TT_in_progress_id/1
  BCM_COM_PROC_P20/399 -> V_BCM_COM_ETH_Invalid_Config/1
  BCM_COM_PROC_P20/398 -> V_BCM_COM_ETH_TARGET_HW_ID/1
  BCM_COM_PROC_P20/394 -> V_BCM_COM_ETH_Braking_Alt_FT_Seq/1
  BCM_COM_PROC_P20/392 -> V_BCM_COM_ETH_Braking_Mode/1
  BCM_COM_PROC_P20/387 -> V_BCM_COM_ETH_FB_RH_SV_CMD_FAIL/1
  BCM_COM_PROC_P20/385 -> V_BCM_COM_ETH_FB_LH_SV_JOP/1
  BCM_COM_PROC_P20/383 -> V_BCM_COM_ETH_FB_LH_SV_CMD_FAIL/1
  BCM_COM_PROC_P20/379 -> V_BCM_COM_ETH_FB_BSELV_CMD_FAIL/1
  BCM_COM_PROC_P20/376 -> V_BCM_COM_ETH_FB_HYD_B_LOW_PRESS/1
  BCM_COM_PROC_P20/374 -> V_BCM_COM_ETH_FB_INHIB_FAIL/1
  BCM_COM_PROC_P20/373 -> V_BCM_COM_ETH_FB_DBCU_BRK_ORDER_FAIL/1
  BCM_COM_PROC_P20/370 -> V_BCM_COM_ETH_FB_BCM_DBCU_MODE_DIS/1
  BCM_COM_PROC_P20/369 -> V_BCM_COM_ETH_FB_PARK_BRK_STATUS_DIS/1
  BCM_COM_PROC_P20/362 -> V_BCM_COM_ETH_RH_SV_Current_Order/1
  BCM_COM_PROC_P20/473 -> Prb_HydroplaneAcceleration (3)/1  "Prb_HydroplaneAcceleration_2_BCMA"
  BCM_COM_PROC_P20/356 -> V_BCM_COM_ETH_LH_DBCU_BRK_CMD_FDBK/1
  BCM_COM_PROC_P20/350 -> V_BCM_COM_ETH_MP_MAINT_MODE_CMD_GND/1
  BCM_COM_PROC_P20/346 -> V_BCM_COM_ETH_LMLG_Dnlk/1
  BCM_COM_PROC_P20/344 -> V_BCM_COM_ETH_ENG1_RUNNING/1
  BCM_COM_PROC_P20/339 -> V_BCM_COM_A429_DBCU_Alt_Mode/1
  BCM_COM_PROC_P20/333 -> V_BCM_COM_A429_BCM_Fail/1
  BCM_COM_PROC_P20/329 -> V_BCM_COM_A429_Maint_Mode_Req_28V/1
  BCM_COM_PROC_P20/322 -> V_BCM_COM_A429_Pinprog_3/1
  BCM_COM_PROC_P20/321 -> V_BCM_COM_A429_Pinprog_2/1
  BCM_COM_PROC_P20/320 -> V_BCM_COM_A429_Pinprog_1/1
  BCM_COM_PROC_P20/442 -> Prb_OnGndAfterHydroAccel (1)/1  "Prb_OnGndAfterHydroAccel_4_BCMA"
  BCM_COM_PROC_P20/311 -> V_BCM_COM_A429_DFCS_Decel_Law_Inhib/1
  BCM_COM_PROC_P20/308 -> V_BCM_COM_A429_Brk_Residual_Press/1
  BCM_COM_PROC_P20/305 -> V_BCM_COM_A429_Norm_FT_In_Progress/1
  BCM_COM_PROC_P20/301 -> V_BCM_COM_A429_SSM_Avionics_Label_034/1
  BCM_COM_PROC_P20/299 -> V_BCM_COM_A429_SSM_DFCS_Label_106/1
  BCM_COM_PROC_P20/298 -> V_BCM_COM_A429_SSM_Avionics_Label_037/1
  BCM_COM_PROC_P20/293 -> V_BCM_COM_A429_SELV_Disc_Sts_Rdbk/1
  BCM_COM_PROC_P20/471 -> Prb_HydroplanePhaseInit (3)/1  "Prb_HydroplanePhaseInit_2_BCMA"
  BCM_COM_PROC_P20/290 -> V_BCM_COM_A429_SV_PT_Fail/1
  BCM_COM_PROC_P20/289 -> V_BCM_COM_A429_ACCU_PT_Fail/1
  BCM_COM_PROC_P20/287 -> V_BCM_COM_A429_SV_PT_In_PSI/1
  BCM_COM_PROC_P20/282 -> V_BCM_COM_A429_SSM_Avionics_Label_017/1
  BCM_COM_PROC_P20/713 -> Prb_TransitionBrakingInit (3)/1  "Prb_TransitionBrakingInit_1_BCMA"
  BCM_COM_PROC_P20/279 -> V_BCM_COM_A429_SSM_Avionics_Label_014/1
  BCM_COM_PROC_P20/274 -> V_BCM_COM_A429_RMLG_Inboard_Tire_Press_Sensor_Fail/1
  BCM_COM_PROC_P20/269 -> V_BCM_COM_A429_RMLG_Outboard_Tire_Press/1
  BCM_COM_PROC_P20/261 -> V_BCM_COM_A429_RH_Brake_Temp_Sensor_Fail/1
  BCM_COM_PROC_P20/257 -> V_BCM_COM_A429_SSM_DFCS_Label_104/1
  BCM_COM_PROC_P20/437 -> Prb_HydroplaneAcceleration (1)/1  "Prb_HydroplaneAcceleration_4_BCMA"
  BCM_COM_PROC_P20/251 -> V_BCM_COM_A429_SSM_Avionics_Label_002/1
  BCM_COM_PROC_P20/249 -> V_BCM_COM_A429_TACHO_Fail_W34/1
  BCM_COM_PROC_P20/242 -> V_BCM_COM_A429_SSM_Avionics_Label_042/1
  BCM_COM_PROC_P20/424 -> Prb_OnGndAfterHydroAccel/1  "Prb_OnGndAfterHydroAccel_5_BCMA"
  BCM_COM_PROC_P20/240 -> V_BCM_COM_A429_SSM_Avionics_Label_040/1
  BCM_COM_PROC_P20/237 -> V_BCM_COM_A429_SSM_Avionics_Label_031/1
  BCM_COM_PROC_P20/788 -> v_BCM_COM_CF_DFCS_A_RMLGWOW_2_RX/1  "v_BCM_COM_CF_DFCS_A_RMLGWOW_2_RX_1_BCMA"
  BCM_COM_PROC_P20/232 -> V_BCM_COM_A429_SSM_Avionics_Label_005/1
  BCM_COM_PROC_P20/227 -> V_BCM_COM_LMLG_Inboard_Tire_Press_Cons_Val/1
  BCM_COM_PROC_P20/221 -> V_BCM_COM_RNLG_Tire_Press_Cons/1
  BCM_COM_PROC_P20/218 -> V_BCM_COM_MP_MAINT_MODE_CMD_GND_Conf/1
  BCM_COM_PROC_P20/214 -> V_BCM_COM_BCP_PARK_OFF_SW_CMD_Conf/1
  BCM_COM_PROC_P20/213 -> V_BCM_COM_RH_Brake_Temp_Cons_Val/1
  BCM_COM_PROC_P20/627 -> Prb_TransitionGammaIncrease (1)/1  "Prb_TransitionGammaIncrease_3_BCMA"
  BCM_COM_PROC_P20/212 -> V_BCM_COM_RH_Brake_Temp_Cons/1
  BCM_COM_PROC_P20/203 -> V_BCM_COM_DBCU_FAILED_Cons/1
  BCM_COM_PROC_P20/198 -> V_BCM_COM_DBCU_DISPATCH_SW_ON_Cons_Val/1
  BCM_COM_PROC_P20/191 -> V_BCM_COM_LH_DBCU_BRK_CMD_FDBK_Conf/1
  BCM_COM_PROC_P20/187 -> V_BCM_COM_UTC_Time_Seconds_Cons/1
  BCM_COM_PROC_P20/185 -> V_BCM_COM_UTC_Time_Minutes_Cons/1
  BCM_COM_PROC_P20/769 -> v_BCM_COM_UF_DFCS_A_RH_BRK_CMD_RX/1  "v_BCM_COM_UF_DFCS_A_RH_BRK_CMD_RX_1_BCMA"
  BCM_COM_PROC_P20/184 -> V_BCM_COM_UTC_Time_Hours_Cons_Val/1
  BCM_COM_PROC_P20/182 -> V_BCM_COM_DFCS_B_TLA_Above_Idle_Val/1
  BCM_COM_PROC_P20/176 -> V_BCM_COM_DFCS_B_RH_Braking_Cmd_Val/1
  BCM_COM_PROC_P20/175 -> V_BCM_COM_DFCS_B_LH_Braking_Cmd_Val/1
  BCM_COM_PROC_P20/173 -> V_BCM_COM_DFCS_A_LH_Braking_Cmd_Val/1
  BCM_COM_PROC_P20/170 -> V_BCM_COM_DFCS_B_RMLG_WOWs_Val/1
  BCM_COM_PROC_P20/167 -> V_BCM_COM_DFCS_A_NLG_WOWs_Val/1
  BCM_COM_PROC_P20/164 -> V_BCM_COM_DFCS_B_AC_Pitch_Angle_Val/1
  BCM_COM_PROC_P20/160 -> V_BCM_COM_DFCS_A_Decel_Law_Inhib_Val/1
  BCM_COM_PROC_P20/158 -> V_BCM_COM_DFCS_A_AC_Long_Accel_Val/1
  BCM_COM_PROC_P20/156 -> V_BCM_COM_Hyd_B_Press_Unconf_Flt/1
  BCM_COM_PROC_P20/153 -> V_BCM_COM_Hyd_A_Press_Conf_Flt/1
  BCM_COM_PROC_P20/152 -> V_BCM_COM_Engine_Running_Unconf_Flt/1
  BCM_COM_PROC_P20/150 -> V_BCM_COM_DBCU_Inhibition_Order_From_Opp_BCM_Cons_Val/1
  BCM_COM_PROC_P20/149 -> V_BCM_COM_DBCU_Inhibition_Order_From_Opp_BCM_Cons/1
  BCM_COM_PROC_P20/148 -> V_BCM_COM_CCDL_Data_From_Opp_BCM_Val/1
  BCM_COM_PROC_P20/147 -> V_BCM_COM_Big_Slip_Trig_In_Cons_W34/1
  BCM_COM_PROC_P20/142 -> V_BCM_COM_Big_Gamma_Trig_In_Cons_W12/1
  BCM_COM_PROC_P20/141 -> V_BCM_COM_Big_Slip_WD_Trig_In_Cons_W34/1
  BCM_COM_PROC_P20/140 -> V_BCM_COM_Big_Slip_WD_Trig_In_Cons_W12/1
  BCM_COM_PROC_P20/858 -> PRB_RateLimitationActivation/1  "PRB_RateLimitationActivation_2_BCMA"
  BCM_COM_PROC_P20/138 -> V_BCM_COM_Target_Speed_In_Cons_W12/1
  BCM_COM_PROC_P20/136 -> V_BCM_COM_Opt_Adhesion_In_Cons_W12/1
  BCM_COM_PROC_P20/470 -> Prb_HydroplaneAccelProblem (3)/1  "Prb_HydroplaneAccelProblem_2_BCMA"
  BCM_COM_PROC_P20/134 -> V_BCM_COM_Adhesion_In_Cons_W12/1
  BCM_COM_PROC_P20/131 -> V_BCM_COM_Opt_Adhesion_Out_W34/1
  BCM_COM_PROC_P20/128 -> V_BCM_COM_Adhesion_Out_W12/1
  BCM_COM_PROC_P20/124 -> V_BCM_COM_Target_Speed_Out_W12/1
  BCM_COM_PROC_P20/123 -> V_BCM_COM_Automate_State_W34/1
  BCM_COM_PROC_P20/724 -> Prb_TransitionBigSlipWatchDog (3)/1  "Prb_TransitionBigSlipWatchDog_1_BCMA"
  BCM_COM_PROC_P20/117 -> V_BCM_COM_Big_Slip_Trig_Out_W34/1
  BCM_COM_PROC_P20/115 -> V_BCM_COM_Big_Gamma_Trig_Out_W34/1
  BCM_COM_PROC_P20/112 -> V_BCM_COM_Wheel_Control_Speed_W12/1
  BCM_COM_PROC_P20/110 -> V_BCM_COM_Hyd_B_Press_State/1
  BCM_COM_PROC_P20/109 -> V_BCM_COM_Hyd_A_Press_State/1
  BCM_COM_PROC_P20/106 -> V_BCM_COM_Hyd_B_Press_Cons/1
  BCM_COM_PROC_P20/104 -> V_BCM_COM_PBSELV_State_Cons_Val/1
  BCM_COM_PROC_P20/102 -> V_BCM_COM_PBSELV_ON_POS_Conf/1
  BCM_COM_PROC_P20/101 -> V_BCM_COM_Press_Cmd_Rate_Lim/1
  BCM_COM_PROC_P20/96 -> V_BCM_COM_Norm_Brkg_Availability/1
  BCM_COM_PROC_P20/95 -> V_BCM_COM_Braking_State/1
  BCM_COM_PROC_P20/93 -> V_BCM_COM_MP_BCMA_Alt_Disp_Sw_Conf/1
  BCM_COM_PROC_P20/91 -> V_BCM_COM_Disp_Sw_Cmd_Cons/1
  BCM_COM_PROC_P20/89 -> V_BCM_COM_Alt_Sw_Cmd_Cons/1
  BCM_COM_PROC_P20/88 -> V_BCM_COM_BCM_Validity/1
  BCM_COM_PROC_P20/85 -> V_BCM_COM_Brkg_SELV_High_Side_FT_Cmd_Order/1
  BCM_COM_PROC_P20/83 -> V_BCM_COM_LH_Eng_Run_Press_Cmd/1
  BCM_COM_PROC_P20/82 -> V_BCM_COM_RH_Ret_Brkg_Press_Cmd/1
  BCM_COM_PROC_P20/80 -> V_BCM_COM_RH_FT_Press_Cmd/1
  BCM_COM_PROC_P20/79 -> V_BCM_COM_LH_FT_Press_Cmd/1
  BCM_COM_PROC_P20/74 -> V_BCM_COM_Brkg_Alt_FT_Cond/1
  BCM_COM_PROC_P20/72 -> V_BCM_COM_Abort_Alt_FT_Cond/1
  BCM_COM_PROC_P20/828 -> v_BCM_COM_UF_DFCS_B_LMLGWOW_3_RX/1  "v_BCM_COM_UF_DFCS_B_LMLGWOW_3_RX_1_BCMA"
  BCM_COM_PROC_P20/70 -> V_BCM_COM_Brkg_Alt_FT_Prog_Sts/1
  BCM_COM_PROC_P20/69 -> V_BCM_COM_Abort_Norm_FT_Cond/1
  BCM_COM_PROC_P20/66 -> V_BCM_COM_Brkg_Norm_FT_Prog_Sts/1
  BCM_COM_PROC_P20/63 -> V_BCM_COM_Braking_Mode/1
  BCM_COM_PROC_P20/62 -> V_BCM_COM_AC_Flight_Phase/1
  BCM_COM_PROC_P20/314 -> V_BCM_COM_A429_DFCS_LH_Brk_Pdl_Ord_Fail/1
  BCM_COM_PROC_P20/60 -> V_BCM_COM_RMLG_Global_Wheel_Spd/1
  BCM_COM_PROC_P20/59 -> V_BCM_COM_LMLG_Global_Wheel_Spd/1
  BCM_COM_PROC_P20/58 -> V_BCM_COM_Global_Wheel_Spd/1
  BCM_COM_PROC_P20/54 -> V_BCM_COM_LH_Regular_Brkg_Press_Cmd/1
  BCM_COM_PROC_P20/343 -> V_BCM_COM_ETH_HYD_B_PRESS/1
  BCM_COM_PROC_P20/52 -> V_BCM_COM_LH_Braking_Cmd_State/1
  BCM_COM_PROC_P20/51 -> V_BCM_COM_Engine_State_Val/1
  BCM_COM_PROC_P20/50 -> V_BCM_COM_Engine_State/1
  BCM_COM_PROC_P20/48 -> V_BCM_COM_SELV_High_Side_Cmd_Order/1
  BCM_COM_PROC_P20/47 -> V_BCM_COM_RMLG_Dnlk_State_Val/1
  BCM_COM_PROC_P20/44 -> V_BCM_COM_LMLG_Downlock_State/1
  BCM_COM_PROC_P20/43 -> V_BCM_COM_RMLG_Downlock_Conf/1
  BCM_COM_PROC_P20/42 -> V_BCM_COM_LMLG_Downlock_Conf/1
  BCM_COM_PROC_P20/40 -> V_BCM_COM_LG_Lever_State_Cons/1
  BCM_COM_PROC_P20/38 -> V_BCM_COM_TLA_State_Cons_Val/1
  BCM_COM_PROC_P20/37 -> V_BCM_COM_TLA_State_Cons/1
  BCM_COM_PROC_P20/35 -> V_BCM_COM_Decel_Law_Inhib_Cons/1
  BCM_COM_PROC_P20/233 -> V_BCM_COM_A429_SSM_Avionics_Label_006/1
  BCM_COM_PROC_P20/30 -> V_BCM_COM_NLG_On_Gnd_State/1
  BCM_COM_PROC_P20/623 -> Prb_NaturalSmallSlipStep (1)/1  "Prb_NaturalSmallSlipStep_3_BCMA"
  BCM_COM_PROC_P20/29 -> V_BCM_COM_MLG_On_Gnd_State/1
  BCM_COM_PROC_P20/28 -> V_BCM_COM_RMLG_On_Gnd_State_Val/1
  BCM_COM_PROC_P20/25 -> V_BCM_COM_LMLG_On_Gnd_State/1
  BCM_COM_PROC_P20/24 -> V_BCM_COM_NLG_WOWs_Cons_Val/1
  BCM_COM_PROC_P20/23 -> V_BCM_COM_NLG_WOWs_Cons/1
  BCM_COM_PROC_P20/20 -> V_BCM_COM_LMLG_WOWs_Cons_Val/1
  BCM_COM_PROC_P20/19 -> V_BCM_COM_LMLG_WOWs_Cons/1
  BCM_COM_PROC_P20/17 -> V_BCM_COM_DFCS_A_WOWs_Val_Cons/1
  BCM_COM_PROC_P20/599 -> Prb_DecelerationDecrement (1)/1  "Prb_DecelerationDecrement_3_BCMA"
  BCM_COM_PROC_P20/16 -> V_BCM_COM_AC_Pitch_Ang_Cons/1
  BCM_COM_PROC_P20/13 -> V_BCM_COM_AC_Long_Accel_Filt_Corr/1
  BCM_COM_PROC_P20/189 -> V_BCM_COM_DBCU_BRK_ORDER_FAIL_Conf/1
  BCM_COM_PROC_P20/12 -> V_BCM_COM_AC_Long_Accel_Cons_Val/1
  BCM_COM_PROC_P20/10 -> V_BCM_COM_DFCS_B_Long_Accel_Conv/1
  BCM_COM_PROC_P20/8 -> V_BCM_COM_AC_Gnd_Spd_Cons_Val/1
  BCM_COM_PROC_P20/6 -> V_BCM_COM_DFCS_B_Gnd_Spd_Conv/1
  BCM_COM_PROC_P20/87 -> V_BCM_COM_DBCU_Inhib_Order/1
  BCM_COM_PROC_P20/5 -> V_BCM_COM_DFCS_A_Gnd_Spd_Conv/1
  BCM_COM_PROC_P20/4 -> V_BCM_COM_Whl_Ref_Speed_W34/1
  BCM_COM_PROC_P20/3 -> V_BCM_COM_Whl_Spun_Up_State_W34/1
  BCM_COM_PROC_P20/436 -> Prb_HydroplaneAccelCond (1)/1  "Prb_HydroplaneAccelCond_4_BCMA"
  BCM_COM_PROC_P20/728 -> Prb_TransitionBigGammaStep (3)/1  "Prb_TransitionBigGammaStep_1_BCMA"
  BCM_COM_PROC_P20/250 -> V_BCM_COM_A429_SSM_Avionics_Label_001/1
  BCM_COM_PROC_P20/502 -> Prb_PreviousSpeed/1  "Prb_PreviousSpeed_1_BCMA"
  BCM_COM_PROC_P20/624 -> Prb_ForcedSmallSlipStep (1)/1  "Prb_ForcedSmallSlipStep_3_BCMA"
  BCM_COM_PROC_P20/315 -> V_BCM_COM_A429_DFCS_RH_Brk_Pdl_Ord_Fail/1
  BCM_COM_PROC_P20/300 -> V_BCM_COM_A429_SSM_DFCS_Label_107/1
  BCM_COM_PROC_P20/358 -> V_BCM_COM_ETH_DBCU_FAILED/1
  BCM_COM_PROC_P20/61 -> V_BCM_COM_AC_State/1
  BCM_COM_PROC_P20/264 -> V_BCM_COM_A429_LNLG_Tire_Press/1
  BCM_COM_PROC_P20/632 -> Prb_OptimalSpeed (1)/1  "Prb_OptimalSpeed_3_BCMA"
  BCM_COM_PROC_P20/166 -> V_BCM_COM_DFCS_A_RMLG_WOWs_Val/1
  BCM_COM_PROC_P20/53 -> V_BCM_COM_RH_Braking_Cmd_State/1
  BCM_COM_PROC_P20/103 -> V_BCM_COM_PBSELV_State_Cons/1
  BCM_COM_PROC_P20/178 -> V_BCM_COM_DFCS_A_DBCU_Alt_Mode_2_Val/1
  BCM_COM_PROC_P20/327 -> V_BCM_COM_A429_Maint_Mode_Active/1
  BCM_COM_PROC_P20/239 -> V_BCM_COM_A429_SSM_Avionics_Label_033/1
  BCM_COM_PROC_P20/634 -> Prb_WheelSkidSmoothAverage (1)/1  "Prb_WheelSkidSmoothAverage_3_BCMA"
  BCM_COM_PROC_P20/342 -> V_BCM_COM_ETH_HYD_A_PRESS/1
  BCM_COM_PROC_P20/636 -> Prb_StepSize (1)/1  "Prb_StepSize_3_BCMA"
  BCM_COM_PROC_P20/703 -> Prb_BigGammaStepSize (3)/1  "Prb_BigGammaStepSize_1_BCMA"
  BCM_COM_PROC_P20/594 -> Prb_AutomateSofteningFreezingCond (1)/1  "Prb_AutomateSofteningFreezingCond_3_BCMA"
  BCM_COM_PROC_P20/397 -> V_BCM_COM_ETH_FB_RMLG_DWNLOCK_FAIL/1
  BCM_COM_PROC_P20/756 -> v_BCM_COM_UF_ENG_1_RUN_RX/1  "v_BCM_COM_UF_ENG_1_RUN_RX_1_BCMA"
  BCM_COM_PROC_P20/144 -> V_BCM_COM_Small_Slip_Trig_In_Cons_W12/1
  BCM_COM_PROC_P20/277 -> V_BCM_COM_A429_SSM_Avionics_Label_012/1
  BCM_COM_PROC_P20/94 -> V_BCM_COM_BCP_BCM_Alt_Sw_On_Cmd_Conf/1
  BCM_COM_PROC_P20/7 -> V_BCM_COM_AC_Gnd_Spd_Cons/1
  BCM_COM_PROC_P20/783 -> v_BCM_COM_CF_DFCS_A_LMLGWOW_1_RX/1  "v_BCM_COM_CF_DFCS_A_LMLGWOW_1_RX_1_BCMA"
  BCM_COM_PROC_P20/384 -> V_BCM_COM_ETH_FB_LH_SV_JCL/1
  BCM_COM_PROC_P20/143 -> V_BCM_COM_Big_Gamma_Trig_In_Cons_W34/1
  V_BCM_COM_RH_BTS_TEMP_Comp/1 -> DTC229/1
  V_BCM_COM_RH_SV_PT_Conf_Flt/1 -> DTC225/1
  DTC224/1 -> BCM_COM_PROC_P20/224
  BCM_COM_PROC_P20/56 -> V_BCM_COM_Wheels_Global_Spun_Up_Ste/1
  V_BCM_COM_CF_LH_SV_JCL/1 -> DTC223/1
  BCM_COM_PROC_P20/216 -> V_BCM_COM_Park_Sw_Cmd_Cons_Val/1
  DTC222/1 -> BCM_COM_PROC_P20/222
  V_BCM_COM_CF_SV_DRIFT/1 -> DTC222/1
  DTC221/1 -> BCM_COM_PROC_P20/221
  BCM_COM_PROC_P20/162 -> V_BCM_COM_DFCS_B_AC_Gnd_Spd_Val/1
  V_BCM_COM_CF_BSELV_JOP/1 -> DTC220/1
  DTC218/1 -> BCM_COM_PROC_P20/218
  DTC217/1 -> BCM_COM_PROC_P20/217
  V_BCM_COM_CF_BSELV_OC/1 -> DTC217/1
  V_BCM_COM_CF_RH_SV_JCL/1 -> DTC226/1
  BCM_COM_PROC_P20/2 -> V_BCM_COM_Whl_Ref_Speed_W12/1
  V_BCM_COM_SV_Current_Order/1 -> DTC216/1
  V_BCM_COM_DBCU_Conf_Flt/1 -> DTC214/1
  V_BCM_COM_PPRG_i_Acquired/1 -> DTC212/1
  BCM_COM_PROC_P20/510 -> Prb_Previous_GlobalReferenceSpeed/1  "Prb_Previous_GlobalReferenceSpeed_1_BCMA"
  DTC214/1 -> BCM_COM_PROC_P20/214
  V_BCM_COM_DFCS_B_DFCS_BCM_Caps_Val/1 -> DTC211/1
  V_BCM_COM_DFCS_B_Conf_Flt/1 -> DTC210/1
  DTC209/1 -> BCM_COM_PROC_P20/209
  BCM_COM_PROC_P20/193 -> V_BCM_COM_DBCU_FAILED_Conf/1
  V_BCM_COM_DFCS_A_Conf_Flt/1 -> DTC208/1
  V_BCM_COM_Avionics_Conf_Flt/1 -> DTC207/1
  DTC206/1 -> BCM_COM_PROC_P20/206
  V_BCM_COM_CF_RESIDUAL_PRESS/1 -> DTC206/1
  DTC205/1 -> BCM_COM_PROC_P20/205
  V_BCM_COM_CF_PARK_BRK/1 -> DTC205/1
  DTC204/1 -> BCM_COM_PROC_P20/204
  DTC203/1 -> BCM_COM_PROC_P20/203
  V_BCM_COM_CF_SELV_JOP/1 -> DTC203/1
  DTC202/1 -> BCM_COM_PROC_P20/202
  V_BCM_COM_CF_SELV_OC/1 -> DTC202/1
  DTC201/1 -> BCM_COM_PROC_P20/201
  BCM_COM_PROC_P20/119 -> V_BCM_COM_Big_Slip_WD_Trig_Out_W34/1
  DTC200/1 -> BCM_COM_PROC_P20/200
  DTC199/1 -> BCM_COM_PROC_P20/199
  V_BCM_COM_CF_RH_SV_SC/1 -> DTC199/1
  BCM_COM_PROC_P20/366 -> V_BCM_COM_ETH_FB_DFCS_A_RX/1
  DTC196/1 -> BCM_COM_PROC_P20/196
  V_BCM_COM_SELV_High_Side_Readback/1 -> DTC196/1
  V_BCM_COM_LH_BTS_TEMP_Comp/1 -> DTC228/1
  V_BCM_COM_SELV_High_Side_Readback_Val/1 -> DTC195/1
  BCM_COM_PROC_P20/534 -> Prb_SvLowPassTheorCurrent/1  "Prb_SvLowPassTheorCurrent_4_BCMA"
  DTC194/1 -> BCM_COM_PROC_P20/194
  V_BCM_COM_Whl_AS_Activity/1 -> DTC194/1
  DTC228/1 -> BCM_COM_PROC_P20/228
  BCM_COM_PROC_P20/527 -> v_BCM_COM_Alt_FT_Reset_Cond/1  "v_BCM_COM_Alt_FT_Reset_Cond_1_BCMA"
  BCM_COM_PROC_P20/197 -> V_BCM_COM_DBCU_DISPATCH_SW_ON_Cons/1
  DTC193/1 -> BCM_COM_PROC_P20/193
  V_BCM_COM_Whl_AS_Curr_Order/1 -> DTC192/1
  DTC191/1 -> BCM_COM_PROC_P20/191
  V_BCM_COM_RMLG_Outboard_Tire_Press_Unconf_Flt/1 -> DTC191/1
  DTC190/1 -> BCM_COM_PROC_P20/190
  V_BCM_COM_RMLG_Outboard_Tire_Press_Conf_Flt/1 -> DTC190/1
  BCM_COM_PROC_P20/270 -> V_BCM_COM_A429_LNLG_Tire_Press_Sensor_Fail/1
  V_BCM_COM_RMLG_Inboard_Tire_Press_Unconf_Flt/1 -> DTC188/1
  DTC186/1 -> BCM_COM_PROC_P20/186
  V_BCM_COM_RMLG_Inboard_Tire_Press_Acq/1 -> DTC186/1
  DTC185/1 -> BCM_COM_PROC_P20/185
  DTC195/1 -> BCM_COM_PROC_P20/195
  V_BCM_COM_LMLG_Inboard_Tire_Press_Unconf_Flt/1 -> DTC185/1
  BCM_COM_PROC_P20/562 -> Prb_BigGammaThreshold/1  "Prb_BigGammaThreshold_4_BCMA"
  DTC184/1 -> BCM_COM_PROC_P20/184
  DTC182/1 -> BCM_COM_PROC_P20/182
  DTC192/1 -> BCM_COM_PROC_P20/192
  V_BCM_COM_LMLG_Outboard_Tire_Press_Unconf_Flt/1 -> DTC182/1
  BCM_COM_PROC_P20/146 -> V_BCM_COM_Big_Slip_Trig_In_Cons_W12/1
  DTC181/1 -> BCM_COM_PROC_P20/181
  BCM_COM_PROC_P20/132 -> V_BCM_COM_Whl_AS_Adp_Gain_W12/1
  DTC180/1 -> BCM_COM_PROC_P20/180
  V_BCM_COM_LMLG_Outboard_Tire_Press_Acq/1 -> DTC180/1
  DTC179/1 -> BCM_COM_PROC_P20/179
  V_BCM_COM_RNLG_Tire_Press_Unconf_Flt/1 -> DTC179/1
  DTC178/1 -> BCM_COM_PROC_P20/178
  BCM_COM_PROC_P20/129 -> V_BCM_COM_Adhesion_Out_W34/1
  V_BCM_COM_RNLG_Tire_Press_Conf_Flt/1 -> DTC178/1
  DTC177/1 -> BCM_COM_PROC_P20/177
  DTC175/1 -> BCM_COM_PROC_P20/175
  V_BCM_COM_LNLG_Tire_Press_Conf_Flt/1 -> DTC175/1
  DTC173/1 -> BCM_COM_PROC_P20/173
  DTC172/1 -> BCM_COM_PROC_P20/172
  DTC171/1 -> BCM_COM_PROC_P20/171
  V_BCM_COM_BCP_PARK_OFF_SW_CMD_Unconf_Flt/1 -> DTC171/1
  DTC187/1 -> BCM_COM_PROC_P20/187
  BCM_COM_PROC_P20/463 -> Prb_WheelSpeedState (2)/1  "Prb_WheelSpeedState_3_BCMA"
  BCM_COM_PROC_P20/113 -> V_BCM_COM_Wheel_Control_Speed_W34/1
  DTC170/1 -> BCM_COM_PROC_P20/170
  V_BCM_COM_BCP_PARK_OFF_SW_CMD_Conf_Flt/1 -> DTC170/1
  BCM_COM_PROC_P20/55 -> V_BCM_COM_RH_Regular_Brkg_Press_Cmd/1
  DTC169/1 -> BCM_COM_PROC_P20/169
  V_BCM_COM_BCP_PARK_OFF_SW_CMD_Acq/1 -> DTC169/1
  V_BCM_COM_RH_BTS_Unconf_Flt/1 -> DTC168/1
  DTC167/1 -> BCM_COM_PROC_P20/167
  V_BCM_COM_RH_BTS_Conf_Flt/1 -> DTC167/1
  DTC166/1 -> BCM_COM_PROC_P20/166
  V_BCM_COM_LH_BTS_Unconf_Flt/1 -> DTC166/1
  DTC165/1 -> BCM_COM_PROC_P20/165
  V_BCM_COM_ACCU_PT_Acq/1 -> DTC164/1
  BCM_COM_PROC_P20/486 -> v_BCM_COM_Braking_On_W12/1  "v_BCM_COM_Braking_On_W12_1_BCMA"
  DTC163/1 -> BCM_COM_PROC_P20/163
  V_BCM_COM_ACCU_PT_Unconf_Flt/1 -> DTC163/1
  DTC162/1 -> BCM_COM_PROC_P20/162
  V_BCM_COM_ACCU_PT_Conf_Flt/1 -> DTC162/1
  BCM_COM_PROC_P20/122 -> V_BCM_COM_Automate_State_W12/1
  DTC160/1 -> BCM_COM_PROC_P20/160
  V_BCM_COM_DBCU_ALT_MODE_Conf_Flt/1 -> DTC160/1
  DTC159/1 -> BCM_COM_PROC_P20/159
  V_BCM_COM_DBCU_FAILED_Unconf_Flt/1 -> DTC159/1
  V_BCM_COM_DBCU_FAILED_Conf_Flt/1 -> DTC158/1
  DTC157/1 -> BCM_COM_PROC_P20/157
  V_BCM_COM_RH_DBCU_BRK_CMD_FDBK_Unconf_Flt/1 -> DTC157/1
  BCM_COM_PROC_P20/268 -> V_BCM_COM_A429_RMLG_Inboard_Tire_Press/1
  BCM_COM_PROC_P20/556 -> Prb_SlowTrigCondition/1  "Prb_SlowTrigCondition_4_BCMA"
  DTC156/1 -> BCM_COM_PROC_P20/156
  V_BCM_COM_RH_DBCU_BRK_CMD_FDBK_Conf_Flt/1 -> DTC156/1
  DTC154/1 -> BCM_COM_PROC_P20/154
  V_BCM_COM_LH_DBCU_BRK_CMD_FDBK_Conf_Flt/1 -> DTC154/1
  BCM_COM_PROC_P20/393 -> V_BCM_COM_ETH_Braking_Norm_FT_Seq/1
  DTC225/1 -> BCM_COM_PROC_P20/225
  DTC153/1 -> BCM_COM_PROC_P20/153
  V_BCM_COM_DBCU_DISPATCH_SW_ON_Unconf_Flt/1 -> DTC153/1
  DTC152/1 -> BCM_COM_PROC_P20/152
  V_BCM_COM_DBCU_DISPATCH_SW_ON_Conf_Flt/1 -> DTC152/1
  DTC151/1 -> BCM_COM_PROC_P20/151
  V_BCM_COM_DBCU_BRK_ORDER_FAIL_Conf_Flt/1 -> DTC150/1
  DTC149/1 -> BCM_COM_PROC_P20/149
  V_BCM_COM_DBCU_ALT_MODE_Acq/1 -> DTC149/1
  DTC148/1 -> BCM_COM_PROC_P20/148
  V_BCM_COM_DBCU_FAILED_Acq/1 -> DTC148/1
  DTC147/1 -> BCM_COM_PROC_P20/147
  V_BCM_COM_LMLG_Inboard_Tire_Press_Acq/1 -> DTC183/1
  BCM_COM_PROC_P20/484 -> v_BCM_COM_Braking_On_W34/1  "v_BCM_COM_Braking_On_W34_1_BCMA"
  V_BCM_COM_RH_DBCU_BRK_CMD_FDBK_Acq/1 -> DTC147/1
  DTC146/1 -> BCM_COM_PROC_P20/146
  V_BCM_COM_LH_DBCU_BRK_CMD_FDBK_Acq/1 -> DTC146/1
  DTC145/1 -> BCM_COM_PROC_P20/145
  V_BCM_COM_DBCU_DISPATCH_SW_ON_Acq/1 -> DTC145/1
  BCM_COM_PROC_P20/229 -> V_BCM_COM_RMLG_Inboard_Tire_Press_Cons_Val/1
  BCM_COM_PROC_P20/288 -> V_BCM_COM_A429_Antiskid_Activity/1
  DTC144/1 -> BCM_COM_PROC_P20/144
  V_BCM_COM_CF_BSELV_JCL/1 -> DTC219/1
  DTC143/1 -> BCM_COM_PROC_P20/143
  V_BCM_COM_UTC_Time_Seconds_Unconf_Flt/1 -> DTC143/1
  DTC142/1 -> BCM_COM_PROC_P20/142
  V_BCM_COM_UTC_Time_Seconds_Conf_Flt/1 -> DTC142/1
  DTC141/1 -> BCM_COM_PROC_P20/141
  DTC140/1 -> BCM_COM_PROC_P20/140
  V_BCM_COM_UTC_Time_Minutes_Unconf_Flt/1 -> DTC140/1
  V_BCM_COM_UTC_Time_Minutes_Conf_Flt/1 -> DTC139/1
  DTC138/1 -> BCM_COM_PROC_P20/138
  V_BCM_COM_UTC_Time_Minutes_Acq/1 -> DTC138/1
  DTC137/1 -> BCM_COM_PROC_P20/137
  V_BCM_COM_UTC_Time_Hours_Unconf_Flt/1 -> DTC137/1
  DTC136/1 -> BCM_COM_PROC_P20/136
  DTC135/1 -> BCM_COM_PROC_P20/135
  BCM_COM_PROC_P20/292 -> V_BCM_COM_A429_ACCU_PT/1
  V_BCM_COM_LH_BTS_Conf_Flt/1 -> DTC165/1
  DTC134/1 -> BCM_COM_PROC_P20/134
  BCM_COM_PROC_P20/278 -> V_BCM_COM_A429_SSM_Avionics_Label_013/1
  DTC183/1 -> BCM_COM_PROC_P20/183
  DTC133/1 -> BCM_COM_PROC_P20/133
  DTC139/1 -> BCM_COM_PROC_P20/139
  V_BCM_COM_DFCS_A_TLA_Above_Idle_Acq_Val/1 -> DTC133/1
  BCM_COM_PROC_P20/364 -> V_BCM_COM_ETH_DBCU_Inhib_Order/1
  V_BCM_COM_DFCS_B_DBCU_ALT_Mode_2_Acq_Val/1 -> DTC132/1
  DTC131/1 -> BCM_COM_PROC_P20/131
  BCM_COM_PROC_P20/434 -> Prb_HydroplaneAccelProblem (1)/1  "Prb_HydroplaneAccelProblem_4_BCMA"
  V_BCM_COM_DFCS_B_DBCU_ALT_Mode_1_Acq_Val/1 -> DTC131/1
  DTC129/1 -> BCM_COM_PROC_P20/129
  DTC128/1 -> BCM_COM_PROC_P20/128
  V_BCM_COM_DFCS_A_DFCS_LH_Brkg_Cmd_Acq_Val/1 -> DTC128/1
  V_BCM_COM_CF_LH_SV_JOP/1 -> DTC224/1
  DTC127/1 -> BCM_COM_PROC_P20/127
  BCM_COM_PROC_P20/754 -> v_BCM_COM_MLG_Dnlk_State_Cons/1  "v_BCM_COM_MLG_Dnlk_State_Cons_1_BCMA"
  V_BCM_COM_DFCS_A_DFCS_RH_Brkg_Cmd_Acq_Val/1 -> DTC127/1
  DTC126/1 -> BCM_COM_PROC_P20/126
  BCM_COM_PROC_P20/309 -> V_BCM_COM_A429_PLT_Not_Performed/1
  V_BCM_COM_DFCS_B_DFCS_LH_Brkg_Cmd_Acq_Val/1 -> DTC126/1
  BCM_COM_PROC_P20/353 -> V_BCM_COM_ETH_PBSELV_ON_POS/1
  V_BCM_COM_DFCS_B_DFCS_RH_Brkg_Cmd_Acq_Val/1 -> DTC125/1
  BCM_COM_PROC_P20/331 -> V_BCM_COM_A429_Norm_Brake_Fail/1
  DTC124/1 -> BCM_COM_PROC_P20/124
  V_BCM_COM_DFCS_B_Wow_Val_3_Acq_Val/1 -> DTC124/1
  BCM_COM_PROC_P20/733 -> Prb_NaturalSmallSlipStep (3)/1  "Prb_NaturalSmallSlipStep_1_BCMA"
  V_BCM_COM_DFCS_B_Wow_Val_2_Acq_Val/1 -> DTC123/1
  DTC122/1 -> BCM_COM_PROC_P20/122
  BCM_COM_PROC_P20/255 -> V_BCM_COM_A429_SSM_DFCS_Label_102/1
  BCM_COM_PROC_P20/349 -> V_BCM_COM_ETH_BCP_BCM_ALT_SW_ON_CMD/1
  V_BCM_COM_DFCS_B_Wow_Val_1_Acq_Val/1 -> DTC122/1
  DTC121/1 -> BCM_COM_PROC_P20/121
  BCM_COM_PROC_P20/840 -> v_BCM_COM_UF_DFCS_B_DBCU_ALT_MODE_1_RX/1  "v_BCM_COM_UF_DFCS_B_DBCU_ALT_MODE_1_RX_1_BCMA"
  V_BCM_COM_DBCU_ALT_MODE_Unconf_Flt/1 -> DTC161/1
  V_BCM_COM_DFCS_B_Nlg_Wow_3_Acq_Val/1 -> DTC121/1
  DTC120/1 -> BCM_COM_PROC_P20/120
  V_BCM_COM_DFCS_A_DFCS_BCM_Caps_Val/1 -> DTC209/1
  V_BCM_COM_DFCS_B_Nlg_Wow_2_Acq_Val/1 -> DTC120/1
  DTC119/1 -> BCM_COM_PROC_P20/119
  BCM_COM_PROC_P20/248 -> V_BCM_COM_A429_TACHO_Fail_W12/1
  V_BCM_COM_DFCS_B_Rmlg_Wow_3_Acq_Val/1 -> DTC118/1
  DTC117/1 -> BCM_COM_PROC_P20/117
  V_BCM_COM_LH_DBCU_BRK_CMD_FDBK_Unconf_Flt/1 -> DTC155/1
  V_BCM_COM_DFCS_B_Rmlg_Wow_2_Acq_Val/1 -> DTC117/1
  BCM_COM_PROC_P20/683 -> Prb_AutomateState (2)/1  "Prb_AutomateState_2_BCMA"
  DTC189/1 -> BCM_COM_PROC_P20/189
  DTC116/1 -> BCM_COM_PROC_P20/116
  BCM_COM_PROC_P20/846 -> v_BCM_COM_UF_DFCS_A_TLA_ABOVE_IDLE_RX/1  "v_BCM_COM_UF_DFCS_A_TLA_ABOVE_IDLE_RX_1_BCMA"
  BCM_COM_PROC_P20/78 -> V_BCM_COM_RH_Press_Law_Brkg_Press_Cmd/1
  V_BCM_COM_DFCS_B_Rmlg_Wow_1_Acq_Val/1 -> DTC116/1
  BCM_COM_PROC_P20/241 -> V_BCM_COM_A429_SSM_Avionics_Label_041/1
  BCM_COM_PROC_P20/545 -> Prb_AsBrkLossTargetDecel/1  "Prb_AsBrkLossTargetDecel_4_BCMA"
  V_BCM_COM_DFCS_B_Lmlg_Wow_3_Acq_Val/1 -> DTC115/1
  BCM_COM_PROC_P20/254 -> V_BCM_COM_A429_SSM_DFCS_Label_101/1
  DTC114/1 -> BCM_COM_PROC_P20/114
  BCM_COM_PROC_P20/567 -> Prb_TransitionBigSlipStep/1  "Prb_TransitionBigSlipStep_4_BCMA"
  V_BCM_COM_DFCS_B_Nlg_Wow_1_Acq_Val/1 -> DTC119/1
  DTC229/1 -> BCM_COM_PROC_P20/229
  DTC112/1 -> BCM_COM_PROC_P20/112
  DTC111/1 -> BCM_COM_PROC_P20/111
  V_BCM_COM_DFCS_A_Wow_Val_2_Acq_Val/1 -> DTC111/1
  DTC110/1 -> BCM_COM_PROC_P20/110
  BCM_COM_PROC_P20/116 -> V_BCM_COM_Big_Slip_Trig_Out_W12/1
  V_BCM_COM_DBCU_BRK_ORDER_FAIL_Acq/1 -> DTC144/1
  BCM_COM_PROC_P20/312 -> V_BCM_COM_A429_LH_Brkg_Cmd_Fdbk/1
  V_BCM_COM_DFCS_A_Wow_Val_1_Acq_Val/1 -> DTC110/1
  DTC168/1 -> BCM_COM_PROC_P20/168
  DTC109/1 -> BCM_COM_PROC_P20/109
  BCM_COM_PROC_P20/720 -> Prb_FastTrigCondition (3)/1  "Prb_FastTrigCondition_1_BCMA"
  DTC108/1 -> BCM_COM_PROC_P20/108
  BCM_COM_PROC_P20/205 -> V_BCM_COM_DBCU_ALT_MODE_Cons/1
  DTC132/1 -> BCM_COM_PROC_P20/132
  DTC107/1 -> BCM_COM_PROC_P20/107
  DTC106/1 -> BCM_COM_PROC_P20/106
  BCM_COM_PROC_P20/657 -> Prb_ResearchModeCondition (2)/1  "Prb_ResearchModeCondition_2_BCMA"
  V_BCM_COM_LNLG_Tire_Press_Acq/1 -> DTC174/1
  BCM_COM_PROC_P20/265 -> V_BCM_COM_A429_RNLG_Tire_Press/1
  V_BCM_COM_DFCS_A_Rmlg_Wow_3_Acq_Val/1 -> DTC106/1
  BCM_COM_PROC_P20/668 -> Prb_NaturalBigSlipWatchDog (2)/1  "Prb_NaturalBigSlipWatchDog_2_BCMA"
  DTC105/1 -> BCM_COM_PROC_P20/105
  DTC104/1 -> BCM_COM_PROC_P20/104
  BCM_COM_PROC_P20/612 -> Prb_ForcedBigSlipWatchDog (1)/1  "Prb_ForcedBigSlipWatchDog_3_BCMA"
  BCM_COM_PROC_P20/15 -> V_BCM_COM_AC_Pitch_Ang_Filt/1
  DTC103/1 -> BCM_COM_PROC_P20/103
  V_BCM_COM_DFCS_A_Lmlg_Wow_3_Acq_Val/1 -> DTC103/1
  DTC102/1 -> BCM_COM_PROC_P20/102
  V_BCM_COM_UTC_Time_Seconds_Acq/1 -> DTC141/1
  BCM_COM_PROC_P20/126 -> V_BCM_COM_Target_Decel_Out_W12/1
  V_BCM_COM_DFCS_A_Lmlg_Wow_2_Acq_Val/1 -> DTC102/1
  BCM_COM_PROC_P20/690 -> Prb_DenAccuBigSlip (2)/1  "Prb_DenAccuBigSlip_2_BCMA"
  BCM_COM_PROC_P20/206 -> V_BCM_COM_DBCU_ALT_MODE_Cons_Val/1
  V_BCM_COM_DFCS_A_Lmlg_Wow_1_Acq_Val/1 -> DTC101/1
  DTC100/1 -> BCM_COM_PROC_P20/100
  DTC210/1 -> BCM_COM_PROC_P20/210
  V_BCM_COM_DFCS_B_Pitch_Angle_Acq_Val/1 -> DTC100/1
  V_BCM_COM_DFCS_B_Long_Accel_Acq_Val/1 -> DTC99/1
  DTC98/1 -> BCM_COM_PROC_P20/98
  BCM_COM_PROC_P20/774 -> v_BCM_COM_UF_DFCS_A_ACCEL_RX/1  "v_BCM_COM_UF_DFCS_A_ACCEL_RX_1_BCMA"
  BCM_COM_PROC_P20/92 -> V_BCM_COM_Disp_Sw_Cmd_Cons_Val/1
  DTC97/1 -> BCM_COM_PROC_P20/97
  BCM_COM_PROC_P20/27 -> V_BCM_COM_LMLG_On_Gnd_State_Val/1
  V_BCM_COM_DFCS_B_Decel_Law_Inhib_Acq_Val/1 -> DTC97/1
  BCM_COM_PROC_P20/727 -> Prb_BigGammaThreshold (3)/1  "Prb_BigGammaThreshold_1_BCMA"
  V_BCM_COM_RMLG_Inboard_Tire_Press_Conf_Flt/1 -> DTC187/1
  DTC95/1 -> BCM_COM_PROC_P20/95
  BCM_COM_PROC_P20/451 -> Prb_HydroplaneCondition (2)/1  "Prb_HydroplaneCondition_2_BCMA"
  V_BCM_COM_DFCS_A_Pitch_Angle_Acq_Val/1 -> DTC95/1
  DTC94/1 -> BCM_COM_PROC_P20/94
  V_BCM_COM_CF_RH_SV_OC/1 -> DTC200/1
  BCM_COM_PROC_P20/230 -> V_BCM_COM_RMLG_Outboard_Tire_Press_Cons/1
  BCM_COM_PROC_P20/717 -> Prb_SlowMonitoringCondition (3)/1  "Prb_SlowMonitoringCondition_1_BCMA"
  DTC123/1 -> BCM_COM_PROC_P20/123
  V_BCM_COM_DFCS_A_Long_Accel_Acq_Val/1 -> DTC94/1
  BCM_COM_PROC_P20/345 -> V_BCM_COM_ETH_ENG2_RUNNING/1
  DTC93/1 -> BCM_COM_PROC_P20/93
  V_BCM_COM_DFCS_A_Nlg_Wow_3_Acq_Val/1 -> DTC109/1
  DTC92/1 -> BCM_COM_PROC_P20/92
  DTC223/1 -> BCM_COM_PROC_P20/223
  BCM_COM_PROC_P20/608 -> Prb_FastStateCondition (1)/1  "Prb_FastStateCondition_3_BCMA"
  V_BCM_COM_Hyd_B_Press_Acq_Val/1 -> DTC92/1
  BCM_COM_PROC_P20/217 -> V_BCM_COM_MP_MAINT_MODE_CMD_28V_Conf/1
  DTC89/1 -> BCM_COM_PROC_P20/89
  DTC125/1 -> BCM_COM_PROC_P20/125
  DTC88/1 -> BCM_COM_PROC_P20/88
  V_BCM_COM_BCM_DBCU_INHIBITION_Acq/1 -> DTC88/1
  DTC87/1 -> BCM_COM_PROC_P20/87
  V_BCM_COM_LMLG_Outboard_Tire_Press_Conf_Flt/1 -> DTC181/1
  V_BCM_COM_BCM_DBCU_INHIBITION_Unconf_Flt/1 -> DTC87/1
  BCM_COM_PROC_P20/18 -> V_BCM_COM_DFCS_B_WOWs_Val_Cons/1
  V_BCM_COM_BCM_DBCU_INHIBITION_Conf_Flt/1 -> DTC86/1
  BCM_COM_PROC_P20/247 -> V_BCM_COM_A429_Wheel_Speed_W34/1
  DTC85/1 -> BCM_COM_PROC_P20/85
  V_BCM_COM_UTC_Time_Hours_Conf_Flt/1 -> DTC136/1
  BCM_COM_PROC_P20/65 -> V_BCM_COM_Start_Norm_FT_Cond/1
  V_BCM_COM_Big_Slip_Trig_In_Acq_W34/1 -> DTC85/1
  BCM_COM_PROC_P20/685 -> Prb_TargetSpeedDelta (2)/1  "Prb_TargetSpeedDelta_2_BCMA"
  BCM_COM_PROC_P20/108 -> V_BCM_COM_Hyd_B_Press_Cons_Val/1
  DTC84/1 -> BCM_COM_PROC_P20/84
  V_BCM_COM_Big_Slip_Trig_In_Acq_W12/1 -> DTC84/1
  BCM_COM_PROC_P20/98 -> V_BCM_COM_Braking_Type/1
  V_BCM_COM_Small_Slip_Trig_In_Acq_W34/1 -> DTC83/1
  BCM_COM_PROC_P20/820 -> v_BCM_COM_UF_DFCS_B_VALWOW_2_RX/1  "v_BCM_COM_UF_DFCS_B_VALWOW_2_RX_1_BCMA"
  DTC164/1 -> BCM_COM_PROC_P20/164
  DTC82/1 -> BCM_COM_PROC_P20/82
  BCM_COM_PROC_P20/604 -> Prb_TransitionAntiskidBrakeLoss (1)/1  "Prb_TransitionAntiskidBrakeLoss_3_BCMA"
  BCM_COM_PROC_P20/97 -> V_BCM_COM_Alt_Brkg_Availability/1
  BCM_COM_PROC_P20/580 -> Prb_DenAccuBigSlip/1  "Prb_DenAccuBigSlip_4_BCMA"
  V_BCM_COM_DFCS_A_Decel_Law_Inhib_Acq_Val/1 -> DTC96/1
  V_BCM_COM_Small_Slip_Trig_In_Acq_W12/1 -> DTC82/1
  DTC211/1 -> BCM_COM_PROC_P20/211
  V_BCM_COM_Big_Gamma_Trig_In_Acq_W34/1 -> DTC81/1
  DTC80/1 -> BCM_COM_PROC_P20/80
  BCM_COM_PROC_P20/565 -> Prb_ForcedBigSlipStep/1  "Prb_ForcedBigSlipStep_4_BCMA"
  BCM_COM_PROC_P20/228 -> V_BCM_COM_RMLG_Inboard_Tire_Press_Cons/1
  V_BCM_COM_UTC_Time_Hours_Acq/1 -> DTC135/1
  BCM_COM_PROC_P20/816 -> v_BCM_COM_CF_DFCS_B_VALWOW_3_RX/1  "v_BCM_COM_CF_DFCS_B_VALWOW_3_RX_1_BCMA"
  DTC79/1 -> BCM_COM_PROC_P20/79
  DTC81/1 -> BCM_COM_PROC_P20/81
  V_BCM_COM_Big_Slip_WD_Trig_In_Acq_W34/1 -> DTC79/1
  V_BCM_COM_Big_Slip_WD_Trig_In_Acq_W12/1 -> DTC78/1
  BCM_COM_PROC_P20/689 -> Prb_WheelSkidSmoothAverage (2)/1  "Prb_WheelSkidSmoothAverage_2_BCMA"
  DTC115/1 -> BCM_COM_PROC_P20/115
  DTC77/1 -> BCM_COM_PROC_P20/77
  BCM_COM_PROC_P20/643 -> Prb_AsLowPassTheorCurrent (2)/1  "Prb_AsLowPassTheorCurrent_2_BCMA"
  V_BCM_COM_Target_Speed_In_Acq_W34/1 -> DTC77/1
  BCM_COM_PROC_P20/118 -> V_BCM_COM_Big_Slip_WD_Trig_Out_W12/1
  DTC76/1 -> BCM_COM_PROC_P20/76
  BCM_COM_PROC_P20/171 -> V_BCM_COM_DFCS_B_NLG_WOWs_Val/1
  V_BCM_COM_Target_Speed_In_Acq_W12/1 -> DTC76/1
  BCM_COM_PROC_P20/630 -> Prb_TargetSpeedDelta (1)/1  "Prb_TargetSpeedDelta_3_BCMA"
  BCM_COM_PROC_P20/73 -> V_BCM_COM_Start_Alt_FT_Cond/1
  DTC75/1 -> BCM_COM_PROC_P20/75
  BCM_COM_PROC_P20/425 -> Prb_BrakingPhaseAcceleration/1  "Prb_BrakingPhaseAcceleration_5_BCMA"
  DTC74/1 -> BCM_COM_PROC_P20/74
  DTC227/1 -> BCM_COM_PROC_P20/227
  V_BCM_COM_DFCS_A_Gnd_Spd_Acq_Val/1 -> DTC93/1
  V_BCM_COM_Opt_Adhesion_In_Acq_W12/1 -> DTC74/1
  DTC72/1 -> BCM_COM_PROC_P20/72
  V_BCM_COM_Big_Gamma_Trig_In_Acq_W12/1 -> DTC80/1
  V_BCM_COM_Adhesion_In_Acq_W12/1 -> DTC72/1
  BCM_COM_PROC_P20/375 -> V_BCM_COM_ETH_FB_HYD_A_LOW_PRESS/1
  V_BCM_COM_BCM_CCDL_Unconf_Flt/1 -> DTC71/1
  DTC86/1 -> BCM_COM_PROC_P20/86
  DTC70/1 -> BCM_COM_PROC_P20/70
  V_BCM_COM_BCM_CCDL_Conf_Flt/1 -> DTC70/1
  DTC69/1 -> BCM_COM_PROC_P20/69
  BCM_COM_PROC_P20/111 -> V_BCM_COM_Sys_Sanc_Inhib_During_FT/1
  V_BCM_COM_SV_PT_Cons_Val/1 -> DTC69/1
  BCM_COM_PROC_P20/46 -> V_BCM_COM_RMLG_Downlock_State/1
  V_BCM_COM_SV_Current/1 -> DTC68/1
  BCM_COM_PROC_P20/823 -> v_BCM_COM_UF_DFCS_B_RMLGWOW_2_RX/1  "v_BCM_COM_UF_DFCS_B_RMLGWOW_2_RX_1_BCMA"
  DTC67/1 -> BCM_COM_PROC_P20/67
  BCM_COM_PROC_P20/76 -> V_BCM_COM_RH_Press_Reg_FT_Act_Cond/1
  V_BCM_COM_Whl_LP_AS_Curr_Order_W34/1 -> DTC67/1
  V_BCM_COM_LMLG_Inboard_Tire_Press_Conf_Flt/1 -> DTC184/1
  BCM_COM_PROC_P20/501 -> Prb_HydroplaneAcceleration (4)/1  "Prb_HydroplaneAcceleration_1_BCMA"
  DTC65/1 -> BCM_COM_PROC_P20/65
  V_BCM_COM_Wheel_Speed_Error_W34/1 -> DTC65/1
  BCM_COM_PROC_P20/570 -> Prb_TransitionSmallSlipStep/1  "Prb_TransitionSmallSlipStep_4_BCMA"
  V_BCM_COM_PPRG_Fault/1 -> DTC213/1
  DTC64/1 -> BCM_COM_PROC_P20/64
  DTC101/1 -> BCM_COM_PROC_P20/101
  V_BCM_COM_Wheel_Speed_Error_W12/1 -> DTC64/1
  DTC63/1 -> BCM_COM_PROC_P20/63
  BCM_COM_PROC_P20/448 -> Prb_HydroplaneTransition (2)/1  "Prb_HydroplaneTransition_3_BCMA"
  V_BCM_COM_Wheel_Filtered_Speed_W34/1 -> DTC63/1
  BCM_COM_PROC_P20/324 -> V_BCM_COM_A429_Pinprog_5/1
  DTC62/1 -> BCM_COM_PROC_P20/62
  V_BCM_COM_Wheel_Filtered_Speed_W12/1 -> DTC62/1
  DTC61/1 -> BCM_COM_PROC_P20/61
  V_BCM_COM_SV_PT_Cons/1 -> DTC61/1
  BCM_COM_PROC_P20/560 -> Prb_ForcedBigGammaStep/1  "Prb_ForcedBigGammaStep_4_BCMA"
  DTC60/1 -> BCM_COM_PROC_P20/60
  BCM_COM_PROC_P20/71 -> V_BCM_COM_Braking_Alt_FT_Seq/1
  BCM_COM_PROC_P20/390 -> V_BCM_COM_ETH_AC_State/1
  V_BCM_COM_Whl_LP_AS_Curr_Order/1 -> DTC60/1
  BCM_COM_PROC_P20/618 -> Prb_TransitionBigGammaStep (1)/1  "Prb_TransitionBigGammaStep_3_BCMA"
  DTC59/1 -> BCM_COM_PROC_P20/59
  BCM_COM_PROC_P20/680 -> Prb_TransitionSmallSlipStep (2)/1  "Prb_TransitionSmallSlipStep_2_BCMA"
  DTC226/1 -> BCM_COM_PROC_P20/226
  V_BCM_COM_Whl_AS_Inhib_Cond_W34/1 -> DTC59/1
  V_BCM_COM_Whl_AS_Inhib_Cond_W12/1 -> DTC58/1
  BCM_COM_PROC_P20/100 -> V_BCM_COM_Brkg_On_Wheels/1
  DTC57/1 -> BCM_COM_PROC_P20/57
  V_BCM_COM_Hyd_B_Press_Acq/1 -> DTC57/1
  BCM_COM_PROC_P20/338 -> V_BCM_COM_A429_DBCU_Inhib_Opp_Side/1
  DTC56/1 -> BCM_COM_PROC_P20/56
  BCM_COM_PROC_P20/429 -> Prb_Previous_ReferenceSpeed/1  "Prb_Previous_ReferenceSpeed_4_BCMA"
  V_BCM_COM_Hyd_A_Press_Acq/1 -> DTC56/1
  BCM_COM_PROC_P20/407 -> V_BCM_COM_ETH_TT_completed/1
  DTC55/1 -> BCM_COM_PROC_P20/55
  BCM_COM_PROC_P20/659 -> Prb_TransitionAntiskidBrakeLoss (2)/1  "Prb_TransitionAntiskidBrakeLoss_2_BCMA"
  DTC53/1 -> BCM_COM_PROC_P20/53
  V_BCM_COM_PBSELV_ON_POS_Acq/1 -> DTC53/1
  BCM_COM_PROC_P20/528 -> v_BCM_COM_Hyd_Press_State/1  "v_BCM_COM_Hyd_Press_State_1_BCMA"
  DTC52/1 -> BCM_COM_PROC_P20/52
  V_BCM_COM_SV_PT_Filt/1 -> DTC52/1
  V_BCM_COM_Adhesion_In_Acq_W34/1 -> DTC73/1
  BCM_COM_PROC_P20/207 -> V_BCM_COM_ACCU_PT_Cons/1
  DTC51/1 -> BCM_COM_PROC_P20/51
  BCM_COM_PROC_P20/256 -> V_BCM_COM_A429_SSM_DFCS_Label_103/1
  DTC91/1 -> BCM_COM_PROC_P20/91
  V_BCM_COM_CF_RH_ALT_BRK_LOSS/1 -> DTC51/1
  BCM_COM_PROC_P20/225 -> V_BCM_COM_LMLG_Outboard_Tire_Press_Cons_Val/1
  DTC113/1 -> BCM_COM_PROC_P20/113
  BCM_COM_PROC_P20/646 -> Prb_AdhesionOpt (2)/1  "Prb_AdhesionOpt_2_BCMA"
  DTC50/1 -> BCM_COM_PROC_P20/50
  DTC49/1 -> BCM_COM_PROC_P20/49
  DTC58/1 -> BCM_COM_PROC_P20/58
  BCM_COM_PROC_P20/130 -> V_BCM_COM_Opt_Adhesion_Out_W12/1
  BCM_COM_PROC_P20/412 -> Prb_HydroplaneTransition/1  "Prb_HydroplaneTransition_5_BCMA"
  V_BCM_COM_CF_LH_ALT_BRK_LOSS/1 -> DTC49/1
  DTC48/1 -> BCM_COM_PROC_P20/48
  DTC54/1 -> BCM_COM_PROC_P20/54
  DTC47/1 -> BCM_COM_PROC_P20/47
  BCM_COM_PROC_P20/512 -> Prb_WheelSpeedState (4)/1  "Prb_WheelSpeedState_1_BCMA"
  DTC198/1 -> BCM_COM_PROC_P20/198
  V_BCM_COM_Antiskid_Off_Sanction/1 -> DTC47/1
  DTC99/1 -> BCM_COM_PROC_P20/99
  DTC46/1 -> BCM_COM_PROC_P20/46
  V_BCM_COM_MP_BCMA_Alt_Disp_Sw_Acq/1 -> DTC46/1
  BCM_COM_PROC_P20/49 -> V_BCM_COM_SELV_Low_Speed_Logic/1
  DTC45/1 -> BCM_COM_PROC_P20/45
  V_BCM_COM_DFCS_B_TLA_Above_Idle_Acq_Val/1 -> DTC134/1
  BCM_COM_PROC_P20/780 -> v_BCM_COM_UF_DFCS_B_PITCH_RX/1  "v_BCM_COM_UF_DFCS_B_PITCH_RX_1_BCMA"
  V_BCM_COM_MP_BCMA_Alt_Disp_Sw_Unconf_Flt/1 -> DTC45/1
  BCM_COM_PROC_P20/36 -> V_BCM_COM_Decel_Law_Inhib_Cons_Val/1
  DTC44/1 -> BCM_COM_PROC_P20/44
  BCM_COM_PROC_P20/372 -> V_BCM_COM_ETH_FB_DBCU_FAIL/1
  V_BCM_COM_MP_BCMA_Alt_Disp_Sw_Conf_Flt/1 -> DTC44/1
  V_BCM_COM_DBCU_BRK_ORDER_FAIL_Unconf_Flt/1 -> DTC151/1
  DTC43/1 -> BCM_COM_PROC_P20/43
  BCM_COM_PROC_P20/172 -> V_BCM_COM_DFCS_B_WOWs_Val_Val/1
  BCM_COM_PROC_P20/760 -> v_BCM_COM_UF_HYD_A_PRESS_RX/1  "v_BCM_COM_UF_HYD_A_PRESS_RX_1_BCMA"
  V_BCM_COM_BCP_BCM_Alt_Sw_On_Cmd_Unconf_Flt/1 -> DTC43/1
  DTC42/1 -> BCM_COM_PROC_P20/42
  DTC130/1 -> BCM_COM_PROC_P20/130
  V_BCM_COM_BCP_BCM_Alt_Sw_On_Cmd_Conf_Flt/1 -> DTC42/1
  V_BCM_COM_DFCS_A_DBCU_ALT_Mode_1_Acq_Val/1 -> DTC129/1
  DTC41/1 -> BCM_COM_PROC_P20/41
  V_BCM_COM_BCP_BCM_Alt_Sw_On_Cmd_Acq/1 -> DTC41/1
  BCM_COM_PROC_P20/645 -> Prb_Adhesion (2)/1  "Prb_Adhesion_2_BCMA"
  V_BCM_COM_DFCS_A_DBCU_ALT_Mode_2_Acq_Val/1 -> DTC130/1
  DTC40/1 -> BCM_COM_PROC_P20/40
  DTC71/1 -> BCM_COM_PROC_P20/71
  BCM_COM_PROC_P20/204 -> V_BCM_COM_DBCU_FAILED_Cons_Val/1
  V_BCM_COM_BCM_Validity_By_SP/1 -> DTC40/1
  V_BCM_COM_DFCS_A_Nlg_Wow_2_Acq_Val/1 -> DTC108/1
  V_BCM_COM_Engine_2_Running_Acq_Val/1 -> DTC90/1
  BCM_COM_PROC_P20/705 -> Prb_SoftSpeedCounter (3)/1  "Prb_SoftSpeedCounter_1_BCMA"
  DTC39/1 -> BCM_COM_PROC_P20/39
  V_BCM_COM_BCM_Off_Sanction/1 -> DTC39/1
  DTC161/1 -> BCM_COM_PROC_P20/161
  DTC38/1 -> BCM_COM_PROC_P20/38
  V_BCM_COM_BCM_Config/1 -> DTC38/1
  BCM_COM_PROC_P20/180 -> V_BCM_COM_DFCS_B_DBCU_Alt_Mode_2_Val/1
  DTC37/1 -> BCM_COM_PROC_P20/37
  BCM_COM_PROC_P20/151 -> V_BCM_COM_Engine_Running_Conf_Flt/1
  BCM_COM_PROC_P20/829 -> v_BCM_COM_UF_DFCS_B_LMLGWOW_2_RX/1  "v_BCM_COM_UF_DFCS_B_LMLGWOW_2_RX_1_BCMA"
  V_BCM_COM_Maint_Itv_Function_Req/1 -> DTC37/1
  DTC36/1 -> BCM_COM_PROC_P20/36
  BCM_COM_PROC_P20/323 -> V_BCM_COM_A429_Pinprog_4/1
  DTC118/1 -> BCM_COM_PROC_P20/118
  V_BCM_COM_Engine_Running_Acq/1 -> DTC36/1
  DTC35/1 -> BCM_COM_PROC_P20/35
  BCM_COM_PROC_P20/313 -> V_BCM_COM_A429_RH_Brkg_Cmd_Fdbk/1
  V_BCM_COM_DFCS_B_Lmlg_Wow_1_Acq_Val/1 -> DTC113/1
  V_BCM_COM_RMLG_Dnlk_Conf_Flt/1 -> DTC35/1
  DTC34/1 -> BCM_COM_PROC_P20/34
  BCM_COM_PROC_P20/593 -> Prb_BigGammaStepSize (1)/1  "Prb_BigGammaStepSize_3_BCMA"
  V_BCM_COM_Hyd_A_Press_Acq_Val/1 -> DTC91/1
  BCM_COM_PROC_P20/183 -> V_BCM_COM_UTC_Time_Hours_Cons/1
  V_BCM_COM_DFCS_B_Lmlg_Wow_2_Acq_Val/1 -> DTC114/1
  V_BCM_COM_RMLG_Dnlk_Unconf_Flt/1 -> DTC34/1
  V_BCM_COM_DFCS_A_Rmlg_Wow_2_Acq_Val/1 -> DTC105/1
  DTC33/1 -> BCM_COM_PROC_P20/33
  V_BCM_COM_LH_SV_PT_Conf_Flt/1 -> DTC221/1
  DTC31/1 -> BCM_COM_PROC_P20/31
  V_BCM_COM_DFCS_A_Wow_Val_3_Acq_Val/1 -> DTC112/1
  BCM_COM_PROC_P20/809 -> v_BCM_COM_CF_DFCS_B_LMLGWOW_3_RX/1  "v_BCM_COM_CF_DFCS_B_LMLGWOW_3_RX_1_BCMA"
  V_BCM_COM_LMLG_Dnlk_Conf_Flt/1 -> DTC33/1
  V_BCM_COM_RMLG_Downlock_Acq/1 -> DTC31/1
  BCM_COM_PROC_P20/41 -> V_BCM_COM_LG_Lever_Ste_Cons_Val/1
  DTC30/1 -> BCM_COM_PROC_P20/30
  DTC28/1 -> BCM_COM_PROC_P20/28
  V_BCM_COM_DFCS_A_Nlg_Wow_1_Acq_Val/1 -> DTC107/1
  BCM_COM_PROC_P20/120 -> V_BCM_COM_Small_Slip_Trig_Out_W12/1
  V_BCM_COM_LG_Lever_Up_Acq/1 -> DTC27/1
  V_BCM_COM_DFCS_B_Gnd_Spd_Acq_Val/1 -> DTC98/1
  BCM_COM_PROC_P20/258 -> V_BCM_COM_A429_LH_Brake_Temp/1
  BCM_COM_PROC_P20/763 -> v_BCM_COM_CF_DFCS_B_RH_BRK_CMD_RX/1  "v_BCM_COM_CF_DFCS_B_RH_BRK_CMD_RX_1_BCMA"
  V_BCM_COM_DFCS_B_TLA_Above_Idle_Acq/1 -> DTC26/1
  V_BCM_COM_CF_SELV_SC/1 -> DTC201/1
  BCM_COM_PROC_P20/747 -> Prb_TargetOverDecelInteg (3)/1  "Prb_TargetOverDecelInteg_1_BCMA"
  DTC24/1 -> BCM_COM_PROC_P20/24
  BCM_COM_PROC_P20/540 -> Prb_SoftSpeedCounter/1  "Prb_SoftSpeedCounter_4_BCMA"
  V_BCM_COM_DFCS_B_Decel_Law_Inhib_Acq/1 -> DTC24/1
  BCM_COM_PROC_P20/625 -> Prb_TransitionSmallSlipStep (1)/1  "Prb_TransitionSmallSlipStep_3_BCMA"
  DTC96/1 -> BCM_COM_PROC_P20/96
  V_BCM_COM_DFCS_A_Decel_Law_Inhib_Acq/1 -> DTC23/1
  DTC23/1 -> BCM_COM_PROC_P20/23
  BCM_COM_PROC_P20/737 -> Prb_TransitionGammaIncrease (3)/1  "Prb_TransitionGammaIncrease_1_BCMA"
  DTC21/1 -> BCM_COM_PROC_P20/21
  BCM_COM_PROC_P20/655 -> Prb_AsBrkLossTargetDecel (2)/1  "Prb_AsBrkLossTargetDecel_2_BCMA"
  V_BCM_COM_DFCS_B_DFCS_RH_Braking_Cmd_Acq/1 -> DTC22/1
  DTC212/1 -> BCM_COM_PROC_P20/212
  V_BCM_COM_LG_Lever_Up_Unconf_Flt/1 -> DTC28/1
  BCM_COM_PROC_P20/33 -> V_BCM_COM_LH_Braking_Cmd_Cons/1
  V_BCM_COM_DFCS_B_DFCS_LH_Braking_Cmd_Acq/1 -> DTC21/1
  BCM_COM_PROC_P20/600 -> Prb_AsBrkLossTargetDecel (1)/1  "Prb_AsBrkLossTargetDecel_3_BCMA"
  BCM_COM_PROC_P20/588 -> Prb_AsLowPassTheorCurrent (1)/1  "Prb_AsLowPassTheorCurrent_3_BCMA"
  DTC20/1 -> BCM_COM_PROC_P20/20
  V_BCM_COM_DFCS_A_DFCS_RH_Braking_Cmd_Acq/1 -> DTC20/1
  DTC25/1 -> BCM_COM_PROC_P20/25
  V_BCM_COM_Engine_1_Running_Acq_Val/1 -> DTC89/1
  V_BCM_COM_DFCS_A_DFCS_LH_Braking_Cmd_Acq/1 -> DTC19/1
  DTC83/1 -> BCM_COM_PROC_P20/83
  BCM_COM_PROC_P20/174 -> V_BCM_COM_DFCS_A_RH_Braking_Cmd_Val/1
  BCM_COM_PROC_P20/411 -> V_BCM_COM_Decel_Ctrl_Loop_Act_Cond/1
  DTC18/1 -> BCM_COM_PROC_P20/18
  BCM_COM_PROC_P20/294 -> V_BCM_COM_A429_SELV_Disc_Sts_Rdbk_Val/1
  V_BCM_COM_LH_Decel_Law_Brkg_Press_Cmd/1 -> DTC18/1
  BCM_COM_PROC_P20/640 -> Prb_TheorCommandedPressure (2)/1  "Prb_TheorCommandedPressure_2_BCMA"
  DTC17/1 -> BCM_COM_PROC_P20/17
  V_BCM_COM_RH_Decel_Law_Brkg_Press_Cmd/1 -> DTC17/1
  BCM_COM_PROC_P20/296 -> V_BCM_COM_A429_SSM_Avionics_Label_020/1
  V_BCM_COM_DFCS_A_Rmlg_Wow_1_Acq_Val/1 -> DTC104/1
  BCM_COM_PROC_P20/280 -> V_BCM_COM_A429_SSM_Avionics_Label_015/1
  DTC16/1 -> BCM_COM_PROC_P20/16
  DTC78/1 -> BCM_COM_PROC_P20/78
